simulink model "SimulinkAnalysisofCheetahTail"  (R2022a)
settings: Solver=ode4  StartTime=0.0  StopTime=1.5  FixedStep=0.001  RelTol=1e-3
undefined symbols (not defined in the file): B_cg_H, B_con_H, B_con_L, bar_len, cd_table, Cf, cl_table, g, gear_ratio, int_point_bar, int_point_tail, ITail, M_add, M_cg_H, M_cg_L, M_cg_W, Mb, Mm, Mt, psi3, rho, T_cg_H, T_fur_gap, T_length, T_width_major, T_width_minor, th2_initial, torque_constant, uncertainty_Forces, uncertainty_Position, Vf, windspeed
(part 2 of 21)

== matlab function SimulinkAnalysisofCheetahTail/Model/CoriolusMatrix ==
  data: B_cg_H parameter; B_con_H parameter; B_con_L parameter; ITail parameter; M_cg_H parameter; M_cg_L parameter; M_cg_W parameter; Mb parameter; Mm parameter; Mt parameter; T_cg_H parameter; C output; q input; dq input
function C = CoriolusMatrix(B_cg_H,B_con_H,B_con_L,ITail,M_cg_H,M_cg_L,M_cg_W,Mb,Mm,Mt,T_cg_H,q,dq)
%#codegen
[x,y,z,phi1,th1,psi1,phi2,th2] = deal(q(1),q(2),q(3),q(4),q(5),q(6),q(7),q(8));
[dx,dy,dz,dphi1,dth1,dpsi1,dphi2,dth2] = deal(dq(1),dq(2),dq(3),dq(4),dq(5),dq(6),dq(7),dq(8));
%    This function was generated by the Symbolic Math Toolbox version 9.0.
%    26-Jan-2022 10:41:54

t2 = cos(phi1);
t3 = cos(phi2);
t4 = cos(psi1);
t5 = cos(th1);
t6 = cos(th2);
t7 = sin(phi1);
t8 = sin(phi2);
t9 = sin(psi1);
t10 = sin(th1);
t11 = sin(th2);
t12 = M_cg_L+x;
t13 = M_cg_W+y;
t14 = M_cg_H+z;
t15 = B_cg_H.^2;
t1314 = dphi1.*1.8563e-7;
t1336 = dphi1.*2.3495e-8;
t16 = t2.^2;
t17 = t4.^2;
t18 = t5.^2;
t19 = t7.^2;
t20 = t9.^2;
t21 = t10.^2;
t22 = B_con_L.*t5;
t23 = B_con_L.*t10;
t24 = dth1.*t2;
t25 = dx.*t5;
t26 = dth1.*t7;
t27 = dpsi1.*t10;
t28 = dx.*t10;
t29 = t2.*t3;
t30 = t2.*t4;
t31 = t5.*t6;
t32 = t2.*t8;
t33 = t2.*t9;
t34 = t4.*t7;
t35 = t5.*t11;
t36 = t6.*t10;
t37 = t7.*t8;
t38 = t7.*t9;
t39 = t10.*t11;
t40 = B_con_H.*t2.*t5;
t42 = t5.*t12;
t43 = B_con_H.*t2.*t10;
t44 = B_con_H.*t5.*t7;
t47 = t10.*t12;
t48 = Mb.*t5.*t10;
t49 = Mm.*t5.*t10;
t50 = Mt.*t5.*t10;
t51 = B_con_H.*t7.*t10;
t53 = dphi1.*t2.*t5;
t54 = dpsi1.*t2.*t5;
t56 = dy.*t2.*t5;
t57 = dz.*t2.*t5;
t58 = dpsi1.*t4.*t5;
t60 = dphi1.*t5.*t7;
t61 = dpsi1.*t5.*t7;
t63 = dy.*t5.*t7;
t64 = dz.*t2.*t10;
t65 = dz.*t5.*t7;
t66 = dpsi1.*t5.*t9;
t67 = dth1.*t4.*t10;
t71 = dy.*t7.*t10;
t72 = dth1.*t9.*t10;
t93 = t3.*t5.*t7;
t94 = t3.*t6.*t7;
t107 = t3.*t7.*t10;
t117 = t2.*t5.*t13;
t121 = t2.*t5.*t14;
t127 = t2.*t10.*t13;
t128 = t5.*t7.*t13;
t131 = t2.*t10.*t14;
t132 = t5.*t7.*t14;
t139 = t7.*t10.*t13;
t140 = t7.*t10.*t14;
t1196 = t5.*7.84867146e-3;
t1215 = t2.*1.19846373e-3;
t1223 = t7.*1.19846373e-3;
t1233 = t2.*3.949132625e-3;
t1234 = t7.*3.949132625e-3;
t1252 = t2.*1.0208097e-4;
t1253 = t7.*1.0208097e-4;
t1315 = t5.*t7.*(-1.19846373e-3);
t1343 = t2.*1.8563e-7;
t1344 = t2.*3.7126e-7;
t1345 = t5.*1.8563e-7;
t1346 = t7.*1.8563e-7;
t1347 = t10.*1.8563e-7;
t1348 = t7.*4.699e-8;
t1353 = t5.*t7.*(-1.0208097e-4);
t1370 = t2.*2.3495e-8;
t1371 = t5.*2.3495e-8;
t1374 = t7.*2.3495e-8;
t1375 = t10.*2.3495e-8;
t1391 = t2.*t5.*4.699e-8;
t1393 = t5.*t7.*3.7126e-7;
t1433 = t2.*t10.*(-3.7126e-7);
t41 = t4.*t22;
t45 = t4.*t23;
t46 = t9.*t22;
t52 = t9.*t23;
t55 = dphi1+t27;
t59 = t4.*t25;
t62 = t10.*t24;
t68 = t4.*t28;
t69 = t9.*t25;
t70 = t10.*t26;
t73 = t9.*t28;
t74 = t2.*t39;
t75 = t3.*t39;
t76 = t8.*t35;
t77 = t8.*t36;
t78 = t4.*t39;
t79 = t9.*t35;
t80 = t9.*t36;
t81 = t10.*t37;
t82 = t10.*t38;
t83 = t11.*t38;
t84 = t8.*t39;
t85 = t9.*t39;
t86 = t5.*t29;
t87 = t6.*t29;
t88 = t2.*t31;
t89 = t3.*t31;
t90 = t4.*t31;
t91 = t10.*t29;
t92 = t5.*t32;
t95 = t10.*t30;
t96 = t11.*t30;
t97 = t6.*t34;
t98 = t2.*t35;
t99 = t2.*t36;
t100 = t3.*t35;
t101 = t3.*t36;
t102 = t8.*t31;
t103 = t4.*t35;
t104 = t4.*t36;
t105 = t9.*t31;
t106 = t10.*t32;
t108 = t5.*t37;
t109 = t6.*t37;
t110 = t10.*t33;
t111 = t10.*t34;
t112 = t11.*t33;
t113 = t11.*t34;
t114 = t6.*t38;
t115 = B_con_H.*t5.*t30;
t116 = t4.*t42;
t119 = B_con_H.*t5.*t33;
t120 = B_con_H.*t5.*t34;
t122 = t4.*t47;
t123 = t9.*t42;
t124 = t2.*t48;
t125 = t2.*t49;
t126 = t2.*t50;
t130 = B_con_H.*t5.*t38;
t133 = t4.*t5.*t24;
t134 = dz.*t5.*t30;
t135 = t9.*t47;
t136 = t7.*t48;
t137 = t7.*t49;
t138 = t7.*t50;
t141 = t5.*t9.*t24;
t142 = t4.*t5.*t26;
t143 = dy.*t5.*t34;
t144 = dz.*t5.*t33;
t146 = dphi1.*t7.*t31;
t147 = dth2.*t7.*t31;
t148 = -t43;
t149 = -t44;
t150 = t5.*t9.*t26;
t151 = dy.*t5.*t38;
t152 = dphi1.*t7.*t35;
t153 = -t48;
t154 = -t49;
t155 = -t50;
t156 = -t51;
t157 = dphi1.*t7.*t39;
t158 = t26.*t39;
t159 = -t61;
t160 = -t63;
t161 = -t64;
t164 = -t72;
t165 = Mb.*t2.*t18;
t166 = Mm.*t2.*t18;
t167 = Mt.*t2.*t18;
t168 = Mb.*t2.*t21;
t169 = Mb.*t7.*t18;
t170 = Mm.*t2.*t21;
t171 = Mm.*t7.*t18;
t172 = Mt.*t2.*t21;
t173 = Mt.*t7.*t18;
t174 = Mb.*t7.*t21;
t175 = Mm.*t7.*t21;
t176 = Mt.*t7.*t21;
t182 = t29.*t31;
t183 = t30.*t31;
t186 = t5.*t8.*t30;
t187 = t3.*t5.*t34;
t188 = t29.*t35;
t189 = t29.*t36;
t190 = t31.*t32;
t192 = t30.*t35;
t193 = t30.*t36;
t194 = t31.*t33;
t200 = t3.*t5.*t38;
t201 = t5.*t8.*t34;
t202 = t29.*t39;
t203 = t32.*t35;
t204 = t32.*t36;
t206 = t31.*t37;
t207 = t30.*t39;
t208 = t33.*t35;
t209 = t33.*t36;
t219 = t32.*t39;
t220 = t36.*t37;
t221 = t33.*t39;
t222 = t34.*t39;
t230 = t38.*t39;
t234 = t5.*t13.*t30;
t235 = t5.*t14.*t30;
t236 = t5.*t13.*t33;
t237 = t5.*t13.*t34;
t239 = t5.*t14.*t33;
t240 = t5.*t14.*t34;
t241 = Mb.*t16.*t18;
t242 = Mm.*t16.*t18;
t243 = Mt.*t16.*t18;
t248 = t5.*t13.*t38;
t250 = t5.*t14.*t38;
t251 = Mb.*t18.*t19;
t252 = Mm.*t18.*t19;
t253 = Mt.*t18.*t19;
t255 = -t117;
t261 = dphi1.*t34.*t35;
t264 = -t127;
t265 = -t128;
t268 = -t131;
t269 = -t132;
t271 = dphi1.*t35.*t37;
t272 = dth2.*t35.*t37;
t273 = dphi1.*t35.*t38;
t275 = -t140;
t283 = t16.*t48;
t284 = t17.*t48;
t285 = t16.*t49;
t286 = t16.*t50;
t287 = t17.*t49;
t288 = t17.*t50;
t289 = t19.*t48;
t290 = t20.*t48;
t291 = t19.*t49;
t292 = t19.*t50;
t293 = t20.*t49;
t294 = t20.*t50;
t304 = t26+t54;
t377 = t66+t67;
t378 = t32+t94;
t391 = t93.*(2.7e+1./1.0e+2);
t395 = t107.*(2.7e+1./1.0e+2);
t524 = t117+t132;
t527 = t127+t140;
t1254 = -t1223;
t1258 = t26.*1.19846373e-3;
t1259 = t24.*3.949132625e-3;
t1268 = -t1253;
t1269 = t5.*t1215;
t1273 = t10.*t1215;
t1274 = t5.*t1223;
t1283 = t5.*t1233;
t1290 = t5.*t1234;
t1300 = t10.*t1234;
t1301 = t24.*1.0208097e-4;
t1305 = t26.*1.0208097e-4;
t1310 = t10.*t1253;
t1318 = t54.*1.19846373e-3;
t1321 = t61.*3.949132625e-3;
t1322 = t5.*t1252;
t1326 = t10.*t1252;
t1327 = t5.*t1253;
t1337 = t54.*1.0208097e-4;
t1338 = t61.*1.0208097e-4;
t1359 = t27.*1.8563e-7;
t1369 = -t1345;
t1373 = -t1348;
t1387 = t27.*2.3495e-8;
t1392 = t10.*t1344;
t1397 = t10.*t1348;
t1398 = -t1374;
t1401 = -t1375;
t2597 = t1215+t1253;
t2617 = t1234+t1252;
t2839 = -t2.*t10.*(t1223-t1252);
t2840 = -t5.*t7.*(t1223-t1252);
t2910 = t1346+t1370;
t2913 = t5.*t7.*(t1223-t1252);
t118 = B_con_H.*t95;
t129 = B_con_H.*t110;
t145 = dphi1.*t98;
t162 = -t69;
t163 = -t70;
t177 = -t74;
t178 = -t81;
t179 = -t82;
t180 = -t84;
t181 = t4.*t86;
t184 = t4.*t89;
t185 = t9.*t86;
t191 = t7.*t89;
t195 = t4.*t100;
t196 = t4.*t101;
t197 = t9.*t89;
t198 = t8.*t90;
t199 = t9.*t92;
t205 = t7.*t101;
t210 = t4.*t75;
t211 = t3.*t79;
t212 = t3.*t80;
t213 = t4.*t76;
t214 = t9.*t102;
t215 = -t87;
t216 = t8.*t111;
t217 = t9.*t108;
t218 = -t88;
t223 = t9.*t75;
t224 = t8.*t78;
t225 = t9.*t76;
t226 = -t95;
t227 = t9.*t81;
t228 = -t103;
t229 = -t105;
t231 = t9.*t84;
t232 = -t109;
t233 = -t114;
t238 = t14.*t95;
t244 = t7.*t124;
t245 = t7.*t125;
t246 = t7.*t126;
t247 = t13.*t111;
t249 = t14.*t110;
t254 = T_cg_H.*t7.*t100;
t257 = -t120;
t258 = t13.*t82;
t259 = dphi1.*t7.*t100;
t260 = dth2.*t7.*t100;
t262 = t26.*t103;
t263 = -t123;
t267 = -t130;
t270 = -t133;
t274 = t26.*t79;
t276 = -t143;
t277 = -t151;
t278 = -t157;
t279 = -t158;
t280 = t7.*t165;
t281 = t7.*t166;
t282 = t7.*t167;
t295 = -t165;
t296 = -t166;
t297 = -t167;
t298 = -t169;
t299 = -t171;
t300 = -t173;
t305 = t29.*t90;
t306 = t29.*t103;
t307 = t29.*t104;
t308 = t29.*t105;
t309 = t30.*t102;
t310 = t34.*t89;
t314 = t29.*t79;
t315 = t29.*t80;
t316 = t32.*t105;
t317 = t38.*t89;
t318 = t34.*t102;
t319 = -t182;
t320 = -t183;
t321 = t37.*t105;
t322 = -t190;
t323 = -t194;
t326 = -t202;
t327 = -t206;
t328 = -t207;
t331 = -t219;
t332 = -t220;
t333 = -t221;
t336 = -t230;
t338 = -t234;
t339 = t20.*t169;
t340 = t20.*t171;
t341 = t20.*t173;
t342 = -t236;
t343 = -t237;
t345 = -t240;
t346 = -t241;
t347 = -t242;
t348 = -t243;
t349 = -t248;
t351 = -t250;
t352 = -t271;
t353 = -t272;
t354 = -t273;
t361 = t17.*t165;
t362 = t17.*t166;
t363 = t17.*t167;
t364 = t20.*t165;
t365 = t17.*t169;
t366 = t20.*t166;
t367 = t17.*t171;
t368 = t20.*t167;
t369 = t17.*t173;
t370 = t75.*(2.7e+1./1.0e+2);
t371 = t76.*(2.7e+1./1.0e+2);
t372 = t77.*(2.7e+1./1.0e+2);
t373 = t81.*(2.7e+1./1.0e+2);
t374 = t84.*(2.7e+1./1.0e+2);
t375 = B_cg_H.*Mb.*t7.*t10.*t100;
t376 = t60+t62;
t379 = t35+t99;
t380 = t36+t98;
t381 = t33+t111;
t382 = t34+t110;
t383 = t24+t159;
t388 = t86.*(2.7e+1./1.0e+2);
t389 = t89.*(2.7e+1./1.0e+2);
t390 = t92.*(2.7e+1./1.0e+2);
t392 = t100.*(2.7e+1./1.0e+2);
t393 = t101.*(2.7e+1./1.0e+2);
t394 = t106.*(2.7e+1./1.0e+2);
t396 = t108.*(2.7e+1./1.0e+2);
t401 = B_cg_H.*t3.*t11.*t251;
t415 = t58+t164;
t422 = B_cg_H.*t11.*t29.*t169;
t423 = t182.*(2.7e+1./1.0e+2);
t425 = t186.*(2.7e+1./1.0e+2);
t426 = t187.*(2.7e+1./1.0e+2);
t427 = t188.*(2.7e+1./1.0e+2);
t428 = t189.*(2.7e+1./1.0e+2);
t429 = t190.*(2.7e+1./1.0e+2);
t437 = t200.*(2.7e+1./1.0e+2);
t438 = t201.*(2.7e+1./1.0e+2);
t441 = t202.*(2.7e+1./1.0e+2);
t442 = t203.*(2.7e+1./1.0e+2);
t443 = t204.*(2.7e+1./1.0e+2);
t446 = t206.*(2.7e+1./1.0e+2);
t475 = dphi1.*t5.*t378;
t477 = dphi1.*t10.*t378;
t481 = t93+t190;
t485 = t101+t188;
t487 = t104+t192;
t495 = t77+t203;
t496 = t80+t208;
t506 = t112+t222;
t585 = dphi1.*t524;
t595 = t121+t265;
t650 = Mm.*t5.*t524;
t651 = t234+t240;
t655 = Mm.*t10.*t527;
t657 = t236+t250;
t753 = t7.*t11.*t18.*t378;
t756 = Mm.*t2.*t10.*t524;
t759 = Mm.*t2.*t5.*t527;
t760 = Mm.*t7.*t10.*t524;
t762 = Mm.*t5.*t7.*t527;
t818 = t79+t97+t209;
t819 = t76+t107+t204;
t855 = t42+t139+t268;
t1149 = Mm.*t524.*t527;
t1316 = -t1301;
t1317 = -t1305;
t1350 = -t1321;
t1364 = -t1337;
t2653 = t1252+t1254;
t2660 = t1233+t1268;
t2789 = t5.*t7.*t2617;
t2801 = t1315+t1322;
t2809 = t153+t154+t155+t284+t287+t288+t290+t293+t294;
t2810 = t1283+t1353;
t2815 = t2.*t5.*t2597;
t2911 = t7.*(t1322-t5.*t7.*1.19846373e-3);
t2912 = t2.*(t1283+t5.*t1268);
t2948 = t1343+t1398;
t3030 = t5.*t2910;
t3932 = t1269+t1327+t1347;
t3944 = t1273+t1310+t1369;
t3955 = t1300+t1326+t1371;
t3965 = t1290+t1322+t1401;
t256 = -t118;
t266 = -t129;
t301 = t244.*2.0;
t302 = t245.*2.0;
t303 = t246.*2.0;
t311 = t280.*2.0;
t312 = t281.*2.0;
t313 = t282.*2.0;
t324 = -t195;
t325 = -t197;
t329 = -t214;
t330 = -t216;
t334 = -t224;
t335 = t9.*t178;
t337 = t9.*t180;
C = ft_1({B_cg_H,B_con_H,ITail,Mb,Mm,Mt,T_cg_H,dphi1,dphi2,dpsi1,dth1,dth2,dx,dy,dz,t10,t100,t102,t103,t105,t106,t108,t11,t113,t1149,t115,t116,t119,t1196,t120,t1215,t122,t1223,t123,t1234,t124,t125,t1252,t1253,t1258,t1259,t126,t1268,t1283,t13,t130,t1301,t1305,t1314,t1316,t1317,t1318,t1322,t1336,t1337,t1338,t134,t1343,t1344,t1345,t1348,t135,t1350,t1359,t136,t1364,t137,t1370,t1371,t1373,t1374,t138,t1387,t1391,t1393,t1397,t14,t141,t142,t1433,t144,t145,t146,t147,t148,t149,t15,t150,t152,t156,t160,t161,t162,t163,t165,t166,t167,t168,t169,t170,t171,t172,t173,t174,t175,t176,t177,t178,t179,t180,t181,t184,t185,t186,t187,t189,t191,t193,t195,t196,t197,t198,t199,t2,t200,t201,t205,t210,t211,t212,t213,t214,t215,t216,t217,t218,t22,t221,t223,t224,t225,t226,t227,t228,t229,t23,t231,t232,t233,t235,t239,t24,t241,t242,t243,t244,t245,t246,t247,t249,t25,t251,t252,t253,t254,t255,t256,t257,t258,t259,t2597,t26,t260,t261,t2617,t262,t263,t264,t266,t2660,t267,t269,t27,t270,t271,t273,t274,t275,t276,t277,t278,t2789,t279,t28,t280,t2809,t281,t2815,t282,t283,t2839,t284,t285,t286,t287,t288,t289,t29,t290,t291,t2911,t2912,t2913,t292,t293,t294,t2948,t295,t296,t297,t298,t299,t3,t30,t300,t301,t302,t303,t3030,t304,t305,t306,t307,t308,t309,t31,t310,t311,t312,t313,t314,t315,t316,t317,t318,t319,t320,t322,t323,t324,t325,t326,t327,t328,t329,t33,t330,t331,t332,t333,t334,t335,t336,t337,t338,t339,t34,t340,t341,t342,t343,t345,t346,t347,t348,t349,t35,t351,t352,t353,t354,t361,t362,t363,t364,t365,t366,t367,t368,t369,t37,t370,t371,t372,t373,t374,t375,t376,t377,t378,t379,t38,t380,t381,t382,t383,t388,t389,t39,t390,t391,t392,t393,t3932,t394,t3944,t395,t3955,t396,t3965,t4,t40,t401,t41,t415,t423,t425,t426,t427,t428,t429,t437,t438,t44,t441,t442,t443,t446,t45,t46,t47,t475,t477,t48,t481,t485,t487,t49,t495,t496,t5,t50,t506,t51,t52,t524,t527,t53,t54,t55,t56,t57,t585,t59,t595,t6,t61,t65,t650,t651,t655,t657,t68,t69,t7,t71,t73,t75,t753,t756,t759,t760,t762,t78,t79,t8,t818,t819,t83,t84,t85,t855,t86,t89,t9,t90,t91,t92,t96,t98});
end
function C = ft_1(ct)
B_cg_H = ct{1};
B_con_H = ct{2};
ITail = ct{3};
Mb = ct{4};
Mm = ct{5};
Mt = ct{6};
T_cg_H = ct{7};
dphi1 = ct{8};
dphi2 = ct{9};
dpsi1 = ct{10};
dth1 = ct{11};
dth2 = ct{12};
dx = ct{13};
dy = ct{14};
dz = ct{15};
t10 = ct{16};
t100 = ct{17};
t102 = ct{18};
t103 = ct{19};
t105 = ct{20};
t106 = ct{21};
t108 = ct{22};
t11 = ct{23};
t113 = ct{24};
t1149 = ct{25};
t115 = ct{26};
t116 = ct{27};
t119 = ct{28};
t1196 = ct{29};
t120 = ct{30};
t1215 = ct{31};
t122 = ct{32};
t1223 = ct{33};
t123 = ct{34};
t1234 = ct{35};
t124 = ct{36};
t125 = ct{37};
t1252 = ct{38};
t1253 = ct{39};
t1258 = ct{40};
t1259 = ct{41};
t126 = ct{42};
t1268 = ct{43};
t1283 = ct{44};
t13 = ct{45};
t130 = ct{46};
t1301 = ct{47};
t1305 = ct{48};
t1314 = ct{49};
t1316 = ct{50};
t1317 = ct{51};
t1318 = ct{52};
t1322 = ct{53};
t1336 = ct{54};
t1337 = ct{55};
t1338 = ct{56};
t134 = ct{57};
t1343 = ct{58};
t1344 = ct{59};
t1345 = ct{60};
t1348 = ct{61};
t135 = ct{62};
t1350 = ct{63};
t1359 = ct{64};
t136 = ct{65};
t1364 = ct{66};
t137 = ct{67};
t1370 = ct{68};
t1371 = ct{69};
t1373 = ct{70};
t1374 = ct{71};
t138 = ct{72};
t1387 = ct{73};
t1391 = ct{74};
t1393 = ct{75};
t1397 = ct{76};
t14 = ct{77};
t141 = ct{78};
t142 = ct{79};
t1433 = ct{80};
t144 = ct{81};
t145 = ct{82};
t146 = ct{83};
t147 = ct{84};
t148 = ct{85};
t149 = ct{86};
t15 = ct{87};
t150 = ct{88};
t152 = ct{89};
t156 = ct{90};
t160 = ct{91};
t161 = ct{92};
t162 = ct{93};
t163 = ct{94};
t165 = ct{95};
t166 = ct{96};
t167 = ct{97};
t168 = ct{98};
t169 = ct{99};
t170 = ct{100};
t171 = ct{101};
t172 = ct{102};
t173 = ct{103};
t174 = ct{104};
t175 = ct{105};
t176 = ct{106};
t177 = ct{107};
t178 = ct{108};
t179 = ct{109};
t180 = ct{110};
t181 = ct{111};
t184 = ct{112};
t185 = ct{113};
t186 = ct{114};
t187 = ct{115};
t189 = ct{116};
t191 = ct{117};
t193 = ct{118};
t195 = ct{119};
t196 = ct{120};
t197 = ct{121};
t198 = ct{122};
t199 = ct{123};
t2 = ct{124};
t200 = ct{125};
t201 = ct{126};
t205 = ct{127};
t210 = ct{128};
t211 = ct{129};
t212 = ct{130};
t213 = ct{131};
t214 = ct{132};
t215 = ct{133};
t216 = ct{134};
t217 = ct{135};
t218 = ct{136};
t22 = ct{137};
t221 = ct{138};
t223 = ct{139};
t224 = ct{140};
t225 = ct{141};
t226 = ct{142};
t227 = ct{143};
t228 = ct{144};
t229 = ct{145};
t23 = ct{146};
t231 = ct{147};
t232 = ct{148};
t233 = ct{149};
t235 = ct{150};
t239 = ct{151};
t24 = ct{152};
t241 = ct{153};
t242 = ct{154};
t243 = ct{155};
t244 = ct{156};
t245 = ct{157};
t246 = ct{158};
t247 = ct{159};
t249 = ct{160};
t25 = ct{161};
t251 = ct{162};
t252 = ct{163};
t253 = ct{164};
t254 = ct{165};
t255 = ct{166};
t256 = ct{167};
t257 = ct{168};
t258 = ct{169};
t259 = ct{170};
t2597 = ct{171};
t26 = ct{172};
t260 = ct{173};
t261 = ct{174};
t2617 = ct{175};
t262 = ct{176};
t263 = ct{177};
t264 = ct{178};
t266 = ct{179};
t2660 = ct{180};
t267 = ct{181};
t269 = ct{182};
t27 = ct{183};
t270 = ct{184};
t271 = ct{185};
t273 = ct{186};
t274 = ct{187};
t275 = ct{188};
t276 = ct{189};
t277 = ct{190};
t278 = ct{191};
t2789 = ct{192};
t279 = ct{193};
t28 = ct{194};
t280 = ct{195};
t2809 = ct{196};
t281 = ct{197};
t2815 = ct{198};
t282 = ct{199};
t283 = ct{200};
t2839 = ct{201};
t284 = ct{202};
t285 = ct{203};
t286 = ct{204};
t287 = ct{205};
t288 = ct{206};
t289 = ct{207};
t29 = ct{208};
t290 = ct{209};
t291 = ct{210};
t2911 = ct{211};
t2912 = ct{212};
t2913 = ct{213};
t292 = ct{214};
t293 = ct{215};
t294 = ct{216};
t2948 = ct{217};
t295 = ct{218};
t296 = ct{219};
t297 = ct{220};
t298 = ct{221};
t299 = ct{222};
t3 = ct{223};
t30 = ct{224};
t300 = ct{225};
t301 = ct{226};
t302 = ct{227};
t303 = ct{228};
t3030 = ct{229};
t304 = ct{230};
t305 = ct{231};
t306 = ct{232};
t307 = ct{233};
t308 = ct{234};
t309 = ct{235};
t31 = ct{236};
t310 = ct{237};
t311 = ct{238};
t312 = ct{239};
t313 = ct{240};
t314 = ct{241};
t315 = ct{242};
t316 = ct{243};
t317 = ct{244};
t318 = ct{245};
t319 = ct{246};
t320 = ct{247};
t322 = ct{248};
t323 = ct{249};
t324 = ct{250};
t325 = ct{251};
t326 = ct{252};
t327 = ct{253};
t328 = ct{254};
t329 = ct{255};
t33 = ct{256};
t330 = ct{257};
t331 = ct{258};
t332 = ct{259};
t333 = ct{260};
t334 = ct{261};
t335 = ct{262};
t336 = ct{263};
t337 = ct{264};
t338 = ct{265};
t339 = ct{266};
t34 = ct{267};
t340 = ct{268};
t341 = ct{269};
t342 = ct{270};
t343 = ct{271};
t345 = ct{272};
t346 = ct{273};
t347 = ct{274};
t348 = ct{275};
t349 = ct{276};
t35 = ct{277};
t351 = ct{278};
t352 = ct{279};
t353 = ct{280};
t354 = ct{281};
t361 = ct{282};
t362 = ct{283};
t363 = ct{284};
t364 = ct{285};
t365 = ct{286};
t366 = ct{287};
t367 = ct{288};
t368 = ct{289};
t369 = ct{290};
t37 = ct{291};
t370 = ct{292};
t371 = ct{293};
t372 = ct{294};
t373 = ct{295};
t374 = ct{296};
t375 = ct{297};
t376 = ct{298};
t377 = ct{299};
t378 = ct{300};
t379 = ct{301};
t38 = ct{302};
t380 = ct{303};
t381 = ct{304};
t382 = ct{305};
t383 = ct{306};
t388 = ct{307};
t389 = ct{308};
t39 = ct{309};
t390 = ct{310};
t391 = ct{311};
t392 = ct{312};
t393 = ct{313};
t3932 = ct{314};
t394 = ct{315};
t3944 = ct{316};
t395 = ct{317};
t3955 = ct{318};
t396 = ct{319};
t3965 = ct{320};
t4 = ct{321};
t40 = ct{322};
t401 = ct{323};
t41 = ct{324};
t415 = ct{325};
t423 = ct{326};
t425 = ct{327};
t426 = ct{328};
t427 = ct{329};
t428 = ct{330};
t429 = ct{331};
t437 = ct{332};
t438 = ct{333};
t44 = ct{334};
t441 = ct{335};
t442 = ct{336};
t443 = ct{337};
t446 = ct{338};
t45 = ct{339};
t46 = ct{340};
t47 = ct{341};
t475 = ct{342};
t477 = ct{343};
t48 = ct{344};
t481 = ct{345};
t485 = ct{346};
t487 = ct{347};
t49 = ct{348};
t495 = ct{349};
t496 = ct{350};
t5 = ct{351};
t50 = ct{352};
t506 = ct{353};
t51 = ct{354};
t52 = ct{355};
t524 = ct{356};
t527 = ct{357};
t53 = ct{358};
t54 = ct{359};
t55 = ct{360};
t56 = ct{361};
t57 = ct{362};
t585 = ct{363};
t59 = ct{364};
t595 = ct{365};
t6 = ct{366};
t61 = ct{367};
t65 = ct{368};
t650 = ct{369};
t651 = ct{370};
t655 = ct{371};
t657 = ct{372};
t68 = ct{373};
t69 = ct{374};
t7 = ct{375};
t71 = ct{376};
t73 = ct{377};
t75 = ct{378};
t753 = ct{379};
t756 = ct{380};
t759 = ct{381};
t760 = ct{382};
t762 = ct{383};
t78 = ct{384};
t79 = ct{385};
t8 = ct{386};
t818 = ct{387};
t819 = ct{388};
t83 = ct{389};
t84 = ct{390};
t85 = ct{391};
t855 = ct{392};
t86 = ct{393};
t89 = ct{394};
t9 = ct{395};
t90 = ct{396};
t91 = ct{397};
t92 = ct{398};
t96 = ct{399};
t98 = ct{400};
t344 = t14.*t226;
t350 = -t249;
t355 = -t280;
t357 = -t281;
t359 = -t282;
t384 = -t305;
t385 = t29.*t229;
t386 = -t318;
t387 = t37.*t229;
t397 = -t373;
t398 = -t374;
t399 = B_con_H.*t381;
t400 = B_con_H.*t382;
t402 = dth1.*t379;
t403 = dth1.*t380;
t404 = dth2.*t379;
t405 = dth2.*t380;
t406 = dphi1.*t381;
t407 = dphi1.*t382;
t408 = dpsi1.*t381;
t409 = dpsi1.*t382;
t410 = dy.*t381;
t411 = dy.*t382;
t412 = dz.*t381;
t413 = dz.*t382;
t414 = t53+t163;
t416 = t29+t232;
t417 = t37+t215;
t418 = t31+t177;
t419 = t39+t218;
t420 = t30+t179;
t421 = t38+t226;
t424 = t184.*(2.7e+1./1.0e+2);
t430 = t191.*(2.7e+1./1.0e+2);
t431 = t195.*(2.7e+1./1.0e+2);
t432 = t196.*(2.7e+1./1.0e+2);
t433 = t197.*(2.7e+1./1.0e+2);
t434 = t198.*(2.7e+1./1.0e+2);
t435 = t380.^2;
t436 = t199.*(2.7e+1./1.0e+2);
t439 = t381.^2;
t440 = t382.^2;
t444 = t7.*t392;
t445 = t205.*(2.7e+1./1.0e+2);
t447 = t210.*(2.7e+1./1.0e+2);
t448 = t211.*(2.7e+1./1.0e+2);
t449 = t212.*(2.7e+1./1.0e+2);
t450 = t213.*(2.7e+1./1.0e+2);
t451 = t214.*(2.7e+1./1.0e+2);
t452 = t216.*(2.7e+1./1.0e+2);
t453 = t217.*(2.7e+1./1.0e+2);
t454 = t223.*(2.7e+1./1.0e+2);
t455 = t224.*(2.7e+1./1.0e+2);
t456 = t225.*(2.7e+1./1.0e+2);
t457 = t227.*(2.7e+1./1.0e+2);
t458 = t231.*(2.7e+1./1.0e+2);
t459 = t3.*t381;
t460 = t3.*t382;
t461 = t6.*t382;
t462 = -t423;
t463 = t8.*t381;
t464 = t8.*t382;
t465 = t11.*t382;
t468 = -t441;
t469 = -t446;
t479 = dth2.*t6.*t381;
t480 = t92+t191;
t491 = -t401;
t492 = t106+t205;
t513 = t305.*(2.7e+1./1.0e+2);
t514 = B_cg_H.*t11.*t29.*t298;
t515 = t306.*(2.7e+1./1.0e+2);
t516 = t307.*(2.7e+1./1.0e+2);
t517 = t308.*(2.7e+1./1.0e+2);
t518 = t309.*(2.7e+1./1.0e+2);
t519 = t310.*(2.7e+1./1.0e+2);
t520 = t314.*(2.7e+1./1.0e+2);
t521 = t315.*(2.7e+1./1.0e+2);
t522 = t316.*(2.7e+1./1.0e+2);
t523 = t317.*(2.7e+1./1.0e+2);
t528 = t13.*t381;
t529 = t13.*t382;
t530 = t14.*t381;
t531 = t14.*t382;
t555 = t86+t327;
t556 = t108+t319;
t557 = t75+t319;
t558 = t89+t326;
t559 = t78+t320;
t560 = t90+t328;
t564 = t91+t332;
t566 = t84+t322;
t567 = t102+t331;
t568 = t85+t323;
t569 = t105+t333;
t575 = t96+t336;
t588 = T_cg_H.*t485;
t589 = Mb.*t4.*t5.*t381;
t590 = Mb.*t4.*t5.*t382;
t591 = Mm.*t4.*t5.*t381;
t592 = Mm.*t4.*t5.*t382;
t593 = Mt.*t4.*t5.*t381;
t594 = Mt.*t4.*t5.*t382;
t598 = dphi1.*t481;
t600 = dphi2.*t485;
t601 = dth2.*t485;
t602 = dpsi1.*t487;
t603 = dth1.*t487;
t604 = Mb.*t4.*t10.*t381;
t605 = Mb.*t5.*t9.*t381;
t606 = Mb.*t5.*t9.*t382;
t607 = Mm.*t4.*t10.*t381;
t608 = Mm.*t5.*t9.*t381;
t609 = Mm.*t5.*t9.*t382;
t610 = Mt.*t4.*t10.*t381;
t611 = Mt.*t5.*t9.*t381;
t612 = Mt.*t5.*t9.*t382;
t615 = T_cg_H.*t495;
t616 = Mb.*t9.*t10.*t382;
t617 = Mm.*t9.*t10.*t382;
t618 = Mt.*t9.*t10.*t382;
t628 = dphi2.*t495;
t629 = dth2.*t495;
t630 = dpsi1.*t496;
t631 = dth1.*t496;
t656 = -t585;
t658 = Mb.*t5.*t30.*t381;
t659 = Mm.*t5.*t30.*t381;
t660 = Mt.*t5.*t30.*t381;
t662 = dth1.*t4.*t485;
t663 = dth2.*t3.*t487;
t664 = Mb.*t5.*t33.*t382;
t665 = Mb.*t5.*t34.*t381;
t666 = Mm.*t5.*t33.*t382;
t667 = Mm.*t5.*t34.*t381;
t668 = Mt.*t5.*t33.*t382;
t669 = Mt.*t5.*t34.*t381;
t673 = t186+t310;
t674 = dth1.*t9.*t485;
t675 = t196+t306;
t676 = dth2.*t8.*t487;
t677 = Mb.*t5.*t38.*t382;
t678 = Mm.*t5.*t38.*t382;
t679 = Mt.*t5.*t38.*t382;
t693 = dth1.*t4.*t495;
t694 = dth2.*t3.*t496;
t698 = t199+t317;
t699 = dth2.*t3.*t506;
t720 = dth1.*t9.*t495;
t721 = t212+t314;
t722 = dth2.*t8.*t496;
t724 = dth2.*t8.*t506;
t744 = B_cg_H.*Mb.*t10.*t495;
t745 = t7.*t100.*t380;
t754 = B_cg_H.*Mb.*t5.*t485;
t755 = t2.*t650;
t757 = t7.*t650;
t761 = -t650;
t764 = Mm.*t10.*t595;
t820 = t7.*t35.*t495;
t837 = B_cg_H.*Mb.*t2.*t10.*t485;
t839 = -t753;
t840 = B_cg_H.*Mb.*t195.*t381;
t841 = B_cg_H.*Mb.*t2.*t5.*t495;
t842 = B_cg_H.*Mb.*t7.*t10.*t485;
t843 = B_cg_H.*Mb.*t5.*t7.*t495;
t847 = Mm.*t2.*t5.*t595;
t849 = Mm.*t5.*t7.*t595;
t850 = -t756;
t852 = t47+t595;
t854 = -t759;
t865 = t753./2.0;
t869 = t103+t193+t233;
t870 = t100+t178+t189;
t871 = t180+t481;
t873 = t113+t221+t229;
t899 = T_cg_H.*t819;
t901 = dphi2.*t819;
t902 = dth1.*t819;
t904 = Mm.*t5.*t9.*t657;
t905 = dth1.*t855;
t911 = t145+t147+t279;
t914 = Mm.*t4.*t5.*t651;
t920 = Mb.*t381.*t382;
t921 = Mm.*t381.*t382;
t922 = Mt.*t381.*t382;
t927 = dth2.*t3.*t818;
t934 = dth2.*t8.*t818;
t947 = t5.*t378.*t380;
t948 = B_cg_H.*Mb.*t10.*t819;
t950 = t10.*t378.*t380;
t952 = Mm.*t5.*t855;
t983 = Mb.*t7.*t15.*t100.*t485;
t987 = t380.*t495;
t995 = t7.*t35.*t819;
t1005 = Mm.*t2.*t10.*t855;
t1007 = t122+t235+t343;
t1008 = Mm.*t7.*t10.*t855;
t1010 = B_cg_H.*Mb.*t2.*t5.*t819;
t1012 = B_cg_H.*Mb.*t5.*t7.*t819;
t1013 = t135+t239+t349;
t1131 = t485.*t495;
t1151 = Mm.*t381.*t651;
t1152 = Mm.*t382.*t657;
t1185 = t380.*t819;
t1186 = -t1149;
t1320 = t485.*t819;
t1384 = Mm.*t527.*t855;
t1455 = Mm.*t595.*t855;
t1692 = t753.*3.36554e-3;
t1784 = t753.*9.53094055e-4;
t1810 = t753.*3.372786875e-3;
t2819 = t7.*t10.*t2660;
t2842 = t2.*t5.*t2660;
t2844 = -t2789;
t2857 = dx.*t2809;
t2879 = -t2815;
t2977 = -t2911;
t3052 = t10.*t2948;
t3202 = t168+t170+t172+t361+t362+t363+t364+t366+t368;
t3209 = t174+t175+t176+t339+t340+t341+t365+t367+t369;
t3982 = t2.*t3932;
t3998 = t7.*t3944;
t4003 = t2.*t3955;
t4014 = t7.*t3965;
t4597 = t1258+t1314+t1316+t1318+t1338+t1359;
t4603 = t1259+t1317+t1336+t1350+t1364+t1387;
t356 = -t311;
t358 = -t312;
t360 = -t313;
t466 = -t431;
t467 = -t433;
t470 = -t451;
t471 = -t452;
t472 = -t455;
t473 = -t457;
t474 = -t458;
t476 = t3.*t405;
t478 = t6.*t406;
t482 = B_con_H.*t420;
t483 = B_con_H.*t421;
t484 = -t400;
t486 = t8.*t405;
t488 = t11.*t406;
t489 = t11.*t407;
t490 = t11.*t408;
t493 = dth1.*t418;
t494 = dth2.*t419;
t497 = dphi1.*t420;
t498 = dphi1.*t421;
t499 = dpsi1.*t420;
t500 = dpsi1.*t421;
t501 = dy.*t420;
t502 = dy.*t421;
t503 = dz.*t420;
t504 = dz.*t421;
t505 = -t413;
t507 = Mb.*t439;
t508 = Mb.*t440;
t509 = Mm.*t439;
t510 = Mm.*t440;
t511 = Mt.*t439;
t512 = Mt.*t440;
t525 = t420.^2;
t526 = t421.^2;
t532 = t3.*t435;
t533 = t8.*t435;
t534 = t6.*t459;
t535 = t6.*t460;
t536 = -t513;
t537 = t11.*t460;
t538 = t6.*t463;
t539 = t8.*t461;
t540 = -t517;
t541 = t11.*t464;
t542 = t3.*t420;
t543 = t3.*t421;
t544 = t6.*t421;
t545 = t8.*t420;
t546 = t8.*t421;
t547 = t11.*t421;
t548 = dphi1.*t5.*t416;
t549 = dphi1.*t5.*t417;
t551 = dth2.*t3.*t418;
t554 = dth2.*t6.*t420;
t586 = B_cg_H.*t480;
t587 = T_cg_H.*t480;
t596 = B_cg_H.*t492;
t597 = dphi1.*t480;
t599 = dphi2.*t480;
t613 = T_cg_H.*t11.*t459;
t614 = T_cg_H.*t492;
t620 = dth1.*t492;
t621 = t13.*t420;
t622 = t13.*t421;
t623 = -t529;
t624 = t14.*t420;
t625 = t14.*t421;
t626 = -t530;
t627 = -t531;
t632 = B_cg_H.*t601;
t661 = dth1.*t4.*t480;
t670 = B_cg_H.*t556;
t672 = dth1.*t9.*t480;
t680 = T_cg_H.*t555;
t681 = T_cg_H.*t556;
t682 = T_cg_H.*t557;
t683 = T_cg_H.*t558;
t684 = Mb.*t4.*t5.*t420;
t685 = Mb.*t4.*t5.*t421;
t686 = -t589;
t687 = Mm.*t4.*t5.*t420;
t688 = Mm.*t4.*t5.*t421;
t689 = -t591;
t690 = Mt.*t4.*t5.*t420;
t691 = Mt.*t4.*t5.*t421;
t692 = -t593;
t696 = dphi1.*t555;
t697 = dphi2.*t555;
t700 = dth1.*t558;
t701 = dth1.*t559;
t702 = dth1.*t560;
t703 = -t603;
t704 = dth2.*t559;
t705 = Mb.*t4.*t10.*t421;
t706 = Mb.*t5.*t9.*t420;
t707 = Mb.*t5.*t9.*t421;
t708 = -t604;
t709 = -t606;
t710 = Mm.*t4.*t10.*t421;
t711 = Mm.*t5.*t9.*t420;
t712 = Mm.*t5.*t9.*t421;
t713 = -t607;
t714 = -t609;
t715 = Mt.*t4.*t10.*t421;
t716 = Mt.*t5.*t9.*t420;
t717 = Mt.*t5.*t9.*t421;
t718 = -t610;
t719 = -t612;
t725 = Mb.*t9.*t10.*t420;
t726 = -t616;
t727 = Mm.*t9.*t10.*t420;
t728 = -t617;
t729 = Mt.*t9.*t10.*t420;
t730 = -t618;
t733 = dphi1.*t564;
t734 = dth1.*t564;
t738 = dth1.*t567;
t739 = dth2.*t566;
t740 = dth2.*t567;
t741 = dth1.*t568;
t742 = dth1.*t569;
t743 = dth2.*t568;
t749 = t459.*(2.7e+1./1.0e+2);
t750 = t460.*(2.7e+1./1.0e+2);
t751 = t463.*(2.7e+1./1.0e+2);
t752 = t464.*(2.7e+1./1.0e+2);
t758 = t745.*2.0;
t763 = B_cg_H.*t673;
t765 = T_cg_H.*t673;
t766 = T_cg_H.*t675;
t767 = B_cg_H.*t698;
t768 = dphi1.*t673;
t769 = T_cg_H.*t698;
t770 = T_cg_H.*t721;
t771 = dphi1.*t698;
t772 = Mb.*t5.*t30.*t421;
t773 = -t658;
t774 = Mm.*t5.*t30.*t421;
t775 = -t659;
t776 = Mt.*t5.*t30.*t421;
t777 = -t660;
t778 = dth1.*t4.*t555;
t780 = Mb.*t5.*t33.*t420;
t781 = Mb.*t5.*t34.*t421;
t782 = -t664;
t783 = -t665;
t784 = Mm.*t5.*t33.*t420;
t785 = Mm.*t5.*t34.*t421;
t786 = -t666;
t787 = -t667;
t788 = Mt.*t5.*t33.*t420;
t789 = Mt.*t5.*t34.*t421;
t790 = -t668;
t791 = -t669;
t793 = dth1.*t9.*t555;
t794 = t181+t386;
t795 = Mb.*t5.*t38.*t420;
t796 = -t677;
t797 = Mm.*t5.*t38.*t420;
t798 = -t678;
t799 = Mt.*t5.*t38.*t420;
t800 = -t679;
t801 = -t693;
t804 = t185+t387;
t805 = dth2.*t3.*t575;
t811 = dth2.*t8.*t575;
t817 = t79+t461;
t821 = -t745;
t834 = t2.*t754;
t838 = t7.*t754;
t844 = B_cg_H.*Mb.*t10.*t555;
t845 = B_cg_H.*Mb.*t10.*t557;
t846 = B_cg_H.*Mb.*t10.*t558;
t848 = -t755;
t851 = -t757;
t853 = t745./2.0;
t866 = t229+t465;
t867 = t7.*t35.*t555;
t868 = t75+t556;
t872 = t83+t560;
t874 = -t820;
t876 = t254+t444;
t885 = B_cg_H.*Mb.*t2.*t5.*t555;
t886 = B_cg_H.*Mb.*t2.*t5.*t557;
t887 = B_cg_H.*Mb.*t2.*t5.*t558;
t888 = B_cg_H.*Mb.*t5.*t7.*t555;
t889 = B_cg_H.*Mb.*t5.*t7.*t557;
t890 = B_cg_H.*Mb.*t5.*t7.*t558;
t892 = -t865;
t893 = B_cg_H.*Mb.*t324.*t381;
t896 = -t842;
t897 = B_cg_H.*Mb.*t211.*t420;
t898 = -t843;
t906 = -t849;
t907 = t820./2.0;
t917 = B_cg_H.*Mb.*t4.*t5.*t675;
t919 = B_cg_H.*Mb.*t5.*t9.*t721;
t931 = B_cg_H.*t870;
t933 = t4.*t902;
t935 = -dpsi1.*(t105-t465);
t936 = -dth2.*(t105-t465);
t937 = T_cg_H.*t870;
t938 = T_cg_H.*t871;
t941 = t9.*t902;
t942 = dphi2.*t870;
t943 = dphi2.*t871;
t944 = dth1.*t870;
t945 = dth1.*t871;
t953 = Mm.*t10.*t852;
t958 = Mb.*t381.*t421;
t959 = Mb.*t382.*t420;
t960 = Mm.*t381.*t421;
t961 = Mm.*t382.*t420;
t962 = Mt.*t381.*t421;
t963 = Mt.*t382.*t420;
t966 = dth2.*t3.*t869;
t972 = dth2.*t8.*t869;
t980 = dth2.*t3.*t873;
t984 = dth2.*t8.*t873;
t986 = t380.*t492;
t988 = t5.*t378.*t418;
t989 = t5.*t378.*t419;
t990 = t5.*t380.*t416;
t991 = t5.*t380.*t417;
t992 = -t948;
t993 = t3.*t380.*t418;
t994 = t3.*t380.*t419;
t996 = Mm.*t2.*t5.*t852;
t1003 = t2.*t952;
t1004 = Mm.*t5.*t7.*t852;
t1006 = t7.*t952;
t1009 = t116+t247+t344;
t1011 = -t952;
t1014 = B_cg_H.*Mb.*t5.*t871;
t1016 = t123+t258+t350;
t1017 = t947./2.0;
t1020 = t950./2.0;
t1031 = t201+t210+t384;
t1032 = Mb.*t420.*t421;
t1033 = Mm.*t420.*t421;
t1034 = Mt.*t420.*t421;
t1037 = t187+t309+t334;
t1038 = t195+t307+t330;
t1044 = t217+t223+t385;
t1047 = t200+t316+t337;
t1048 = t211+t315+t335;
t1050 = -t983;
t1052 = t418.*t495;
t1053 = t419.*t495;
t1059 = t98.*t871;
t1060 = t7.*t31.*t871;
t1062 = t7.*t35.*t870;
t1063 = t7.*t35.*t871;
t1064 = t7.*t39.*t871;
t1065 = -t995;
t1066 = dth1.*t1007;
t1069 = dth1.*t1013;
t1074 = -t1008;
t1075 = B_cg_H.*Mb.*t2.*t10.*t871;
t1077 = B_cg_H.*Mb.*t7.*t10.*t871;
t1078 = -t1012;
t1079 = t380.*t555;
t1080 = t380.*t558;
t1082 = t987./2.0;
t1088 = t995./2.0;
t1129 = t480.*t495;
t1137 = t418.*t555;
t1138 = t419.*t555;
t1159 = Mm.*t4.*t10.*t1007;
C = ft_2({B_cg_H,ITail,Mb,Mm,Mt,T_cg_H,dphi1,dphi2,dpsi1,dth1,dth2,dx,dy,dz,t10,t100,t1003,t1004,t1005,t1006,t1007,t1008,t1009,t1010,t1011,t1012,t1013,t1014,t1016,t1017,t1020,t103,t1031,t1032,t1033,t1034,t1037,t1038,t1044,t1047,t1048,t105,t1050,t1052,t1053,t1059,t1060,t1062,t1063,t1064,t1065,t1066,t1069,t1074,t1075,t1077,t1078,t1079,t1080,t1082,t1088,t11,t1129,t1131,t1137,t1138,t1149,t115,t1151,t1152,t1159,t116,t1185,t1186,t119,t1196,t120,t1215,t1223,t123,t1234,t124,t125,t1252,t1253,t126,t1268,t1283,t130,t1301,t1305,t1320,t1322,t1337,t1338,t134,t1343,t1344,t1345,t1348,t136,t137,t1370,t1371,t1373,t1374,t138,t1384,t1391,t1393,t1397,t141,t142,t1433,t144,t1455,t146,t148,t149,t15,t150,t152,t156,t160,t161,t162,t165,t166,t167,t169,t1692,t171,t173,t1784,t1810,t184,t195,t197,t198,t2,t211,t213,t214,t22,t225,t228,t23,t24,t241,t242,t243,t244,t245,t246,t25,t251,t252,t253,t255,t256,t257,t259,t2597,t26,t260,t261,t2617,t262,t263,t264,t266,t2660,t267,t269,t27,t270,t271,t273,t274,t275,t276,t277,t278,t28,t2819,t283,t2839,t284,t2842,t2844,t285,t2857,t286,t287,t2879,t288,t289,t290,t291,t2912,t2913,t292,t293,t294,t295,t296,t297,t2977,t298,t299,t3,t30,t300,t301,t302,t303,t3030,t304,t3052,t3202,t3209,t324,t325,t329,t33,t338,t34,t342,t345,t346,t347,t348,t35,t351,t352,t353,t354,t355,t356,t357,t358,t359,t360,t37,t370,t371,t372,t375,t376,t377,t379,t38,t380,t381,t382,t383,t388,t389,t390,t391,t392,t393,t3932,t394,t3944,t395,t3955,t396,t3965,t397,t398,t3982,t399,t3998,t4,t40,t400,t4003,t401,t4014,t402,t403,t404,t405,t406,t407,t408,t409,t41,t410,t411,t412,t413,t414,t415,t418,t419,t420,t421,t424,t425,t426,t427,t428,t429,t430,t431,t432,t433,t434,t436,t437,t438,t44,t442,t443,t445,t447,t448,t449,t45,t450,t451,t453,t454,t456,t459,t4597,t46,t460,t4603,t462,t463,t464,t465,t466,t467,t468,t469,t470,t471,t472,t473,t474,t475,t476,t477,t478,t479,t48,t480,t481,t482,t483,t484,t485,t486,t487,t488,t489,t49,t490,t491,t493,t494,t495,t496,t497,t498,t499,t5,t50,t500,t501,t502,t503,t504,t505,t506,t507,t508,t509,t51,t510,t511,t512,t514,t515,t516,t518,t519,t52,t520,t521,t522,t523,t524,t525,t526,t527,t528,t529,t530,t531,t532,t533,t534,t535,t536,t537,t538,t539,t54,t540,t541,t542,t543,t544,t545,t546,t547,t548,t549,t55,t551,t554,t555,t557,t558,t559,t56,t560,t564,t566,t567,t568,t569,t57,t575,t586,t587,t588,t59,t590,t592,t594,t595,t596,t597,t598,t599,t6,t600,t601,t602,t603,t604,t605,t607,t608,t61,t610,t611,t613,t614,t615,t616,t617,t618,t620,t621,t622,t623,t624,t625,t626,t627,t628,t629,t630,t631,t632,t65,t650,t651,t655,t656,t657,t661,t662,t663,t664,t665,t666,t667,t668,t669,t670,t672,t673,t674,t675,t676,t68,t680,t681,t682,t683,t684,t685,t686,t687,t688,t689,t69,t690,t691,t692,t693,t694,t696,t697,t698,t699,t7,t700,t701,t702,t703,t704,t705,t706,t707,t708,t709,t71,t710,t711,t712,t713,t714,t715,t716,t717,t718,t719,t720,t721,t722,t724,t725,t726,t727,t728,t729,t73,t730,t733,t734,t738,t739,t740,t741,t742,t743,t744,t745,t749,t750,t751,t752,t753,t754,t755,t756,t757,t758,t759,t760,t761,t762,t763,t764,t765,t766,t767,t768,t769,t770,t771,t772,t773,t774,t775,t776,t777,t778,t780,t781,t782,t783,t784,t785,t786,t787,t788,t789,t790,t791,t793,t794,t795,t796,t797,t798,t799,t8,t800,t801,t804,t805,t811,t817,t818,t819,t820,t821,t834,t837,t838,t839,t841,t842,t843,t844,t845,t846,t847,t848,t850,t851,t852,t853,t854,t855,t865,t867,t868,t869,t870,t871,t872,t873,t874,t876,t885,t886,t887,t888,t889,t890,t892,t893,t896,t897,t898,t899,t9,t90,t901,t902,t904,t905,t906,t907,t911,t914,t917,t919,t920,t921,t922,t927,t931,t933,t934,t935,t936,t937,t938,t941,t942,t943,t944,t945,t947,t948,t950,t952,t953,t958,t959,t960,t961,t962,t963,t966,t972,t980,t983,t984,t986,t987,t988,t989,t990,t991,t992,t993,t994,t995,t996});
end
function C = ft_2(ct)
B_cg_H = ct{1};
ITail = ct{2};
Mb = ct{3};
Mm = ct{4};
Mt = ct{5};
T_cg_H = ct{6};
dphi1 = ct{7};
dphi2 = ct{8};
dpsi1 = ct{9};
dth1 = ct{10};
dth2 = ct{11};
dx = ct{12};
dy = ct{13};
dz = ct{14};
t10 = ct{15};
t100 = ct{16};
t1003 = ct{17};
t1004 = ct{18};
t1005 = ct{19};
t1006 = ct{20};
t1007 = ct{21};
t1008 = ct{22};
t1009 = ct{23};
t1010 = ct{24};
t1011 = ct{25};
t1012 = ct{26};
t1013 = ct{27};
t1014 = ct{28};
t1016 = ct{29};
t1017 = ct{30};
t1020 = ct{31};
t103 = ct{32};
t1031 = ct{33};
t1032 = ct{34};
t1033 = ct{35};
t1034 = ct{36};
t1037 = ct{37};
t1038 = ct{38};
t1044 = ct{39};
t1047 = ct{40};
t1048 = ct{41};
t105 = ct{42};
t1050 = ct{43};
t1052 = ct{44};
t1053 = ct{45};
t1059 = ct{46};
t1060 = ct{47};
t1062 = ct{48};
t1063 = ct{49};
t1064 = ct{50};
t1065 = ct{51};
t1066 = ct{52};
t1069 = ct{53};
t1074 = ct{54};
t1075 = ct{55};
t1077 = ct{56};
t1078 = ct{57};
t1079 = ct{58};
t1080 = ct{59};
t1082 = ct{60};
t1088 = ct{61};
t11 = ct{62};
t1129 = ct{63};
t1131 = ct{64};
t1137 = ct{65};
t1138 = ct{66};
t1149 = ct{67};
t115 = ct{68};
t1151 = ct{69};
t1152 = ct{70};
t1159 = ct{71};
t116 = ct{72};
t1185 = ct{73};
t1186 = ct{74};
t119 = ct{75};
t1196 = ct{76};
t120 = ct{77};
t1215 = ct{78};
t1223 = ct{79};
t123 = ct{80};
t1234 = ct{81};
t124 = ct{82};
t125 = ct{83};
t1252 = ct{84};
t1253 = ct{85};
t126 = ct{86};
t1268 = ct{87};
t1283 = ct{88};
t130 = ct{89};
t1301 = ct{90};
t1305 = ct{91};
t1320 = ct{92};
t1322 = ct{93};
t1337 = ct{94};
t1338 = ct{95};
t134 = ct{96};
t1343 = ct{97};
t1344 = ct{98};
t1345 = ct{99};
t1348 = ct{100};
t136 = ct{101};
t137 = ct{102};
t1370 = ct{103};
t1371 = ct{104};
t1373 = ct{105};
t1374 = ct{106};
t138 = ct{107};
t1384 = ct{108};
t1391 = ct{109};
t1393 = ct{110};
t1397 = ct{111};
t141 = ct{112};
t142 = ct{113};
t1433 = ct{114};
t144 = ct{115};
t1455 = ct{116};
t146 = ct{117};
t148 = ct{118};
t149 = ct{119};
t15 = ct{120};
t150 = ct{121};
t152 = ct{122};
t156 = ct{123};
t160 = ct{124};
t161 = ct{125};
t162 = ct{126};
t165 = ct{127};
t166 = ct{128};
t167 = ct{129};
t169 = ct{130};
t1692 = ct{131};
t171 = ct{132};
t173 = ct{133};
t1784 = ct{134};
t1810 = ct{135};
t184 = ct{136};
t195 = ct{137};
t197 = ct{138};
t198 = ct{139};
t2 = ct{140};
t211 = ct{141};
t213 = ct{142};
t214 = ct{143};
t22 = ct{144};
t225 = ct{145};
t228 = ct{146};
t23 = ct{147};
t24 = ct{148};
t241 = ct{149};
t242 = ct{150};
t243 = ct{151};
t244 = ct{152};
t245 = ct{153};
t246 = ct{154};
t25 = ct{155};
t251 = ct{156};
t252 = ct{157};
t253 = ct{158};
t255 = ct{159};
t256 = ct{160};
t257 = ct{161};
t259 = ct{162};
t2597 = ct{163};
t26 = ct{164};
t260 = ct{165};
t261 = ct{166};
t2617 = ct{167};
t262 = ct{168};
t263 = ct{169};
t264 = ct{170};
t266 = ct{171};
t2660 = ct{172};
t267 = ct{173};
t269 = ct{174};
t27 = ct{175};
t270 = ct{176};
t271 = ct{177};
t273 = ct{178};
t274 = ct{179};
t275 = ct{180};
t276 = ct{181};
t277 = ct{182};
t278 = ct{183};
t28 = ct{184};
t2819 = ct{185};
t283 = ct{186};
t2839 = ct{187};
t284 = ct{188};
t2842 = ct{189};
t2844 = ct{190};
t285 = ct{191};
t2857 = ct{192};
t286 = ct{193};
t287 = ct{194};
t2879 = ct{195};
t288 = ct{196};
t289 = ct{197};
t290 = ct{198};
t291 = ct{199};
t2912 = ct{200};
t2913 = ct{201};
t292 = ct{202};
t293 = ct{203};
t294 = ct{204};
t295 = ct{205};
t296 = ct{206};
t297 = ct{207};
t2977 = ct{208};
t298 = ct{209};
t299 = ct{210};
t3 = ct{211};
t30 = ct{212};
t300 = ct{213};
t301 = ct{214};
t302 = ct{215};
t303 = ct{216};
t3030 = ct{217};
t304 = ct{218};
t3052 = ct{219};
t3202 = ct{220};
t3209 = ct{221};
t324 = ct{222};
t325 = ct{223};
t329 = ct{224};
t33 = ct{225};
t338 = ct{226};
t34 = ct{227};
t342 = ct{228};
t345 = ct{229};
t346 = ct{230};
t347 = ct{231};
t348 = ct{232};
t35 = ct{233};
t351 = ct{234};
t352 = ct{235};
t353 = ct{236};
t354 = ct{237};
t355 = ct{238};
t356 = ct{239};
t357 = ct{240};
t358 = ct{241};
t359 = ct{242};
t360 = ct{243};
t37 = ct{244};
t370 = ct{245};
t371 = ct{246};
t372 = ct{247};
t375 = ct{248};
t376 = ct{249};
t377 = ct{250};
t379 = ct{251};
t38 = ct{252};
t380 = ct{253};
t381 = ct{254};
t382 = ct{255};
t383 = ct{256};
t388 = ct{257};
t389 = ct{258};
t390 = ct{259};
t391 = ct{260};
t392 = ct{261};
t393 = ct{262};
t3932 = ct{263};
t394 = ct{264};
t3944 = ct{265};
t395 = ct{266};
t3955 = ct{267};
t396 = ct{268};
t3965 = ct{269};
t397 = ct{270};
t398 = ct{271};
t3982 = ct{272};
t399 = ct{273};
t3998 = ct{274};
t4 = ct{275};
t40 = ct{276};
t400 = ct{277};
t4003 = ct{278};
t401 = ct{279};
t4014 = ct{280};
t402 = ct{281};
t403 = ct{282};
t404 = ct{283};
t405 = ct{284};
t406 = ct{285};
t407 = ct{286};
t408 = ct{287};
t409 = ct{288};
t41 = ct{289};
t410 = ct{290};
t411 = ct{291};
t412 = ct{292};
t413 = ct{293};
t414 = ct{294};
t415 = ct{295};
t418 = ct{296};
t419 = ct{297};
t420 = ct{298};
t421 = ct{299};
t424 = ct{300};
t425 = ct{301};
t426 = ct{302};
t427 = ct{303};
t428 = ct{304};
t429 = ct{305};
t430 = ct{306};
t431 = ct{307};
t432 = ct{308};
t433 = ct{309};
t434 = ct{310};
t436 = ct{311};
t437 = ct{312};
t438 = ct{313};
t44 = ct{314};
t442 = ct{315};
t443 = ct{316};
t445 = ct{317};
t447 = ct{318};
t448 = ct{319};
t449 = ct{320};
t45 = ct{321};
t450 = ct{322};
t451 = ct{323};
t453 = ct{324};
t454 = ct{325};
t456 = ct{326};
t459 = ct{327};
t4597 = ct{328};
t46 = ct{329};
t460 = ct{330};
t4603 = ct{331};
t462 = ct{332};
t463 = ct{333};
t464 = ct{334};
t465 = ct{335};
t466 = ct{336};
t467 = ct{337};
t468 = ct{338};
t469 = ct{339};
t470 = ct{340};
t471 = ct{341};
t472 = ct{342};
t473 = ct{343};
t474 = ct{344};
t475 = ct{345};
t476 = ct{346};
t477 = ct{347};
t478 = ct{348};
t479 = ct{349};
t48 = ct{350};
t480 = ct{351};
t481 = ct{352};
t482 = ct{353};
t483 = ct{354};
t484 = ct{355};
t485 = ct{356};
t486 = ct{357};
t487 = ct{358};
t488 = ct{359};
t489 = ct{360};
t49 = ct{361};
t490 = ct{362};
t491 = ct{363};
t493 = ct{364};
t494 = ct{365};
t495 = ct{366};
t496 = ct{367};
t497 = ct{368};
t498 = ct{369};
t499 = ct{370};
t5 = ct{371};
t50 = ct{372};
t500 = ct{373};
t501 = ct{374};
t502 = ct{375};
t503 = ct{376};
t504 = ct{377};
t505 = ct{378};
t506 = ct{379};
t507 = ct{380};
t508 = ct{381};
t509 = ct{382};
t51 = ct{383};
t510 = ct{384};
t511 = ct{385};
t512 = ct{386};
t514 = ct{387};
t515 = ct{388};
t516 = ct{389};
t518 = ct{390};
t519 = ct{391};
t52 = ct{392};
t520 = ct{393};
t521 = ct{394};
t522 = ct{395};
t523 = ct{396};
t524 = ct{397};
t525 = ct{398};
t526 = ct{399};
t527 = ct{400};
t528 = ct{401};
t529 = ct{402};
t530 = ct{403};
t531 = ct{404};
t532 = ct{405};
t533 = ct{406};
t534 = ct{407};
t535 = ct{408};
t536 = ct{409};
t537 = ct{410};
t538 = ct{411};
t539 = ct{412};
t54 = ct{413};
t540 = ct{414};
t541 = ct{415};
t542 = ct{416};
t543 = ct{417};
t544 = ct{418};
t545 = ct{419};
t546 = ct{420};
t547 = ct{421};
t548 = ct{422};
t549 = ct{423};
t55 = ct{424};
t551 = ct{425};
t554 = ct{426};
t555 = ct{427};
t557 = ct{428};
t558 = ct{429};
t559 = ct{430};
t56 = ct{431};
t560 = ct{432};
t564 = ct{433};
t566 = ct{434};
t567 = ct{435};
t568 = ct{436};
t569 = ct{437};
t57 = ct{438};
t575 = ct{439};
t586 = ct{440};
t587 = ct{441};
t588 = ct{442};
t59 = ct{443};
t590 = ct{444};
t592 = ct{445};
t594 = ct{446};
t595 = ct{447};
t596 = ct{448};
t597 = ct{449};
t598 = ct{450};
t599 = ct{451};
t6 = ct{452};
t600 = ct{453};
t601 = ct{454};
t602 = ct{455};
t603 = ct{456};
t604 = ct{457};
t605 = ct{458};
t607 = ct{459};
t608 = ct{460};
t61 = ct{461};
t610 = ct{462};
t611 = ct{463};
t613 = ct{464};
t614 = ct{465};
t615 = ct{466};
t616 = ct{467};
t617 = ct{468};
t618 = ct{469};
t620 = ct{470};
t621 = ct{471};
t622 = ct{472};
t623 = ct{473};
t624 = ct{474};
t625 = ct{475};
t626 = ct{476};
t627 = ct{477};
t628 = ct{478};
t629 = ct{479};
t630 = ct{480};
t631 = ct{481};
t632 = ct{482};
t65 = ct{483};
t650 = ct{484};
t651 = ct{485};
t655 = ct{486};
t656 = ct{487};
t657 = ct{488};
t661 = ct{489};
t662 = ct{490};
t663 = ct{491};
t664 = ct{492};
t665 = ct{493};
t666 = ct{494};
t667 = ct{495};
t668 = ct{496};
t669 = ct{497};
t670 = ct{498};
t672 = ct{499};
t673 = ct{500};
t674 = ct{501};
t675 = ct{502};
t676 = ct{503};
t68 = ct{504};
t680 = ct{505};
t681 = ct{506};
t682 = ct{507};
t683 = ct{508};
t684 = ct{509};
t685 = ct{510};
t686 = ct{511};
t687 = ct{512};
t688 = ct{513};
t689 = ct{514};
t69 = ct{515};
t690 = ct{516};
t691 = ct{517};
t692 = ct{518};
t693 = ct{519};
t694 = ct{520};
t696 = ct{521};
t697 = ct{522};
t698 = ct{523};
t699 = ct{524};
t7 = ct{525};
t700 = ct{526};
t701 = ct{527};
t702 = ct{528};
t703 = ct{529};
t704 = ct{530};
t705 = ct{531};
t706 = ct{532};
t707 = ct{533};
t708 = ct{534};
t709 = ct{535};
t71 = ct{536};
t710 = ct{537};
t711 = ct{538};
t712 = ct{539};
t713 = ct{540};
t714 = ct{541};
t715 = ct{542};
t716 = ct{543};
t717 = ct{544};
t718 = ct{545};
t719 = ct{546};
t720 = ct{547};
t721 = ct{548};
t722 = ct{549};
t724 = ct{550};
t725 = ct{551};
t726 = ct{552};
t727 = ct{553};
t728 = ct{554};
t729 = ct{555};
t73 = ct{556};
t730 = ct{557};
t733 = ct{558};
t734 = ct{559};
t738 = ct{560};
t739 = ct{561};
t740 = ct{562};
t741 = ct{563};
t742 = ct{564};
t743 = ct{565};
t744 = ct{566};
t745 = ct{567};
t749 = ct{568};
t750 = ct{569};
t751 = ct{570};
t752 = ct{571};
t753 = ct{572};
t754 = ct{573};
t755 = ct{574};
t756 = ct{575};
t757 = ct{576};
t758 = ct{577};
t759 = ct{578};
t760 = ct{579};
t761 = ct{580};
t762 = ct{581};
t763 = ct{582};
t764 = ct{583};
t765 = ct{584};
t766 = ct{585};
t767 = ct{586};
t768 = ct{587};
t769 = ct{588};
t770 = ct{589};
t771 = ct{590};
t772 = ct{591};
t773 = ct{592};
t774 = ct{593};
t775 = ct{594};
t776 = ct{595};
t777 = ct{596};
t778 = ct{597};
t780 = ct{598};
t781 = ct{599};
t782 = ct{600};
t783 = ct{601};
t784 = ct{602};
t785 = ct{603};
t786 = ct{604};
t787 = ct{605};
t788 = ct{606};
t789 = ct{607};
t790 = ct{608};
t791 = ct{609};
t793 = ct{610};
t794 = ct{611};
t795 = ct{612};
t796 = ct{613};
t797 = ct{614};
t798 = ct{615};
t799 = ct{616};
t8 = ct{617};
t800 = ct{618};
t801 = ct{619};
t804 = ct{620};
t805 = ct{621};
t811 = ct{622};
t817 = ct{623};
t818 = ct{624};
t819 = ct{625};
t820 = ct{626};
t821 = ct{627};
t834 = ct{628};
t837 = ct{629};
t838 = ct{630};
t839 = ct{631};
t841 = ct{632};
t842 = ct{633};
t843 = ct{634};
t844 = ct{635};
t845 = ct{636};
t846 = ct{637};
t847 = ct{638};
t848 = ct{639};
t850 = ct{640};
t851 = ct{641};
t852 = ct{642};
t853 = ct{643};
t854 = ct{644};
t855 = ct{645};
t865 = ct{646};
t867 = ct{647};
t868 = ct{648};
t869 = ct{649};
t870 = ct{650};
t871 = ct{651};
t872 = ct{652};
t873 = ct{653};
t874 = ct{654};
t876 = ct{655};
t885 = ct{656};
t886 = ct{657};
t887 = ct{658};
t888 = ct{659};
t889 = ct{660};
t890 = ct{661};
t892 = ct{662};
t893 = ct{663};
t896 = ct{664};
t897 = ct{665};
t898 = ct{666};
t899 = ct{667};
t9 = ct{668};
t90 = ct{669};
t901 = ct{670};
t902 = ct{671};
t904 = ct{672};
t905 = ct{673};
t906 = ct{674};
t907 = ct{675};
t911 = ct{676};
t914 = ct{677};
t917 = ct{678};
t919 = ct{679};
t920 = ct{680};
t921 = ct{681};
t922 = ct{682};
t927 = ct{683};
t931 = ct{684};
t933 = ct{685};
t934 = ct{686};
t935 = ct{687};
t936 = ct{688};
t937 = ct{689};
t938 = ct{690};
t941 = ct{691};
t942 = ct{692};
t943 = ct{693};
t944 = ct{694};
t945 = ct{695};
t947 = ct{696};
t948 = ct{697};
t950 = ct{698};
t952 = ct{699};
t953 = ct{700};
t958 = ct{701};
t959 = ct{702};
t960 = ct{703};
t961 = ct{704};
t962 = ct{705};
t963 = ct{706};
t966 = ct{707};
t972 = ct{708};
t980 = ct{709};
t983 = ct{710};
t984 = ct{711};
t986 = ct{712};
t987 = ct{713};
t988 = ct{714};
t989 = ct{715};
t990 = ct{716};
t991 = ct{717};
t992 = ct{718};
t993 = ct{719};
t994 = ct{720};
t995 = ct{721};
t996 = ct{722};
t1160 = Mm.*t5.*t9.*t1007;
t1161 = B_cg_H.*Mb.*t381.*t675;
t1164 = Mm.*t4.*t5.*t1013;
t1165 = B_cg_H.*Mb.*t382.*t721;
t1173 = Mm.*t9.*t10.*t1013;
t1176 = t480.*t555;
t1177 = t485.*t555;
t1187 = Mm.*t421.*t651;
t1188 = -t1151;
t1190 = t1131./2.0;
t1191 = Mm.*t420.*t657;
t1192 = -t1152;
t1198 = t146+t402+t405;
t1201 = B_cg_H.*Mb.*t421.*t675;
t1203 = Mm.*t5.*t33.*t1013;
t1205 = t150+t407+t408;
t1206 = Mm.*t5.*t38.*t1013;
t1212 = B_cg_H.*Mb.*t420.*t721;
t1242 = Mb.*t15.*t1131;
t1245 = Mm.*t5.*t30.*t1007;
t1246 = Mb.*t7.*t15.*t100.*t871;
t1247 = Mm.*t5.*t34.*t1007;
t1249 = t418.*t819;
t1250 = t419.*t819;
t1251 = -t1185;
t1261 = t379.*t871;
t1262 = t380.*t870;
t1263 = t380.*t871;
t1264 = t1185./2.0;
t1265 = t270+t406+t409;
t1281 = t278+t403+t404;
t1304 = Mb.*t15.*t485.*t558;
t1319 = t480.*t819;
t1328 = t418.*t870;
t1329 = t418.*t871;
t1330 = t419.*t870;
t1331 = t419.*t871;
t1378 = Mm.*t524.*t852;
t1379 = t495.*t870;
t1380 = t495.*t871;
t1402 = t1320./2.0;
t1415 = Mm.*t381.*t1013;
t1416 = Mm.*t382.*t1013;
t1428 = -t9.*t480.*(t105-t465);
t1429 = -t9.*t485.*(t105-t465);
t1434 = -t3.*t496.*(t105-t465);
t1442 = t555.*t870;
t1443 = t555.*t871;
t1444 = Mb.*t15.*t1320;
t1446 = t3.*t496.*t873;
t1457 = Mm.*t381.*t1007;
t1458 = Mm.*t382.*t1007;
t1460 = -t1384;
t1485 = Mm.*t420.*t1013;
t1486 = Mm.*t421.*t1013;
t1495 = t372+t442+t615;
t1502 = -t698.*(t105-t465);
t1507 = t9.*t480.*(t105-t465);
t1514 = -t3.*t575.*(t105-t465);
t1526 = -t1455;
t1529 = Mm.*t420.*t1007;
t1530 = Mm.*t421.*t1007;
t1531 = t393+t427+t588;
t1539 = t9.*t485.*(t105-t465).*(-1.0./2.0);
t1542 = t3.*t496.*(t105-t465).*(-1.0./2.0);
t1582 = t698.*(t105-t465);
t1596 = Mb.*t15.*t557.*t871;
t1597 = Mb.*t15.*t558.*t871;
t1613 = t3.*t575.*(t105-t465).*(-1.0./2.0);
t1616 = t819.*t870;
t1617 = t819.*t871;
t1645 = t745.*6.73108e-3;
t1648 = -t3.*t818.*(t105-t465);
t1661 = t871.*t911;
t1664 = Mm.*t657.*t1013;
t1675 = t745.*3.36554e-3;
t1693 = Mm.*t651.*t1007;
t1712 = -t9.*t870.*(t105-t465);
t1713 = -t9.*t871.*(t105-t465);
t1714 = -t3.*t873.*(t105-t465);
t1717 = -t8.*t873.*(t105-t465);
t1723 = -t1692;
t1728 = t820.*3.36554e-3;
t1733 = t3.*t818.*(t105-t465).*(-1.0./2.0);
t1775 = t9.*t871.*(t105-t465);
t1798 = t745.*3.372786875e-3;
t1799 = t745.*6.74557375e-3;
t1803 = t9.*t870.*(t105-t465).*(-1.0./2.0);
t1805 = t3.*t873.*(t105-t465).*(-1.0./2.0);
t1806 = t745.*9.53094055e-4;
t1807 = t745.*1.90618811e-3;
t1808 = t8.*t873.*(t105-t465).*(-1.0./2.0);
t1814 = -t1784;
t1841 = -t1810;
t1861 = t820.*3.367829185e-3;
t1865 = t947.*3.36554e-3;
t1867 = t950.*3.36554e-3;
t1892 = t820.*8.56645e-6;
t1906 = t987.*3.36554e-3;
t1915 = t995.*3.36554e-3;
t1971 = t947.*3.372786875e-3;
t1973 = t950.*3.372786875e-3;
t1974 = t947.*9.53094055e-4;
t1975 = t950.*9.53094055e-4;
t2043 = t987.*3.372786875e-3;
t2053 = t987.*9.53094055e-4;
t2062 = t28+t57+t160+t656+t905;
t2066 = t1131.*3.36554e-3;
t2067 = t995.*3.367829185e-3;
t2087 = t371+t395+t443+t899;
t2141 = t995.*8.56645e-6;
t2172 = t1185.*3.36554e-3;
t2238 = t1131.*9.52624335e-4;
t2245 = t1131.*3.372816795e-3;
t2324 = t1185.*3.372786875e-3;
t2326 = t1185.*9.53094055e-4;
t2339 = t1320.*3.36554e-3;
t2479 = t9.*t485.*(t105-t465).*(-3.36554e-3);
t2485 = t3.*t496.*(t105-t465).*(-3.36554e-3);
t2505 = t1320.*9.52624335e-4;
t2512 = t1320.*3.372816795e-3;
t2531 = t9.*t485.*(t105-t465).*3.36554e-3;
t2581 = t3.*t575.*(t105-t465).*(-3.36554e-3);
t2692 = t9.*t485.*(t105-t465).*(-3.372786875e-3);
t2698 = t3.*t496.*(t105-t465).*(-3.372786875e-3);
t2699 = t9.*t485.*(t105-t465).*(-9.53094055e-4);
t2704 = t3.*t496.*(t105-t465).*(-9.53094055e-4);
t2742 = t9.*t485.*(t105-t465).*3.372786875e-3;
t2783 = t3.*t575.*(t105-t465).*(-3.372786875e-3);
t2784 = t3.*t575.*(t105-t465).*(-9.53094055e-4);
t2804 = t3.*t818.*(t105-t465).*(-3.36554e-3);
t2872 = t9.*t870.*(t105-t465).*(-3.36554e-3);
t2874 = t3.*t873.*(t105-t465).*(-3.36554e-3);
t2875 = t8.*t873.*(t105-t465).*(-3.36554e-3);
t2946 = t3.*t818.*(t105-t465).*(-3.372786875e-3);
t2951 = t3.*t818.*(t105-t465).*(-9.53094055e-4);
t3017 = t9.*t870.*(t105-t465).*(-3.372786875e-3);
t3019 = t3.*t873.*(t105-t465).*(-3.372786875e-3);
t3022 = t8.*t873.*(t105-t465).*(-3.372786875e-3);
t3023 = t9.*t870.*(t105-t465).*(-9.53094055e-4);
t3025 = t3.*t873.*(t105-t465).*(-9.53094055e-4);
t3028 = t8.*t873.*(t105-t465).*(-9.53094055e-4);
t3109 = -t3052;
t3260 = dz.*t3202;
t3264 = dy.*t3209;
t4008 = -t3982;
t4033 = -t3998;
t4038 = -t4014;
t550 = t8.*t488;
t552 = t3.*t494;
t553 = t6.*t497;
t561 = t11.*t497;
t562 = t11.*t498;
t563 = t11.*t499;
t565 = -t493;
t570 = -t498;
t571 = -t500;
t572 = -t501;
t573 = -t502;
t574 = -t503;
t576 = Mb.*t525;
t577 = Mb.*t526;
t578 = -t508;
t579 = Mm.*t525;
t580 = Mm.*t526;
t581 = -t510;
t582 = Mt.*t525;
t583 = Mt.*t526;
t584 = -t512;
t619 = t3.*t488;
t633 = t6.*t542;
t634 = t6.*t543;
t635 = -t534;
t636 = t11.*t543;
t637 = t6.*t545;
t638 = t8.*t544;
t639 = -t539;
t640 = t11.*t546;
t641 = -t542;
t642 = -t548;
t643 = t532./2.0;
t645 = -t551;
t647 = -t554;
t648 = t533./2.0;
t671 = -t586;
t695 = -t596;
t723 = T_cg_H.*t11.*t542;
t735 = -t621;
t736 = -t622;
t737 = -t624;
t746 = B_cg_H.*t3.*t11.*t507;
t779 = -t661;
t792 = -t751;
t802 = -t696;
t803 = -t697;
t806 = -t700;
t807 = -t702;
t808 = -t705;
t809 = -t710;
t810 = -t715;
t812 = -t725;
t813 = -t727;
t814 = -t729;
t815 = -t739;
t816 = -t743;
t822 = -t758;
t825 = t534.*(2.7e+1./1.0e+2);
t826 = t535.*(2.7e+1./1.0e+2);
t827 = t11.*t749;
t828 = t537.*(2.7e+1./1.0e+2);
t829 = t538.*(2.7e+1./1.0e+2);
t830 = t539.*(2.7e+1./1.0e+2);
t831 = t541.*(2.7e+1./1.0e+2);
t832 = t542.*(2.7e+1./1.0e+2);
t833 = t543.*(2.7e+1./1.0e+2);
t835 = t545.*(2.7e+1./1.0e+2);
t836 = t546.*(2.7e+1./1.0e+2);
t856 = -t763;
t857 = -t767;
t860 = dphi1.*t794;
t861 = dphi1.*t804;
t864 = -t793;
t875 = -t853;
t891 = -t838;
t894 = dpsi1.*t817;
t895 = dth2.*t817;
t900 = -t846;
t903 = t90+t547;
t915 = -t867;
t916 = -t907;
t918 = t868.^2;
t923 = -t886;
t924 = -t887;
t925 = t211+t535;
t926 = B_cg_H.*t868;
t928 = -t888;
t932 = T_cg_H.*t868;
t939 = dphi2.*t868;
t940 = dth1.*t868;
t946 = t228+t544;
t949 = t867./2.0;
t951 = B_cg_H.*t943;
t955 = -t917;
t957 = -t919;
t967 = t325+t537;
t968 = t4.*t944;
t969 = t4.*t945;
t971 = dth2.*t3.*t872;
t973 = -dpsi1.*(t103-t544);
t975 = -dth2.*(t103-t544);
t978 = t9.*t944;
t979 = t9.*t945;
t981 = dth2.*t8.*t872;
t982 = t329+t541;
t985 = Mt.*t10.*t876;
t997 = t958.*2.0;
t998 = t959.*2.0;
t999 = t960.*2.0;
t1000 = t961.*2.0;
t1001 = t962.*2.0;
t1002 = t963.*2.0;
t1018 = t993.*2.0;
t1019 = t994.*2.0;
t1022 = -T_cg_H.*(t197-t537);
t1026 = -dphi2.*(t197-t537);
t1027 = -dpsi1.*(t197-t537);
t1028 = -T_cg_H.*(t214-t541);
t1035 = -dphi2.*(t214-t541);
t1036 = -dpsi1.*(t214-t541);
t1040 = Mt.*t2.*t5.*t876;
t1043 = -t972;
t1045 = Mt.*t5.*t7.*t876;
t1051 = -t984;
t1054 = -t988;
t1055 = -t989;
t1056 = -t991;
t1057 = -t994;
t1061 = t7.*t35.*t868;
t1067 = -t1004;
t1071 = -B_cg_H.*dth2.*(t197-t537);
t1072 = t2.*t1014;
t1076 = t7.*t1014;
t1081 = t986./2.0;
t1083 = t988./2.0;
t1084 = t989./2.0;
t1085 = t990./2.0;
t1086 = t991./2.0;
t1087 = B_cg_H.*t1031;
t1089 = B_cg_H.*t1038;
t1090 = T_cg_H.*t1031;
t1091 = T_cg_H.*t1037;
t1092 = T_cg_H.*t1038;
t1093 = dphi2.*t1031;
t1094 = dpsi1.*t1031;
t1096 = B_cg_H.*t1044;
t1097 = dphi2.*t1037;
t1098 = dpsi1.*t1037;
t1100 = B_cg_H.*t1048;
t1101 = T_cg_H.*t1044;
t1102 = dpsi1.*(t197-t537);
t1103 = T_cg_H.*t1047;
t1104 = T_cg_H.*t1048;
t1105 = dphi2.*t1044;
t1106 = dpsi1.*t1044;
t1108 = dphi2.*t1047;
t1109 = dpsi1.*t1047;
t1110 = -t1032;
t1111 = -t1033;
t1112 = -t1034;
t1113 = dphi2.*(t214-t541);
t1116 = -t1053;
t1120 = -t1059;
t1121 = -t1060;
t1122 = -t1063;
t1123 = -t1064;
t1124 = -t1088;
t1126 = -t1066;
t1127 = B_cg_H.*Mb.*t459.*t547;
t1128 = B_cg_H.*Mb.*t420.*t537;
t1130 = -t1069;
t1134 = -t1075;
t1136 = -t1077;
t1139 = t35.*t37.*t868;
t1140 = t1052./2.0;
t1141 = t1053./2.0;
t1142 = t1059./2.0;
t1143 = t1060./2.0;
t1145 = t1062./2.0;
t1146 = t1063./2.0;
t1147 = t1064./2.0;
t1153 = t1079./2.0;
t1154 = t1080./2.0;
t1158 = Mm.*t4.*t5.*t1009;
t1166 = -B_cg_H.*Mb.*t4.*t5.*(t197-t537);
t1169 = t528+t625;
t1170 = t531+t621;
t1172 = Mm.*t5.*t9.*t1016;
t1174 = -B_cg_H.*Mb.*t9.*t10.*(t197-t537);
t1175 = -B_cg_H.*Mb.*t5.*t9.*(t214-t541);
t1179 = t538+t543;
t1181 = t535+t545;
t1182 = -t1137;
t1183 = -t1138;
t1189 = t1129./2.0;
t1193 = t1137./2.0;
t1194 = t1138./2.0;
t1199 = -t1159;
t1200 = -t1160;
t1204 = -B_cg_H.*Mb.*t5.*t33.*(t197-t537);
t1209 = B_cg_H.*Mb.*t4.*t5.*t1037;
t1211 = -t1164;
t1213 = -t1165;
t1214 = -B_cg_H.*Mb.*t5.*t38.*(t197-t537);
t1222 = t622+t626;
t1232 = -t1173;
t1235 = B_cg_H.*Mb.*t5.*t9.*t1047;
t1236 = B_cg_H.*Mb.*t5.*t9.*(t214-t541);
t1237 = -t1176;
t1255 = t1176./2.0;
t1256 = t1177./2.0;
t1257 = -t1187;
t1260 = t380.*t868;
t1270 = -t1201;
t1272 = -t1203;
t1275 = B_cg_H.*Mb.*t5.*t33.*(t197-t537);
t1277 = -B_cg_H.*(t534-t546);
t1284 = -t1212;
t1285 = B_cg_H.*Mb.*t5.*t38.*(t197-t537);
t1287 = -T_cg_H.*(t534-t546);
t1294 = -dphi1.*(t534-t546);
t1296 = -dphi2.*(t534-t546);
t1298 = -dpsi1.*(t534-t546);
t1302 = Mb.*t15.*t1177;
t1307 = -t1242;
t1308 = -t1245;
t1309 = -t1246;
t1311 = -t1249;
t1312 = -t1250;
t1313 = -t1264;
t1323 = t418.*t868;
t1324 = t419.*t868;
t1332 = -t1263;
t1333 = t1249./2.0;
t1334 = t1250./2.0;
t1341 = dphi1.*(t534-t546);
t1342 = dpsi1.*(t534-t546);
t1354 = t1261./2.0;
t1355 = t1262./2.0;
t1356 = t1263./2.0;
t1365 = t480.*t868;
t1366 = t481.*t868;
t1368 = t485.*t868;
t1372 = t4.*t11.*t381.*t868;
t1376 = t495.*t868;
t1377 = t11.*t459.*t872;
t1385 = -t1330;
t1399 = t1319./2.0;
t1409 = t1328./2.0;
t1410 = t1329./2.0;
t1411 = t1330./2.0;
t1412 = t1331./2.0;
t1417 = -B_cg_H.*Mb.*t381.*(t197-t537);
t1418 = -B_cg_H.*Mb.*t382.*(t197-t537);
t1420 = Mm.*t382.*t1016;
t1422 = -B_cg_H.*Mb.*t382.*(t214-t541);
t1427 = t4.*t487.*t868;
t1431 = t3.*t487.*t872;
t1436 = t555.*t868;
t1441 = t9.*t496.*t868;
t1448 = t564.*t868;
t1449 = t566.*t868;
t1450 = t567.*t868;
t1452 = t9.*t11.*t420.*t868;
t1453 = -t1378;
t1454 = t11.*t542.*t873;
t1456 = t40+t595+t670;
t1459 = Mm.*t381.*t1009;
t1478 = t1379./2.0;
t1479 = t1380./2.0;
t1481 = B_cg_H.*Mb.*t381.*t1037;
t1489 = -B_cg_H.*Mb.*t420.*(t197-t537);
t1490 = -B_cg_H.*Mb.*t421.*(t197-t537);
t1491 = B_cg_H.*Mb.*t381.*(t197-t537);
t1492 = Mm.*t420.*t1016;
t1499 = B_cg_H.*Mb.*t382.*t1047;
t1500 = -B_cg_H.*Mb.*t420.*(t214-t541);
t1506 = t11.*t381.*t1037;
t1509 = -t496.*(t214-t541);
t1517 = -t11.*t420.*(t214-t541);
t1518 = -t1444;
t1521 = Mb.*t15.*t1380;
t1532 = Mm.*t421.*t1009;
t1538 = t1507.*(-1.0./2.0);
t1548 = t1442./2.0;
t1549 = t1443./2.0;
t1550 = t11.*t542.*(t105-t465).*(-1.0./2.0);
t1552 = t1446./2.0;
t1559 = B_cg_H.*Mb.*t421.*t1037;
t1562 = -t1485;
t1563 = t532.*3.36554e-3;
t1565 = B_cg_H.*Mb.*t421.*(t197-t537);
t1567 = t487.*t1037;
t1568 = t533.*3.36554e-3;
t1576 = B_cg_H.*Mb.*t420.*t1047;
t1588 = t1507./2.0;
t1591 = t496.*t1047;
t1593 = Mb.*t15.*t1443;
t1598 = t11.*t420.*t1047;
t1600 = dth2.*t1531;
t1605 = -t1530;
t1608 = t1582.*(-1.0./2.0);
t1610 = t496.*(t214-t541).*(-1.0./2.0);
t1614 = t11.*t420.*(t214-t541).*(-1.0./2.0);
t1615 = t819.*t868;
t1618 = t388+t469+t680;
t1619 = t370+t462+t682;
t1620 = t389+t468+t683;
t1632 = t1582./2.0;
t1635 = Mt.*t5.*t1531;
t1639 = -t1596;
t1640 = -t1597;
t1642 = Mt.*t10.*t1495;
t1647 = t9.*t817.*t868;
t1651 = t3.*t817.*t873;
t1653 = t868.*t870;
t1654 = t868.*t871;
t1663 = t532.*3.372786875e-3;
t1667 = t533.*3.372786875e-3;
t1670 = t532.*9.53094055e-4;
t1671 = Mt.*t2.*t10.*t1531;
t1673 = t533.*9.53094055e-4;
t1674 = -t1645;
t1677 = Mt.*t7.*t10.*t1531;
t1684 = Mt.*t2.*t5.*t1495;
t1685 = Mt.*t5.*t7.*t1495;
t1690 = t1616./2.0;
t1691 = t1617./2.0;
t1700 = -t817.*(t214-t541);
t1704 = -t11.*t381.*(t534-t546);
t1709 = -t9.*t868.*(t105-t465);
t1718 = Mb.*t15.*t1617;
t1727 = t432+t515+t766;
t1734 = t449+t520+t770;
t1747 = -Mb.*t15.*t721.*(t197-t537);
t1749 = -t487.*(t534-t546);
t1761 = t817.*t1047;
t1762 = (t105-t465).*(t214-t541);
t1765 = -t1728;
t1766 = -t4.*t868.*(t103-t544);
t1773 = -t3.*t872.*(t103-t544);
t1786 = t867.*3.36554e-3;
t1788 = t817.*(t214-t541).*(-1.0./2.0);
t1791 = t11.*t381.*(t534-t546).*(-1.0./2.0);
t1796 = t9.*t868.*(t105-t465).*(-1.0./2.0);
t1804 = t1775.*(-1.0./2.0);
t1812 = -t1031.*(t105-t465);
t1815 = -t1037.*(t105-t465);
t1818 = -t9.*t871.*(t197-t537);
t1825 = -t8.*t873.*(t197-t537);
t1829 = -t1047.*(t105-t465);
C = ft_3({B_cg_H,ITail,Mb,Mm,Mt,T_cg_H,dphi1,dphi2,dpsi1,dth1,dth2,dx,dy,dz,t10,t100,t1000,t1001,t1002,t1003,t1004,t1005,t1006,t1007,t1008,t1009,t1010,t1011,t1012,t1013,t1014,t1016,t1017,t1018,t1019,t1020,t1022,t1026,t1028,t103,t1031,t1036,t1037,t1040,t1043,t1044,t1045,t1047,t105,t1050,t1051,t1052,t1053,t1054,t1055,t1056,t1057,t1059,t1060,t1061,t1062,t1063,t1064,t1065,t1067,t1071,t1072,t1074,t1075,t1076,t1077,t1078,t1079,t1080,t1081,t1082,t1083,t1084,t1085,t1086,t1087,t1088,t1089,t1090,t1091,t1092,t1093,t1094,t1096,t1097,t1098,t11,t1100,t1101,t1102,t1103,t1104,t1105,t1106,t1108,t1109,t1110,t1111,t1112,t1113,t1116,t1120,t1121,t1122,t1123,t1124,t1126,t1127,t1128,t1129,t1130,t1131,t1134,t1136,t1137,t1138,t1139,t1140,t1141,t1142,t1143,t1145,t1146,t1147,t1149,t115,t1152,t1153,t1154,t1158,t1159,t116,t1160,t1161,t1164,t1165,t1166,t1169,t1170,t1172,t1173,t1174,t1176,t1177,t1179,t1181,t1182,t1183,t1185,t1186,t1187,t1188,t1189,t119,t1190,t1191,t1192,t1193,t1194,t1196,t1198,t1199,t120,t1200,t1201,t1203,t1205,t1206,t1209,t1211,t1212,t1213,t1214,t1215,t1223,t123,t1232,t1234,t1235,t1236,t1237,t124,t1242,t1245,t1246,t1247,t1249,t125,t1250,t1251,t1252,t1253,t1255,t1256,t1257,t126,t1260,t1261,t1262,t1263,t1264,t1265,t1268,t1270,t1272,t1275,t1277,t1281,t1283,t1284,t1285,t1287,t1296,t130,t1301,t1302,t1304,t1305,t1307,t1308,t1309,t1311,t1312,t1313,t1319,t1320,t1322,t1323,t1324,t1328,t1329,t1330,t1331,t1332,t1333,t1334,t1337,t1338,t134,t1341,t1342,t1343,t1344,t1345,t1348,t1354,t1355,t1356,t136,t1365,t1366,t1368,t137,t1370,t1371,t1372,t1373,t1374,t1376,t1377,t1378,t1379,t138,t1380,t1384,t1385,t1391,t1393,t1397,t1399,t1402,t1409,t141,t1410,t1411,t1412,t1415,t1416,t1418,t142,t1420,t1422,t1427,t1429,t1431,t1433,t1434,t1436,t144,t1441,t1442,t1443,t1444,t1446,t1448,t1449,t1450,t1452,t1453,t1454,t1455,t1456,t1457,t1458,t1459,t1460,t1478,t1479,t148,t1481,t1486,t1489,t149,t1491,t1492,t1495,t1499,t15,t1500,t1506,t1507,t1509,t1514,t1517,t1518,t152,t1521,t1526,t1529,t1531,t1532,t1539,t1542,t1548,t1549,t1550,t1552,t1559,t156,t1562,t1563,t1565,t1567,t1568,t1576,t1582,t1588,t1591,t1593,t1596,t1597,t1598,t160,t1600,t1605,t161,t1610,t1613,t1614,t1615,t1616,t1617,t1618,t1619,t162,t1620,t1632,t1635,t1639,t1640,t1642,t1645,t1647,t1648,t165,t1651,t1653,t1654,t166,t1661,t1663,t1664,t1667,t167,t1670,t1671,t1673,t1674,t1675,t1677,t1684,t1685,t169,t1690,t1691,t1692,t1693,t1700,t1704,t1709,t171,t1712,t1714,t1717,t1718,t1723,t1727,t173,t1733,t1734,t1747,t1749,t1761,t1762,t1765,t1773,t1775,t1784,t1786,t1788,t1791,t1796,t1798,t1799,t1803,t1805,t1806,t1807,t1808,t1810,t1812,t1814,t1815,t1825,t1829,t184,t1841,t1861,t1865,t1867,t1892,t1906,t1915,t195,t197,t1971,t1973,t1974,t1975,t198,t2,t2043,t2053,t2062,t2066,t2067,t2087,t213,t214,t2141,t2172,t22,t2238,t2245,t225,t23,t2324,t2326,t2339,t24,t241,t242,t243,t244,t245,t246,t2479,t2485,t25,t2505,t251,t2512,t252,t253,t2531,t255,t256,t257,t2581,t259,t2597,t26,t260,t261,t2617,t262,t263,t264,t266,t2660,t267,t269,t2692,t2698,t2699,t27,t2704,t271,t273,t274,t2742,t275,t276,t277,t2783,t2784,t28,t2804,t2819,t283,t2839,t284,t2842,t2844,t285,t2857,t286,t287,t2872,t2874,t2875,t2879,t288,t289,t290,t291,t2912,t2913,t292,t293,t294,t2946,t295,t2951,t296,t297,t2977,t298,t299,t3,t30,t300,t301,t3017,t3019,t302,t3022,t3023,t3025,t3028,t303,t3030,t304,t3109,t3202,t3209,t324,t3260,t3264,t33,t338,t34,t342,t345,t346,t347,t348,t35,t351,t352,t353,t354,t355,t356,t357,t358,t359,t360,t370,t375,t376,t377,t38,t380,t381,t382,t383,t390,t391,t392,t3932,t394,t3944,t3955,t396,t3965,t397,t398,t3982,t399,t3998,t4,t40,t400,t4003,t4008,t401,t4014,t4033,t4038,t41,t410,t411,t412,t413,t414,t415,t418,t419,t420,t421,t424,t425,t426,t428,t429,t430,t431,t433,t434,t436,t437,t438,t44,t445,t447,t448,t45,t450,t451,t453,t454,t456,t459,t4597,t46,t460,t4603,t462,t463,t464,t465,t466,t467,t470,t471,t472,t473,t474,t475,t476,t477,t478,t479,t48,t480,t482,t483,t484,t485,t486,t487,t488,t489,t49,t490,t491,t494,t495,t496,t497,t499,t5,t50,t501,t502,t504,t505,t506,t507,t508,t509,t51,t510,t511,t512,t514,t516,t518,t519,t52,t521,t522,t523,t524,t527,t529,t530,t532,t533,t534,t536,t537,t539,t54,t540,t541,t542,t544,t545,t546,t547,t549,t55,t550,t552,t553,t555,t557,t558,t559,t56,t560,t561,t562,t563,t565,t568,t569,t57,t570,t571,t572,t573,t574,t575,t576,t577,t578,t579,t580,t581,t582,t583,t584,t587,t59,t590,t592,t594,t595,t597,t598,t599,t6,t600,t601,t602,t603,t604,t605,t607,t608,t61,t610,t611,t613,t614,t616,t617,t618,t619,t620,t623,t624,t627,t628,t629,t630,t631,t632,t633,t634,t635,t636,t637,t638,t639,t640,t641,t642,t643,t645,t647,t648,t65,t650,t651,t655,t657,t662,t663,t664,t665,t666,t667,t668,t669,t671,t672,t673,t674,t675,t676,t68,t681,t684,t685,t686,t687,t688,t689,t69,t690,t691,t692,t693,t694,t695,t699,t7,t701,t703,t704,t705,t706,t707,t708,t709,t71,t710,t711,t712,t713,t714,t715,t716,t717,t718,t719,t720,t721,t722,t723,t724,t725,t726,t727,t728,t729,t73,t730,t733,t734,t735,t736,t737,t738,t739,t740,t741,t742,t743,t744,t746,t749,t750,t751,t752,t753,t754,t755,t756,t757,t759,t760,t761,t762,t764,t765,t768,t769,t771,t772,t773,t774,t775,t776,t777,t778,t779,t780,t781,t782,t783,t784,t785,t786,t787,t788,t789,t790,t791,t792,t794,t795,t796,t797,t798,t799,t8,t800,t801,t802,t803,t804,t805,t806,t807,t808,t809,t810,t811,t812,t813,t814,t815,t816,t817,t818,t819,t820,t821,t822,t825,t826,t827,t828,t829,t830,t831,t832,t833,t834,t835,t836,t837,t838,t839,t841,t842,t843,t844,t845,t846,t847,t848,t850,t851,t852,t853,t854,t855,t856,t857,t860,t861,t864,t865,t867,t868,t869,t870,t871,t872,t873,t874,t875,t876,t885,t886,t887,t888,t889,t890,t891,t892,t893,t894,t895,t896,t897,t898,t9,t900,t901,t902,t903,t904,t906,t907,t914,t915,t916,t917,t918,t919,t920,t921,t922,t923,t924,t925,t926,t927,t928,t931,t932,t933,t934,t935,t936,t937,t938,t939,t940,t941,t942,t943,t944,t945,t947,t948,t949,t950,t951,t952,t953,t955,t957,t958,t959,t960,t961,t962,t963,t966,t968,t969,t971,t972,t973,t975,t978,t979,t980,t981,t983,t985,t986,t987,t988,t989,t990,t991,t992,t993,t994,t995,t996,t997,t998,t999});
end
function C = ft_3(ct)
B_cg_H = ct{1};
ITail = ct{2};
Mb = ct{3};
Mm = ct{4};
Mt = ct{5};
T_cg_H = ct{6};
dphi1 = ct{7};
dphi2 = ct{8};
dpsi1 = ct{9};
dth1 = ct{10};
dth2 = ct{11};
dx = ct{12};
dy = ct{13};
dz = ct{14};
t10 = ct{15};
t100 = ct{16};
t1000 = ct{17};
t1001 = ct{18};
t1002 = ct{19};
t1003 = ct{20};
t1004 = ct{21};
t1005 = ct{22};
t1006 = ct{23};
t1007 = ct{24};
t1008 = ct{25};
t1009 = ct{26};
t1010 = ct{27};
t1011 = ct{28};
t1012 = ct{29};
t1013 = ct{30};
t1014 = ct{31};
t1016 = ct{32};
t1017 = ct{33};
t1018 = ct{34};
t1019 = ct{35};
t1020 = ct{36};
t1022 = ct{37};
t1026 = ct{38};
t1028 = ct{39};
t103 = ct{40};
t1031 = ct{41};
t1036 = ct{42};
t1037 = ct{43};
t1040 = ct{44};
t1043 = ct{45};
t1044 = ct{46};
t1045 = ct{47};
t1047 = ct{48};
t105 = ct{49};
t1050 = ct{50};
t1051 = ct{51};
t1052 = ct{52};
t1053 = ct{53};
t1054 = ct{54};
t1055 = ct{55};
t1056 = ct{56};
t1057 = ct{57};
t1059 = ct{58};
t1060 = ct{59};
t1061 = ct{60};
t1062 = ct{61};
t1063 = ct{62};
t1064 = ct{63};
t1065 = ct{64};
t1067 = ct{65};
t1071 = ct{66};
t1072 = ct{67};
t1074 = ct{68};
t1075 = ct{69};
t1076 = ct{70};
t1077 = ct{71};
t1078 = ct{72};
t1079 = ct{73};
t1080 = ct{74};
t1081 = ct{75};
t1082 = ct{76};
t1083 = ct{77};
t1084 = ct{78};
t1085 = ct{79};
t1086 = ct{80};
t1087 = ct{81};
t1088 = ct{82};
t1089 = ct{83};
t1090 = ct{84};
t1091 = ct{85};
t1092 = ct{86};
t1093 = ct{87};
t1094 = ct{88};
t1096 = ct{89};
t1097 = ct{90};
t1098 = ct{91};
t11 = ct{92};
t1100 = ct{93};
t1101 = ct{94};
t1102 = ct{95};
t1103 = ct{96};
t1104 = ct{97};
t1105 = ct{98};
t1106 = ct{99};
t1108 = ct{100};
t1109 = ct{101};
t1110 = ct{102};
t1111 = ct{103};
t1112 = ct{104};
t1113 = ct{105};
t1116 = ct{106};
t1120 = ct{107};
t1121 = ct{108};
t1122 = ct{109};
t1123 = ct{110};
t1124 = ct{111};
t1126 = ct{112};
t1127 = ct{113};
t1128 = ct{114};
t1129 = ct{115};
t1130 = ct{116};
t1131 = ct{117};
t1134 = ct{118};
t1136 = ct{119};
t1137 = ct{120};
t1138 = ct{121};
t1139 = ct{122};
t1140 = ct{123};
t1141 = ct{124};
t1142 = ct{125};
t1143 = ct{126};
t1145 = ct{127};
t1146 = ct{128};
t1147 = ct{129};
t1149 = ct{130};
t115 = ct{131};
t1152 = ct{132};
t1153 = ct{133};
t1154 = ct{134};
t1158 = ct{135};
t1159 = ct{136};
t116 = ct{137};
t1160 = ct{138};
t1161 = ct{139};
t1164 = ct{140};
t1165 = ct{141};
t1166 = ct{142};
t1169 = ct{143};
t1170 = ct{144};
t1172 = ct{145};
t1173 = ct{146};
t1174 = ct{147};
t1176 = ct{148};
t1177 = ct{149};
t1179 = ct{150};
t1181 = ct{151};
t1182 = ct{152};
t1183 = ct{153};
t1185 = ct{154};
t1186 = ct{155};
t1187 = ct{156};
t1188 = ct{157};
t1189 = ct{158};
t119 = ct{159};
t1190 = ct{160};
t1191 = ct{161};
t1192 = ct{162};
t1193 = ct{163};
t1194 = ct{164};
t1196 = ct{165};
t1198 = ct{166};
t1199 = ct{167};
t120 = ct{168};
t1200 = ct{169};
t1201 = ct{170};
t1203 = ct{171};
t1205 = ct{172};
t1206 = ct{173};
t1209 = ct{174};
t1211 = ct{175};
t1212 = ct{176};
t1213 = ct{177};
t1214 = ct{178};
t1215 = ct{179};
t1223 = ct{180};
t123 = ct{181};
t1232 = ct{182};
t1234 = ct{183};
t1235 = ct{184};
t1236 = ct{185};
t1237 = ct{186};
t124 = ct{187};
t1242 = ct{188};
t1245 = ct{189};
t1246 = ct{190};
t1247 = ct{191};
t1249 = ct{192};
t125 = ct{193};
t1250 = ct{194};
t1251 = ct{195};
t1252 = ct{196};
t1253 = ct{197};
t1255 = ct{198};
t1256 = ct{199};
t1257 = ct{200};
t126 = ct{201};
t1260 = ct{202};
t1261 = ct{203};
t1262 = ct{204};
t1263 = ct{205};
t1264 = ct{206};
t1265 = ct{207};
t1268 = ct{208};
t1270 = ct{209};
t1272 = ct{210};
t1275 = ct{211};
t1277 = ct{212};
t1281 = ct{213};
t1283 = ct{214};
t1284 = ct{215};
t1285 = ct{216};
t1287 = ct{217};
t1296 = ct{218};
t130 = ct{219};
t1301 = ct{220};
t1302 = ct{221};
t1304 = ct{222};
t1305 = ct{223};
t1307 = ct{224};
t1308 = ct{225};
t1309 = ct{226};
t1311 = ct{227};
t1312 = ct{228};
t1313 = ct{229};
t1319 = ct{230};
t1320 = ct{231};
t1322 = ct{232};
t1323 = ct{233};
t1324 = ct{234};
t1328 = ct{235};
t1329 = ct{236};
t1330 = ct{237};
t1331 = ct{238};
t1332 = ct{239};
t1333 = ct{240};
t1334 = ct{241};
t1337 = ct{242};
t1338 = ct{243};
t134 = ct{244};
t1341 = ct{245};
t1342 = ct{246};
t1343 = ct{247};
t1344 = ct{248};
t1345 = ct{249};
t1348 = ct{250};
t1354 = ct{251};
t1355 = ct{252};
t1356 = ct{253};
t136 = ct{254};
t1365 = ct{255};
t1366 = ct{256};
t1368 = ct{257};
t137 = ct{258};
t1370 = ct{259};
t1371 = ct{260};
t1372 = ct{261};
t1373 = ct{262};
t1374 = ct{263};
t1376 = ct{264};
t1377 = ct{265};
t1378 = ct{266};
t1379 = ct{267};
t138 = ct{268};
t1380 = ct{269};
t1384 = ct{270};
t1385 = ct{271};
t1391 = ct{272};
t1393 = ct{273};
t1397 = ct{274};
t1399 = ct{275};
t1402 = ct{276};
t1409 = ct{277};
t141 = ct{278};
t1410 = ct{279};
t1411 = ct{280};
t1412 = ct{281};
t1415 = ct{282};
t1416 = ct{283};
t1418 = ct{284};
t142 = ct{285};
t1420 = ct{286};
t1422 = ct{287};
t1427 = ct{288};
t1429 = ct{289};
t1431 = ct{290};
t1433 = ct{291};
t1434 = ct{292};
t1436 = ct{293};
t144 = ct{294};
t1441 = ct{295};
t1442 = ct{296};
t1443 = ct{297};
t1444 = ct{298};
t1446 = ct{299};
t1448 = ct{300};
t1449 = ct{301};
t1450 = ct{302};
t1452 = ct{303};
t1453 = ct{304};
t1454 = ct{305};
t1455 = ct{306};
t1456 = ct{307};
t1457 = ct{308};
t1458 = ct{309};
t1459 = ct{310};
t1460 = ct{311};
t1478 = ct{312};
t1479 = ct{313};
t148 = ct{314};
t1481 = ct{315};
t1486 = ct{316};
t1489 = ct{317};
t149 = ct{318};
t1491 = ct{319};
t1492 = ct{320};
t1495 = ct{321};
t1499 = ct{322};
t15 = ct{323};
t1500 = ct{324};
t1506 = ct{325};
t1507 = ct{326};
t1509 = ct{327};
t1514 = ct{328};
t1517 = ct{329};
t1518 = ct{330};
t152 = ct{331};
t1521 = ct{332};
t1526 = ct{333};
t1529 = ct{334};
t1531 = ct{335};
t1532 = ct{336};
t1539 = ct{337};
t1542 = ct{338};
t1548 = ct{339};
t1549 = ct{340};
t1550 = ct{341};
t1552 = ct{342};
t1559 = ct{343};
t156 = ct{344};
t1562 = ct{345};
t1563 = ct{346};
t1565 = ct{347};
t1567 = ct{348};
t1568 = ct{349};
t1576 = ct{350};
t1582 = ct{351};
t1588 = ct{352};
t1591 = ct{353};
t1593 = ct{354};
t1596 = ct{355};
t1597 = ct{356};
t1598 = ct{357};
t160 = ct{358};
t1600 = ct{359};
t1605 = ct{360};
t161 = ct{361};
t1610 = ct{362};
t1613 = ct{363};
t1614 = ct{364};
t1615 = ct{365};
t1616 = ct{366};
t1617 = ct{367};
t1618 = ct{368};
t1619 = ct{369};
t162 = ct{370};
t1620 = ct{371};
t1632 = ct{372};
t1635 = ct{373};
t1639 = ct{374};
t1640 = ct{375};
t1642 = ct{376};
t1645 = ct{377};
t1647 = ct{378};
t1648 = ct{379};
t165 = ct{380};
t1651 = ct{381};
t1653 = ct{382};
t1654 = ct{383};
t166 = ct{384};
t1661 = ct{385};
t1663 = ct{386};
t1664 = ct{387};
t1667 = ct{388};
t167 = ct{389};
t1670 = ct{390};
t1671 = ct{391};
t1673 = ct{392};
t1674 = ct{393};
t1675 = ct{394};
t1677 = ct{395};
t1684 = ct{396};
t1685 = ct{397};
t169 = ct{398};
t1690 = ct{399};
t1691 = ct{400};
t1692 = ct{401};
t1693 = ct{402};
t1700 = ct{403};
t1704 = ct{404};
t1709 = ct{405};
t171 = ct{406};
t1712 = ct{407};
t1714 = ct{408};
t1717 = ct{409};
t1718 = ct{410};
t1723 = ct{411};
t1727 = ct{412};
t173 = ct{413};
t1733 = ct{414};
t1734 = ct{415};
t1747 = ct{416};
t1749 = ct{417};
t1761 = ct{418};
t1762 = ct{419};
t1765 = ct{420};
t1773 = ct{421};
t1775 = ct{422};
t1784 = ct{423};
t1786 = ct{424};
t1788 = ct{425};
t1791 = ct{426};
t1796 = ct{427};
t1798 = ct{428};
t1799 = ct{429};
t1803 = ct{430};
t1805 = ct{431};
t1806 = ct{432};
t1807 = ct{433};
t1808 = ct{434};
t1810 = ct{435};
t1812 = ct{436};
t1814 = ct{437};
t1815 = ct{438};
t1825 = ct{439};
t1829 = ct{440};
t184 = ct{441};
t1841 = ct{442};
t1861 = ct{443};
t1865 = ct{444};
t1867 = ct{445};
t1892 = ct{446};
t1906 = ct{447};
t1915 = ct{448};
t195 = ct{449};
t197 = ct{450};
t1971 = ct{451};
t1973 = ct{452};
t1974 = ct{453};
t1975 = ct{454};
t198 = ct{455};
t2 = ct{456};
t2043 = ct{457};
t2053 = ct{458};
t2062 = ct{459};
t2066 = ct{460};
t2067 = ct{461};
t2087 = ct{462};
t213 = ct{463};
t214 = ct{464};
t2141 = ct{465};
t2172 = ct{466};
t22 = ct{467};
t2238 = ct{468};
t2245 = ct{469};
t225 = ct{470};
t23 = ct{471};
t2324 = ct{472};
t2326 = ct{473};
t2339 = ct{474};
t24 = ct{475};
t241 = ct{476};
t242 = ct{477};
t243 = ct{478};
t244 = ct{479};
t245 = ct{480};
t246 = ct{481};
t2479 = ct{482};
t2485 = ct{483};
t25 = ct{484};
t2505 = ct{485};
t251 = ct{486};
t2512 = ct{487};
t252 = ct{488};
t253 = ct{489};
t2531 = ct{490};
t255 = ct{491};
t256 = ct{492};
t257 = ct{493};
t2581 = ct{494};
t259 = ct{495};
t2597 = ct{496};
t26 = ct{497};
t260 = ct{498};
t261 = ct{499};
t2617 = ct{500};
t262 = ct{501};
t263 = ct{502};
t264 = ct{503};
t266 = ct{504};
t2660 = ct{505};
t267 = ct{506};
t269 = ct{507};
t2692 = ct{508};
t2698 = ct{509};
t2699 = ct{510};
t27 = ct{511};
t2704 = ct{512};
t271 = ct{513};
t273 = ct{514};
t274 = ct{515};
t2742 = ct{516};
t275 = ct{517};
t276 = ct{518};
t277 = ct{519};
t2783 = ct{520};
t2784 = ct{521};
t28 = ct{522};
t2804 = ct{523};
t2819 = ct{524};
t283 = ct{525};
t2839 = ct{526};
t284 = ct{527};
t2842 = ct{528};
t2844 = ct{529};
t285 = ct{530};
t2857 = ct{531};
t286 = ct{532};
t287 = ct{533};
t2872 = ct{534};
t2874 = ct{535};
t2875 = ct{536};
t2879 = ct{537};
t288 = ct{538};
t289 = ct{539};
t290 = ct{540};
t291 = ct{541};
t2912 = ct{542};
t2913 = ct{543};
t292 = ct{544};
t293 = ct{545};
t294 = ct{546};
t2946 = ct{547};
t295 = ct{548};
t2951 = ct{549};
t296 = ct{550};
t297 = ct{551};
t2977 = ct{552};
t298 = ct{553};
t299 = ct{554};
t3 = ct{555};
t30 = ct{556};
t300 = ct{557};
t301 = ct{558};
t3017 = ct{559};
t3019 = ct{560};
t302 = ct{561};
t3022 = ct{562};
t3023 = ct{563};
t3025 = ct{564};
t3028 = ct{565};
t303 = ct{566};
t3030 = ct{567};
t304 = ct{568};
t3109 = ct{569};
t3202 = ct{570};
t3209 = ct{571};
t324 = ct{572};
t3260 = ct{573};
t3264 = ct{574};
t33 = ct{575};
t338 = ct{576};
t34 = ct{577};
t342 = ct{578};
t345 = ct{579};
t346 = ct{580};
t347 = ct{581};
t348 = ct{582};
t35 = ct{583};
t351 = ct{584};
t352 = ct{585};
t353 = ct{586};
t354 = ct{587};
t355 = ct{588};
t356 = ct{589};
t357 = ct{590};
t358 = ct{591};
t359 = ct{592};
t360 = ct{593};
t370 = ct{594};
t375 = ct{595};
t376 = ct{596};
t377 = ct{597};
t38 = ct{598};
t380 = ct{599};
t381 = ct{600};
t382 = ct{601};
t383 = ct{602};
t390 = ct{603};
t391 = ct{604};
t392 = ct{605};
t3932 = ct{606};
t394 = ct{607};
t3944 = ct{608};
t3955 = ct{609};
t396 = ct{610};
t3965 = ct{611};
t397 = ct{612};
t398 = ct{613};
t3982 = ct{614};
t399 = ct{615};
t3998 = ct{616};
t4 = ct{617};
t40 = ct{618};
t400 = ct{619};
t4003 = ct{620};
t4008 = ct{621};
t401 = ct{622};
t4014 = ct{623};
t4033 = ct{624};
t4038 = ct{625};
t41 = ct{626};
t410 = ct{627};
t411 = ct{628};
t412 = ct{629};
t413 = ct{630};
t414 = ct{631};
t415 = ct{632};
t418 = ct{633};
t419 = ct{634};
t420 = ct{635};
t421 = ct{636};
t424 = ct{637};
t425 = ct{638};
t426 = ct{639};
t428 = ct{640};
t429 = ct{641};
t430 = ct{642};
t431 = ct{643};
t433 = ct{644};
t434 = ct{645};
t436 = ct{646};
t437 = ct{647};
t438 = ct{648};
t44 = ct{649};
t445 = ct{650};
t447 = ct{651};
t448 = ct{652};
t45 = ct{653};
t450 = ct{654};
t451 = ct{655};
t453 = ct{656};
t454 = ct{657};
t456 = ct{658};
t459 = ct{659};
t4597 = ct{660};
t46 = ct{661};
t460 = ct{662};
t4603 = ct{663};
t462 = ct{664};
t463 = ct{665};
t464 = ct{666};
t465 = ct{667};
t466 = ct{668};
t467 = ct{669};
t470 = ct{670};
t471 = ct{671};
t472 = ct{672};
t473 = ct{673};
t474 = ct{674};
t475 = ct{675};
t476 = ct{676};
t477 = ct{677};
t478 = ct{678};
t479 = ct{679};
t48 = ct{680};
t480 = ct{681};
t482 = ct{682};
t483 = ct{683};
t484 = ct{684};
t485 = ct{685};
t486 = ct{686};
t487 = ct{687};
t488 = ct{688};
t489 = ct{689};
t49 = ct{690};
t490 = ct{691};
t491 = ct{692};
t494 = ct{693};
t495 = ct{694};
t496 = ct{695};
t497 = ct{696};
t499 = ct{697};
t5 = ct{698};
t50 = ct{699};
t501 = ct{700};
t502 = ct{701};
t504 = ct{702};
t505 = ct{703};
t506 = ct{704};
t507 = ct{705};
t508 = ct{706};
t509 = ct{707};
t51 = ct{708};
t510 = ct{709};
t511 = ct{710};
t512 = ct{711};
t514 = ct{712};
t516 = ct{713};
t518 = ct{714};
t519 = ct{715};
t52 = ct{716};
t521 = ct{717};
t522 = ct{718};
t523 = ct{719};
t524 = ct{720};
t527 = ct{721};
t529 = ct{722};
t530 = ct{723};
t532 = ct{724};
t533 = ct{725};
t534 = ct{726};
t536 = ct{727};
t537 = ct{728};
t539 = ct{729};
t54 = ct{730};
t540 = ct{731};
t541 = ct{732};
t542 = ct{733};
t544 = ct{734};
t545 = ct{735};
t546 = ct{736};
t547 = ct{737};
t549 = ct{738};
t55 = ct{739};
t550 = ct{740};
t552 = ct{741};
t553 = ct{742};
t555 = ct{743};
t557 = ct{744};
t558 = ct{745};
t559 = ct{746};
t56 = ct{747};
t560 = ct{748};
t561 = ct{749};
t562 = ct{750};
t563 = ct{751};
t565 = ct{752};
t568 = ct{753};
t569 = ct{754};
t57 = ct{755};
t570 = ct{756};
t571 = ct{757};
t572 = ct{758};
t573 = ct{759};
t574 = ct{760};
t575 = ct{761};
t576 = ct{762};
t577 = ct{763};
t578 = ct{764};
t579 = ct{765};
t580 = ct{766};
t581 = ct{767};
t582 = ct{768};
t583 = ct{769};
t584 = ct{770};
t587 = ct{771};
t59 = ct{772};
t590 = ct{773};
t592 = ct{774};
t594 = ct{775};
t595 = ct{776};
t597 = ct{777};
t598 = ct{778};
t599 = ct{779};
t6 = ct{780};
t600 = ct{781};
t601 = ct{782};
t602 = ct{783};
t603 = ct{784};
t604 = ct{785};
t605 = ct{786};
t607 = ct{787};
t608 = ct{788};
t61 = ct{789};
t610 = ct{790};
t611 = ct{791};
t613 = ct{792};
t614 = ct{793};
t616 = ct{794};
t617 = ct{795};
t618 = ct{796};
t619 = ct{797};
t620 = ct{798};
t623 = ct{799};
t624 = ct{800};
t627 = ct{801};
t628 = ct{802};
t629 = ct{803};
t630 = ct{804};
t631 = ct{805};
t632 = ct{806};
t633 = ct{807};
t634 = ct{808};
t635 = ct{809};
t636 = ct{810};
t637 = ct{811};
t638 = ct{812};
t639 = ct{813};
t640 = ct{814};
t641 = ct{815};
t642 = ct{816};
t643 = ct{817};
t645 = ct{818};
t647 = ct{819};
t648 = ct{820};
t65 = ct{821};
t650 = ct{822};
t651 = ct{823};
t655 = ct{824};
t657 = ct{825};
t662 = ct{826};
t663 = ct{827};
t664 = ct{828};
t665 = ct{829};
t666 = ct{830};
t667 = ct{831};
t668 = ct{832};
t669 = ct{833};
t671 = ct{834};
t672 = ct{835};
t673 = ct{836};
t674 = ct{837};
t675 = ct{838};
t676 = ct{839};
t68 = ct{840};
t681 = ct{841};
t684 = ct{842};
t685 = ct{843};
t686 = ct{844};
t687 = ct{845};
t688 = ct{846};
t689 = ct{847};
t69 = ct{848};
t690 = ct{849};
t691 = ct{850};
t692 = ct{851};
t693 = ct{852};
t694 = ct{853};
t695 = ct{854};
t699 = ct{855};
t7 = ct{856};
t701 = ct{857};
t703 = ct{858};
t704 = ct{859};
t705 = ct{860};
t706 = ct{861};
t707 = ct{862};
t708 = ct{863};
t709 = ct{864};
t71 = ct{865};
t710 = ct{866};
t711 = ct{867};
t712 = ct{868};
t713 = ct{869};
t714 = ct{870};
t715 = ct{871};
t716 = ct{872};
t717 = ct{873};
t718 = ct{874};
t719 = ct{875};
t720 = ct{876};
t721 = ct{877};
t722 = ct{878};
t723 = ct{879};
t724 = ct{880};
t725 = ct{881};
t726 = ct{882};
t727 = ct{883};
t728 = ct{884};
t729 = ct{885};
t73 = ct{886};
t730 = ct{887};
t733 = ct{888};
t734 = ct{889};
t735 = ct{890};
t736 = ct{891};
t737 = ct{892};
t738 = ct{893};
t739 = ct{894};
t740 = ct{895};
t741 = ct{896};
t742 = ct{897};
t743 = ct{898};
t744 = ct{899};
t746 = ct{900};
t749 = ct{901};
t750 = ct{902};
t751 = ct{903};
t752 = ct{904};
t753 = ct{905};
t754 = ct{906};
t755 = ct{907};
t756 = ct{908};
t757 = ct{909};
t759 = ct{910};
t760 = ct{911};
t761 = ct{912};
t762 = ct{913};
t764 = ct{914};
t765 = ct{915};
t768 = ct{916};
t769 = ct{917};
t771 = ct{918};
t772 = ct{919};
t773 = ct{920};
t774 = ct{921};
t775 = ct{922};
t776 = ct{923};
t777 = ct{924};
t778 = ct{925};
t779 = ct{926};
t780 = ct{927};
t781 = ct{928};
t782 = ct{929};
t783 = ct{930};
t784 = ct{931};
t785 = ct{932};
t786 = ct{933};
t787 = ct{934};
t788 = ct{935};
t789 = ct{936};
t790 = ct{937};
t791 = ct{938};
t792 = ct{939};
t794 = ct{940};
t795 = ct{941};
t796 = ct{942};
t797 = ct{943};
t798 = ct{944};
t799 = ct{945};
t8 = ct{946};
t800 = ct{947};
t801 = ct{948};
t802 = ct{949};
t803 = ct{950};
t804 = ct{951};
t805 = ct{952};
t806 = ct{953};
t807 = ct{954};
t808 = ct{955};
t809 = ct{956};
t810 = ct{957};
t811 = ct{958};
t812 = ct{959};
t813 = ct{960};
t814 = ct{961};
t815 = ct{962};
t816 = ct{963};
t817 = ct{964};
t818 = ct{965};
t819 = ct{966};
t820 = ct{967};
t821 = ct{968};
t822 = ct{969};
t825 = ct{970};
t826 = ct{971};
t827 = ct{972};
t828 = ct{973};
t829 = ct{974};
t830 = ct{975};
t831 = ct{976};
t832 = ct{977};
t833 = ct{978};
t834 = ct{979};
t835 = ct{980};
t836 = ct{981};
t837 = ct{982};
t838 = ct{983};
t839 = ct{984};
t841 = ct{985};
t842 = ct{986};
t843 = ct{987};
t844 = ct{988};
t845 = ct{989};
t846 = ct{990};
t847 = ct{991};
t848 = ct{992};
t850 = ct{993};
t851 = ct{994};
t852 = ct{995};
t853 = ct{996};
t854 = ct{997};
t855 = ct{998};
t856 = ct{999};
t857 = ct{1000};
t860 = ct{1001};
t861 = ct{1002};
t864 = ct{1003};
t865 = ct{1004};
t867 = ct{1005};
t868 = ct{1006};
t869 = ct{1007};
t870 = ct{1008};
t871 = ct{1009};
t872 = ct{1010};
t873 = ct{1011};
t874 = ct{1012};
t875 = ct{1013};
t876 = ct{1014};
t885 = ct{1015};
t886 = ct{1016};
t887 = ct{1017};
t888 = ct{1018};
t889 = ct{1019};
t890 = ct{1020};
t891 = ct{1021};
t892 = ct{1022};
t893 = ct{1023};
t894 = ct{1024};
t895 = ct{1025};
t896 = ct{1026};
t897 = ct{1027};
t898 = ct{1028};
t9 = ct{1029};
t900 = ct{1030};
t901 = ct{1031};
t902 = ct{1032};
t903 = ct{1033};
t904 = ct{1034};
t906 = ct{1035};
t907 = ct{1036};
t914 = ct{1037};
t915 = ct{1038};
t916 = ct{1039};
t917 = ct{1040};
t918 = ct{1041};
t919 = ct{1042};
t920 = ct{1043};
t921 = ct{1044};
t922 = ct{1045};
t923 = ct{1046};
t924 = ct{1047};
t925 = ct{1048};
t926 = ct{1049};
t927 = ct{1050};
t928 = ct{1051};
t931 = ct{1052};
t932 = ct{1053};
t933 = ct{1054};
t934 = ct{1055};
t935 = ct{1056};
t936 = ct{1057};
t937 = ct{1058};
t938 = ct{1059};
t939 = ct{1060};
t940 = ct{1061};
t941 = ct{1062};
t942 = ct{1063};
t943 = ct{1064};
t944 = ct{1065};
t945 = ct{1066};
t947 = ct{1067};
t948 = ct{1068};
t949 = ct{1069};
t950 = ct{1070};
t951 = ct{1071};
t952 = ct{1072};
t953 = ct{1073};
t955 = ct{1074};
t957 = ct{1075};
t958 = ct{1076};
t959 = ct{1077};
t960 = ct{1078};
t961 = ct{1079};
t962 = ct{1080};
t963 = ct{1081};
t966 = ct{1082};
t968 = ct{1083};
t969 = ct{1084};
t971 = ct{1085};
t972 = ct{1086};
t973 = ct{1087};
t975 = ct{1088};
t978 = ct{1089};
t979 = ct{1090};
t980 = ct{1091};
t981 = ct{1092};
t983 = ct{1093};
t985 = ct{1094};
t986 = ct{1095};
t987 = ct{1096};
t988 = ct{1097};
t989 = ct{1098};
t990 = ct{1099};
t991 = ct{1100};
t992 = ct{1101};
t993 = ct{1102};
t994 = ct{1103};
t995 = ct{1104};
t996 = ct{1105};
t997 = ct{1106};
t998 = ct{1107};
t999 = ct{1108};
t1832 = t4.*t868.*(t103-t544);
t1836 = -t1799;
t1837 = t1775./2.0;
t1838 = -t1807;
t1839 = -t1806;
t1844 = t487.*(t534-t546).*(-1.0./2.0);
t1856 = t3.*t872.*(t103-t544).*(-1.0./2.0);
t1862 = -t1037.*(t103-t544);
t1866 = t9.*t871.*(t197-t537);
t1868 = t9.*t871.*t1044;
t1871 = t8.*t873.*t1044;
t1874 = -t1861;
t1876 = t4.*t871.*t1031;
t1879 = t8.*t872.*t1031;
t1881 = t1031.*(t105-t465).*(-1.0./2.0);
t1884 = t1037.*(t105-t465).*(-1.0./2.0);
t1888 = t993.*6.73108e-3;
t1889 = t994.*6.73108e-3;
t1894 = t8.*t873.*(t197-t537).*(-1.0./2.0);
t1895 = t1047.*(t105-t465).*(-1.0./2.0);
t1899 = t867.*3.367829185e-3;
t1905 = t986.*3.36554e-3;
t1907 = t988.*3.36554e-3;
t1908 = t989.*3.36554e-3;
t1909 = t990.*3.36554e-3;
t1910 = t991.*3.36554e-3;
t1914 = -t1892;
t1922 = t1037.*(t103-t544).*(-1.0./2.0);
t1928 = t867.*8.56645e-6;
t1941 = -t1915;
t1962 = t1052.*3.36554e-3;
t1963 = t1053.*3.36554e-3;
t1964 = t1059.*3.36554e-3;
t1965 = t1060.*3.36554e-3;
t1969 = t1062.*3.36554e-3;
t1970 = t1063.*3.36554e-3;
t1972 = t1064.*3.36554e-3;
t1979 = Mb.*t15.*(t197-t537).*(t214-t541);
t1981 = t22+t148+t855+t931;
t1982 = t1079.*3.36554e-3;
t1983 = t1080.*3.36554e-3;
t1989 = (t105-t465).*(t534-t546);
t2008 = t871.*t1198;
t2042 = t986.*3.372786875e-3;
t2044 = t988.*3.372786875e-3;
t2045 = t989.*3.372786875e-3;
t2046 = t990.*3.372786875e-3;
t2047 = t991.*3.372786875e-3;
t2050 = t993.*6.74557375e-3;
t2051 = t994.*6.74557375e-3;
t2052 = t986.*9.53094055e-4;
t2054 = t988.*9.53094055e-4;
t2055 = t989.*9.53094055e-4;
t2056 = t990.*9.53094055e-4;
t2057 = t991.*9.53094055e-4;
t2058 = t993.*1.90618811e-3;
t2059 = t994.*1.90618811e-3;
t2064 = t1129.*3.36554e-3;
t2068 = -Mb.*t15.*t1047.*(t197-t537);
t2071 = t1137.*3.36554e-3;
t2072 = t1138.*3.36554e-3;
t2078 = -t8.*t872.*(t534-t546);
t2102 = -t2067;
t2104 = t871.*t1281;
t2120 = -t4.*t871.*(t534-t546);
t2121 = (t103-t544).*(t534-t546);
t2130 = t1079.*3.372786875e-3;
t2131 = t1080.*3.372786875e-3;
t2134 = t1079.*9.53094055e-4;
t2135 = t1080.*9.53094055e-4;
t2144 = t1062.*3.372786875e-3;
t2145 = t1063.*3.372786875e-3;
t2146 = t1062.*9.53094055e-4;
t2147 = t1063.*9.53094055e-4;
t2150 = t1052.*3.367829185e-3;
t2151 = t1053.*3.367829185e-3;
t2152 = t1176.*3.36554e-3;
t2154 = t1177.*3.36554e-3;
t2155 = t1059.*3.367829185e-3;
t2156 = t1060.*3.367829185e-3;
t2158 = t1063.*3.367829185e-3;
t2159 = t1064.*3.367829185e-3;
t2161 = Mb.*t15.*t1047.*(t197-t537);
t2176 = -t2141;
t2201 = t1052.*8.56645e-6;
t2202 = t1053.*8.56645e-6;
t2203 = t391+t398+t429+t938;
t2205 = t8.*t872.*(t534-t546).*(-1.0./2.0);
t2207 = t1059.*8.56645e-6;
t2208 = t1060.*8.56645e-6;
t2211 = -t2172;
t2214 = t1063.*8.56645e-6;
t2218 = t1064.*8.56645e-6;
t2226 = t1137.*3.367829185e-3;
t2227 = t1138.*3.367829185e-3;
t2237 = t1129.*9.52624335e-4;
t2242 = t1129.*3.372816795e-3;
t2246 = t4.*t871.*(t534-t546).*(-1.0./2.0);
t2251 = t1261.*3.36554e-3;
t2252 = t1262.*3.36554e-3;
t2253 = t1263.*3.36554e-3;
t2256 = t1249.*3.36554e-3;
t2257 = t1250.*3.36554e-3;
t2261 = t353+t598+t599+t734;
t2273 = Mt.*t10.*t2087;
t2302 = t1176.*9.52624335e-4;
t2303 = t1177.*9.52624335e-4;
t2305 = t1176.*3.372816795e-3;
t2307 = t1177.*3.372816795e-3;
t2311 = t1137.*8.56645e-6;
t2312 = t1138.*8.56645e-6;
t2320 = t1328.*3.36554e-3;
t2321 = t1329.*3.36554e-3;
t2322 = t1330.*3.36554e-3;
t2323 = t1331.*3.36554e-3;
t2328 = Mt.*t2.*t5.*t2087;
t2331 = Mt.*t5.*t7.*t2087;
t2337 = t1319.*3.36554e-3;
t2350 = -t2324;
t2351 = -t2326;
t2360 = t40+t396+t462+t595+t681;
t2363 = -t2339;
t2384 = t156+t264+t275+t394+t445+t614;
t2385 = t1262.*3.372786875e-3;
t2386 = t1263.*3.372786875e-3;
t2388 = t1262.*9.53094055e-4;
t2389 = t1263.*9.53094055e-4;
t2392 = t1261.*3.367829185e-3;
t2393 = t1263.*3.367829185e-3;
t2398 = t1249.*3.367829185e-3;
t2399 = t1250.*3.367829185e-3;
t2405 = t149+t255+t269+t390+t430+t587;
t2411 = t1379.*3.36554e-3;
t2412 = t1380.*3.36554e-3;
t2420 = Mt.*t876.*t1531;
t2461 = t1328.*3.372786875e-3;
t2462 = t1329.*3.372786875e-3;
t2463 = t1330.*3.372786875e-3;
t2464 = t1331.*3.372786875e-3;
t2466 = t1328.*9.53094055e-4;
t2467 = t1329.*9.53094055e-4;
t2468 = t1330.*9.53094055e-4;
t2469 = t1331.*9.53094055e-4;
t2477 = dphi1.*(-t44+t390+t430-t524+t587);
t2478 = t1507.*(-3.36554e-3);
t2480 = t1329.*3.367829185e-3;
t2481 = t1331.*3.367829185e-3;
t2489 = t1442.*3.36554e-3;
t2490 = t1443.*3.36554e-3;
t2491 = t11.*t542.*(t105-t465).*(-3.36554e-3);
t2492 = t1446.*3.36554e-3;
t2503 = t1319.*9.52624335e-4;
t2510 = t1319.*3.372816795e-3;
t2514 = t1261.*8.56645e-6;
t2515 = t1263.*8.56645e-6;
t2517 = t1249.*8.56645e-6;
t2518 = t1250.*8.56645e-6;
t2530 = t1507.*3.36554e-3;
t2546 = t11.*t542.*(t105-t465).*3.36554e-3;
t2562 = -t2512;
t2570 = Mt.*t5.*(-t44+t390+t430-t524+t587);
t2572 = t1582.*(-3.36554e-3);
t2577 = t496.*(t214-t541).*(-3.36554e-3);
t2584 = t11.*t420.*(t214-t541).*(-3.36554e-3);
t2589 = Mt.*t10.*(-t51+t394+t445-t527+t614);
t2615 = t1379.*9.52624335e-4;
t2616 = t1380.*9.52624335e-4;
t2620 = t1329.*8.56645e-6;
t2621 = t1331.*8.56645e-6;
t2624 = t1379.*3.372816795e-3;
t2625 = t1380.*3.372816795e-3;
t2632 = t1582.*3.36554e-3;
t2668 = Mt.*t2.*t10.*(-t44+t390+t430-t524+t587);
t2670 = Mt.*t7.*t10.*(-t44+t390+t430-t524+t587);
t2681 = Mt.*t2.*t5.*(-t51+t394+t445-t527+t614);
t2686 = Mt.*t5.*t7.*(-t51+t394+t445-t527+t614);
t2690 = t1507.*(-3.372786875e-3);
t2697 = t1507.*(-9.53094055e-4);
t2706 = t1442.*9.52624335e-4;
t2707 = t1443.*9.52624335e-4;
t2709 = t11.*t542.*(t105-t465).*(-3.372786875e-3);
t2710 = t1446.*3.372786875e-3;
t2715 = t1442.*3.372816795e-3;
t2716 = t1443.*3.372816795e-3;
t2717 = t11.*t542.*(t105-t465).*(-9.53094055e-4);
t2718 = t1446.*9.53094055e-4;
t2740 = t1507.*3.372786875e-3;
t2745 = t1507.*9.53094055e-4;
t2751 = t11.*t542.*(t105-t465).*3.372786875e-3;
t2752 = t1616.*3.36554e-3;
t2753 = t1617.*3.36554e-3;
t2765 = t11.*t420.*(t214-t541).*(-3.367829185e-3);
t2773 = t1582.*(-3.372786875e-3);
t2777 = t1582.*(-9.53094055e-4);
t2788 = t496.*(t214-t541).*(-3.367829185e-3);
t2802 = t1582.*3.372786875e-3;
t2807 = t1582.*9.53094055e-4;
t2821 = t1661.*3.36554e-3;
t2828 = t496.*(t214-t541).*(-8.56645e-6);
t2835 = t11.*t420.*(t214-t541).*(-8.56645e-6);
t2854 = t817.*(t214-t541).*(-3.36554e-3);
t2859 = t11.*t381.*(t534-t546).*(-3.36554e-3);
t2870 = t9.*t868.*(t105-t465).*(-3.36554e-3);
t2873 = t1775.*(-3.36554e-3);
t2883 = t1616.*9.52624335e-4;
t2884 = t1617.*9.52624335e-4;
t2890 = t1616.*3.372816795e-3;
t2891 = t1617.*3.372816795e-3;
t2896 = t817.*(t214-t541).*3.36554e-3;
t2909 = t1775.*3.36554e-3;
t2918 = t487.*(t534-t546).*(-3.36554e-3);
t2938 = t3.*t872.*(t103-t544).*(-3.36554e-3);
t2974 = t257+t338+t345+t425+t519+t765;
t2980 = t267+t342+t351+t436+t523+t769;
t2982 = t1031.*(t105-t465).*(-3.36554e-3);
t2984 = t1037.*(t105-t465).*(-3.36554e-3);
t2992 = t8.*t873.*(t197-t537).*(-3.36554e-3);
t2993 = t475+t476+t943+t944;
t2995 = t1047.*(t105-t465).*(-3.36554e-3);
t3004 = t11.*t381.*(t534-t546).*(-3.372786875e-3);
t3010 = t11.*t381.*(t534-t546).*(-9.53094055e-4);
t3011 = t9.*t868.*(t105-t465).*(-3.372786875e-3);
t3018 = t1775.*(-3.372786875e-3);
t3020 = t9.*t868.*(t105-t465).*(-9.53094055e-4);
t3024 = t1775.*(-9.53094055e-4);
t3029 = t817.*(t214-t541).*(-3.367829185e-3);
t3035 = t1037.*(t105-t465).*3.36554e-3;
t3047 = t1775.*3.372786875e-3;
t3048 = t1775.*9.53094055e-4;
t3051 = t817.*(t214-t541).*3.367829185e-3;
t3056 = t1037.*(t103-t544).*(-3.36554e-3);
t3059 = t817.*(t214-t541).*(-8.56645e-6);
t3060 = t487.*(t534-t546).*(-3.372786875e-3);
t3065 = t487.*(t534-t546).*(-9.53094055e-4);
t3078 = t3.*t872.*(t103-t544).*(-3.372786875e-3);
t3081 = t3.*t872.*(t103-t544).*(-9.53094055e-4);
t3090 = t1037.*(t103-t544).*3.36554e-3;
t3117 = t1031.*(t105-t465).*(-3.372786875e-3);
t3124 = t1031.*(t105-t465).*(-9.53094055e-4);
t3130 = t8.*t873.*(t197-t537).*(-9.52624335e-4);
t3134 = t1047.*(t105-t465).*(-3.372786875e-3);
t3135 = t8.*t873.*(t197-t537).*(-3.372816795e-3);
t3136 = t1047.*(t105-t465).*(-9.53094055e-4);
t3137 = t1037.*(t105-t465).*(-3.367829185e-3);
t3144 = t597+t601+t943+t944;
t3170 = Mt.*t5.*t9.*(-t130+t436+t523-t657+t769);
t3173 = t1037.*(t105-t465).*3.367829185e-3;
t3177 = Mt.*t4.*t5.*(-t120+t425+t519-t651+t765);
t3181 = t1037.*(t105-t465).*(-8.56645e-6);
t3205 = t1037.*(t103-t544).*(-3.367829185e-3);
t3243 = t1037.*(t103-t544).*3.367829185e-3;
t3248 = Mt.*t1495.*t1531;
t3259 = t733+t740+t942+t945;
t3266 = t1037.*(t103-t544).*(-8.56645e-6);
t3268 = t4.*t871.*(t534-t546).*(-3.36554e-3);
t3272 = t8.*t872.*(t534-t546).*(-3.36554e-3);
t3317 = t4.*t871.*(t534-t546).*3.36554e-3;
t3337 = -t3264;
t3419 = -t868.*(t271-t600-t738+t739);
t3426 = t4.*t871.*(t534-t546).*(-9.52624335e-4);
t3434 = t8.*t872.*(t534-t546).*(-9.52624335e-4);
t3435 = t4.*t871.*(t534-t546).*(-3.372816795e-3);
t3441 = t8.*t872.*(t534-t546).*(-3.372816795e-3);
t3449 = Mt.*t876.*(-t44+t390+t430-t524+t587);
t3469 = Mt.*t382.*(-t130+t436+t523-t657+t769);
t3478 = t4.*t871.*(t534-t546).*3.372816795e-3;
t3484 = Mt.*t381.*(-t120+t425+t519-t651+t765);
t3499 = t868.*(t271-t600-t738+t739);
t3519 = Mt.*t420.*(-t130+t436+t523-t657+t769);
t3527 = Mt.*t421.*(-t120+t425+t519-t651+t765);
t3531 = t22+t148+t392+t397+t428+t855+t937;
t3823 = Mt.*t1531.*t2087;
t3852 = t590+t592+t594+t707+t712+t717;
t3853 = t605+t608+t611+t684+t687+t690;
t3926 = Mt.*t1495.*(-t44+t390+t430-t524+t587);
t3931 = Mt.*t1531.*(-t51+t394+t445-t527+t614);
t3994 = -t1037.*(-t488+t603+dpsi1.*(t105-t465)+dth2.*(t103-t544));
t4121 = Mt.*t2087.*(-t44+t390+t430-t524+t587);
t4163 = t124+t125+t126+t685+t688+t691+t709+t714+t719;
t4167 = t136+t137+t138+t686+t689+t692+t706+t711+t716;
t4197 = Mt.*(-t44+t390+t430-t524+t587).*(-t51+t394+t445-t527+t614);
t4251 = t1037.*(-t488+t603+dpsi1.*(t105-t465)+dth2.*(t103-t544)).*(-3.36554e-3);
t4256 = t1037.*(-t488+t603+dpsi1.*(t105-t465)+dth2.*(t103-t544)).*3.36554e-3;
t4283 = t244+t245+t246+t781+t785+t789+t796+t798+t800;
t4284 = t283+t285+t286+t772+t774+t776+t782+t786+t790;
t4287 = t244+t245+t246+t773+t775+t777+t780+t784+t788;
t4288 = t289+t291+t292+t783+t787+t791+t795+t797+t799;
t4466 = t355+t357+t359+t958+t959+t960+t961+t962+t963;
t4593 = t298+t299+t300+t708+t713+t718+t725+t727+t729+t3209;
t4594 = t295+t296+t297+t705+t710+t715+t726+t728+t730+t3202;
t4743 = t301+t302+t303+t773+t775+t777+t780+t781+t784+t785+t788+t789+t796+t798+t800;
t644 = t8.*t561;
t646 = -t553;
t649 = -t562;
t652 = -t577;
t653 = -t580;
t654 = -t583;
t731 = t3.*t561;
t732 = -t619;
t747 = -t633;
t748 = -t638;
t823 = B_cg_H.*t3.*t11.*t576;
t824 = -t746;
t858 = -t825;
t859 = -t826;
t862 = -t832;
t863 = -t835;
t878 = t633.*(2.7e+1./1.0e+2);
t879 = t634.*(2.7e+1./1.0e+2);
t880 = t11.*t832;
t881 = t636.*(2.7e+1./1.0e+2);
t882 = t637.*(2.7e+1./1.0e+2);
t883 = t638.*(2.7e+1./1.0e+2);
t884 = t640.*(2.7e+1./1.0e+2);
t910 = -t860;
t913 = -t861;
t929 = dpsi1.*t903;
t930 = dth2.*t903;
t954 = -t949;
t956 = T_cg_H.*t925;
t964 = t184+t636;
t965 = t4.*t940;
t970 = t9.*t940;
t977 = t198+t640;
t1015 = Mb.*t10.*t926;
t1039 = t324+t634;
t1041 = -t969;
t1042 = -t971;
t1046 = -t981;
t1049 = t918./2.0;
t1058 = -t1019;
t1070 = Mb.*t2.*t5.*t926;
t1073 = Mb.*t5.*t7.*t926;
t1095 = -T_cg_H.*(t195-t634);
t1114 = -t1040;
t1115 = -t1045;
t1117 = -t1083;
t1118 = -t1084;
t1119 = -t1086;
t1125 = B_cg_H.*Mb.*t5.*t9.*t925;
t1133 = -t1072;
t1135 = -t1076;
t1144 = t1061./2.0;
t1148 = -t1098;
t1150 = -t1106;
t1155 = -t1141;
t1156 = -t1142;
t1157 = -t1143;
t1162 = -t1146;
t1163 = -t1147;
t1178 = t460+t637;
t1180 = t463+t634;
t1184 = -t1139;
t1195 = t1139./2.0;
t1208 = B_cg_H.*t1181;
t1210 = -B_cg_H.*Mb.*t4.*t5.*(t195-t634);
t1217 = T_cg_H.*t1179;
t1219 = T_cg_H.*t1181;
t1221 = t529+t737;
t1225 = dphi1.*t1179;
t1227 = dphi1.*t1181;
t1229 = dphi2.*t1179;
t1231 = dpsi1.*t1179;
t1239 = t542+t639;
t1241 = t546+t635;
t1243 = -t1193;
t1244 = -t1194;
t1267 = -dphi1.*(t530+t736);
t1280 = -t1209;
t1282 = B_cg_H.*Mb.*t4.*t5.*(t195-t634);
t1292 = -dphi1.*(t539+t641);
t1303 = -t1235;
t1306 = -t1255;
t1325 = -t1260;
t1335 = dphi1.*(t530+t736);
t1340 = dphi1.*(t539+t641);
t1349 = Mm.*t4.*t5.*t1169;
t1351 = Mm.*t5.*t9.*t1170;
t1352 = t1260./2.0;
t1357 = -t1333;
t1358 = -t1334;
t1360 = B_cg_H.*Mb.*t382.*t925;
t1361 = B_cg_H.*Mb.*t4.*t5.*t1179;
t1362 = t51+t527+t695;
t1367 = t11.*t459.*t903;
t1381 = t613+t827;
t1382 = t44+t524+t671;
t1386 = -t1356;
t1388 = t141+t497+t571;
t1389 = t142+t499+t570;
t1390 = t152+t494+t565;
t1394 = t116+t1169;
t1395 = t1365.*2.0;
t1396 = t1368.*2.0;
t1403 = -Mm.*t4.*t10.*(t530+t736);
t1404 = -Mm.*t5.*t9.*(t530+t736);
t1407 = t1323./2.0;
t1408 = t1324./2.0;
t1419 = B_cg_H.*Mb.*t420.*t925;
t1424 = t4.*t480.*t903;
t1425 = t4.*t485.*t903;
t1426 = t3.*t487.*t903;
t1430 = t545+t925;
t1432 = t3.*t506.*t903;
t1437 = -t1365;
t1439 = -t1368;
t1445 = t11.*t641.*(t105-t465);
t1451 = -t1376;
t1461 = -t1411;
t1463 = -Mm.*t5.*t30.*(t530+t736);
t1464 = t1365./2.0;
t1465 = t1366./2.0;
t1467 = t1368./2.0;
t1469 = -Mm.*t5.*t34.*(t530+t736);
t1470 = t263+t1170;
t1472 = t1372./2.0;
t1474 = t1376./2.0;
t1475 = t1377./2.0;
t1476 = Mm.*t4.*t10.*(t530+t736);
t1477 = Mm.*t5.*t9.*(t530+t736);
t1482 = -B_cg_H.*Mb.*t381.*(t195-t634);
t1488 = t673.*t903;
t1493 = -t1420;
t1511 = -t1431;
t1512 = t225+t539+t641;
t1513 = Mb.*t15.*t1368;
t1515 = -t1436;
t1520 = -t1448;
t1522 = -t1449;
t1524 = -t1452;
t1537 = t1427./2.0;
t1540 = t1431./2.0;
t1543 = Mm.*t5.*t30.*(t530+t736);
t1545 = t1436./2.0;
t1547 = t1441./2.0;
t1553 = t1448./2.0;
t1554 = t1449./2.0;
t1555 = t1450./2.0;
t1556 = t1452./2.0;
t1557 = t1454./2.0;
t1560 = -t1481;
t1561 = -B_cg_H.*Mb.*t421.*(t195-t634);
t1566 = -t1492;
t1577 = -t1499;
t1589 = Mb.*t10.*t1456;
t1609 = t1506./2.0;
t1627 = Mb.*t2.*t5.*t1456;
t1628 = -t1576;
t1629 = Mb.*t5.*t7.*t1456;
t1636 = Mm.*t381.*t1169;
t1637 = Mm.*t382.*t1170;
t1641 = -t1598;
t1644 = t1567./2.0;
t1646 = t11.*t381.*t1179;
t1649 = t1591./2.0;
t1652 = t1598./2.0;
t1657 = B_cg_H.*Mb.*t381.*t1179;
t1660 = t120+t651+t856;
t1665 = Mb.*t11.*t15.*t641.*(t197-t537);
t1668 = t2.*t1635;
t1672 = t7.*t1635;
t1676 = t130+t657+t857;
t1678 = Mm.*t421.*t1169;
t1679 = Mm.*t420.*t1170;
t1682 = -Mm.*t381.*(t530+t736);
t1683 = -Mm.*t382.*(t530+t736);
t1687 = t1653.*2.0;
t1688 = t1654.*2.0;
t1689 = t1615./2.0;
t1694 = t487.*t1179;
t1701 = t4.*t868.*t903;
t1702 = t3.*t869.*t903;
t1706 = t4.*t870.*t903;
t1707 = t4.*t871.*t903;
t1708 = t3.*t872.*t903;
t1710 = t8.*t872.*t903;
t1711 = Mt.*t10.*t1618;
t1715 = Mt.*t10.*t1619;
t1716 = Mt.*t10.*t1620;
t1726 = B_cg_H.*Mb.*t421.*t1179;
t1731 = -t1677;
t1732 = t1647./2.0;
t1737 = -Mm.*t420.*(t530+t736);
t1738 = -Mm.*t421.*(t530+t736);
t1741 = Mm.*t382.*(t530+t736);
t1742 = t1651./2.0;
t1743 = -t1685;
t1744 = t1653./2.0;
t1745 = t1654./2.0;
t1751 = -t903.*(t197-t537);
t1757 = -t903.*(t214-t541);
t1758 = Mt.*t2.*t5.*t1618;
t1759 = Mt.*t2.*t5.*t1619;
t1760 = Mt.*t2.*t5.*t1620;
t1764 = Mt.*t5.*t7.*t1618;
t1769 = Mt.*t5.*t7.*t1619;
t1770 = Mt.*t5.*t7.*t1620;
t1777 = -t1718;
t1801 = Mm.*t420.*(t530+t736);
t1802 = Mm.*t421.*(t530+t736);
C = ft_4({B_cg_H,ITail,Mb,Mm,Mt,T_cg_H,dphi1,dphi2,dpsi1,dth1,dth2,dx,dy,dz,t10,t100,t1000,t1001,t1002,t1003,t1004,t1005,t1006,t1007,t1008,t1009,t1010,t1011,t1012,t1013,t1014,t1015,t1016,t1017,t1018,t1019,t1020,t1022,t1026,t1028,t103,t1031,t1036,t1037,t1039,t1041,t1042,t1043,t1044,t1045,t1046,t1047,t1049,t105,t1050,t1051,t1052,t1053,t1054,t1055,t1056,t1057,t1058,t1059,t1060,t1061,t1062,t1063,t1064,t1065,t1067,t1070,t1071,t1072,t1073,t1074,t1075,t1076,t1077,t1078,t1079,t1080,t1081,t1082,t1084,t1085,t1086,t1087,t1088,t1089,t1090,t1091,t1092,t1093,t1094,t1095,t1096,t1097,t11,t1100,t1101,t1102,t1103,t1104,t1105,t1108,t1109,t1110,t1111,t1112,t1113,t1114,t1115,t1116,t1117,t1118,t1119,t1120,t1121,t1122,t1123,t1124,t1125,t1126,t1127,t1128,t1129,t1130,t1131,t1133,t1134,t1135,t1136,t1137,t1138,t1139,t1140,t1141,t1142,t1143,t1144,t1145,t1146,t1147,t1148,t1149,t115,t1150,t1152,t1153,t1154,t1155,t1156,t1157,t1158,t1159,t1160,t1161,t1162,t1163,t1164,t1165,t1166,t1169,t1170,t1172,t1173,t1174,t1176,t1177,t1178,t1179,t1180,t1181,t1182,t1183,t1184,t1185,t1186,t1187,t1188,t1189,t119,t1190,t1191,t1192,t1193,t1194,t1195,t1196,t1199,t120,t1200,t1201,t1203,t1205,t1206,t1208,t1209,t1211,t1212,t1213,t1214,t1215,t1217,t1219,t1221,t1223,t1225,t1227,t1229,t123,t1231,t1232,t1234,t1235,t1236,t1237,t1242,t1243,t1244,t1245,t1246,t1247,t1250,t1251,t1252,t1253,t1255,t1256,t1257,t1260,t1261,t1262,t1263,t1264,t1265,t1268,t1270,t1272,t1275,t1277,t1280,t1282,t1283,t1284,t1285,t1287,t1296,t130,t1301,t1302,t1303,t1304,t1305,t1306,t1307,t1308,t1309,t1311,t1312,t1313,t1319,t1320,t1322,t1323,t1324,t1325,t1328,t1329,t1331,t1332,t1334,t1335,t1337,t1338,t134,t1340,t1341,t1342,t1343,t1344,t1345,t1348,t1349,t1351,t1352,t1354,t1355,t1356,t1357,t1358,t1360,t1361,t1362,t1365,t1366,t1367,t1368,t1370,t1371,t1372,t1373,t1374,t1376,t1377,t1378,t1379,t1380,t1381,t1382,t1384,t1385,t1386,t1388,t1389,t1390,t1391,t1393,t1394,t1395,t1396,t1397,t1399,t1402,t1403,t1407,t1408,t1409,t1410,t1412,t1415,t1416,t1418,t1419,t1422,t1424,t1425,t1426,t1427,t1429,t1430,t1431,t1432,t1433,t1434,t1436,t1437,t1439,t144,t1441,t1442,t1443,t1444,t1445,t1446,t1448,t1449,t1450,t1451,t1452,t1453,t1454,t1455,t1456,t1457,t1458,t1459,t1460,t1461,t1463,t1464,t1465,t1467,t1469,t1470,t1472,t1474,t1475,t1476,t1477,t1478,t1479,t1481,t1482,t1486,t1488,t1489,t1491,t1492,t1493,t1495,t15,t1500,t1506,t1507,t1509,t1511,t1512,t1513,t1514,t1515,t1517,t1518,t1520,t1521,t1522,t1524,t1526,t1529,t1531,t1532,t1537,t1539,t1540,t1542,t1543,t1545,t1547,t1548,t1549,t1550,t1552,t1553,t1554,t1555,t1556,t1557,t1559,t1560,t1561,t1562,t1563,t1565,t1566,t1567,t1568,t1576,t1577,t1582,t1588,t1589,t1591,t1593,t1596,t1597,t1598,t160,t1600,t1605,t1609,t161,t1610,t1613,t1614,t1615,t1616,t1617,t1618,t1619,t162,t1620,t1627,t1628,t1629,t1632,t1635,t1636,t1637,t1639,t1640,t1641,t1642,t1644,t1645,t1646,t1647,t1648,t1649,t165,t1651,t1652,t1653,t1654,t1657,t166,t1660,t1661,t1663,t1664,t1665,t1667,t1668,t167,t1670,t1671,t1672,t1673,t1674,t1675,t1676,t1677,t1678,t1679,t1682,t1683,t1684,t1685,t1687,t1688,t1689,t169,t1690,t1691,t1692,t1693,t1694,t1700,t1701,t1702,t1704,t1706,t1707,t1708,t1709,t171,t1710,t1711,t1712,t1714,t1715,t1716,t1717,t1718,t1723,t1726,t1727,t173,t1731,t1732,t1733,t1734,t1737,t1741,t1742,t1743,t1744,t1745,t1747,t1749,t1751,t1758,t1759,t1760,t1761,t1762,t1764,t1765,t1769,t1770,t1773,t1775,t1777,t1784,t1786,t1788,t1791,t1796,t1798,t1799,t1801,t1802,t1803,t1805,t1806,t1808,t1810,t1812,t1814,t1815,t1825,t1829,t1832,t1836,t1837,t1838,t1839,t1841,t1844,t1856,t1862,t1865,t1866,t1867,t1868,t1871,t1874,t1876,t1879,t1881,t1884,t1888,t1889,t1894,t1895,t1899,t1905,t1906,t1907,t1908,t1909,t1910,t1914,t1915,t1922,t1928,t1941,t195,t1962,t1963,t1964,t1965,t1969,t197,t1970,t1971,t1972,t1973,t1974,t1975,t1979,t1981,t1982,t1983,t1989,t2,t2008,t2042,t2043,t2044,t2045,t2046,t2047,t2050,t2051,t2052,t2053,t2054,t2055,t2056,t2057,t2058,t2059,t2062,t2064,t2066,t2067,t2068,t2071,t2072,t2078,t2087,t2102,t2104,t2120,t2121,t213,t2130,t2131,t2134,t2135,t214,t2141,t2144,t2145,t2146,t2147,t2150,t2151,t2152,t2154,t2155,t2156,t2158,t2159,t2161,t2172,t2176,t2201,t2202,t2203,t2205,t2207,t2208,t2211,t2214,t2218,t2226,t2227,t2237,t2238,t2242,t2245,t2246,t2251,t2252,t2253,t2256,t2257,t2261,t2273,t23,t2302,t2303,t2305,t2307,t2311,t2312,t2320,t2321,t2322,t2323,t2324,t2326,t2328,t2331,t2337,t2339,t2350,t2351,t2360,t2363,t2385,t2386,t2388,t2389,t2392,t2393,t2398,t2399,t24,t241,t2411,t2412,t242,t2420,t243,t2461,t2462,t2463,t2464,t2466,t2467,t2468,t2469,t2477,t2479,t2480,t2481,t2485,t2489,t2490,t2492,t25,t2503,t2505,t251,t2510,t2512,t2514,t2515,t2517,t2518,t252,t253,t2530,t2531,t2546,t256,t2562,t2570,t2577,t2581,t2584,t2589,t259,t2597,t26,t260,t261,t2615,t2616,t2617,t262,t2620,t2621,t2624,t2625,t2632,t266,t2660,t2668,t2670,t2681,t2686,t2692,t2698,t2699,t27,t2704,t2706,t2707,t2710,t2715,t2716,t2717,t2718,t273,t274,t2740,t2742,t2745,t2751,t2752,t2753,t276,t2765,t277,t2783,t2784,t2788,t28,t2802,t2804,t2807,t2819,t2821,t2828,t283,t2835,t2839,t284,t2842,t2844,t285,t2857,t2859,t286,t287,t2870,t2872,t2874,t2875,t2879,t288,t2883,t2884,t289,t2890,t2891,t2896,t290,t2909,t291,t2912,t2913,t2918,t292,t293,t2938,t294,t2946,t2951,t2977,t2982,t2992,t2993,t2995,t3,t30,t3004,t3010,t3011,t3017,t3019,t3020,t3022,t3023,t3025,t3028,t3030,t3035,t304,t3047,t3048,t3051,t3059,t3060,t3065,t3078,t3081,t3090,t3109,t3117,t3124,t3130,t3134,t3135,t3136,t3144,t3170,t3173,t3177,t3181,t3243,t3248,t3259,t3260,t3266,t3272,t33,t3317,t3337,t34,t3419,t3426,t3434,t3441,t3449,t346,t3469,t347,t3478,t348,t3484,t3499,t35,t3519,t352,t3527,t3531,t354,t356,t358,t360,t370,t375,t376,t377,t38,t380,t381,t382,t3823,t383,t3852,t3853,t390,t3926,t3931,t3932,t394,t3944,t3955,t396,t3965,t3982,t399,t3994,t3998,t4,t40,t400,t4003,t4008,t401,t4014,t4033,t4038,t41,t410,t411,t412,t4121,t413,t414,t415,t4163,t4167,t418,t419,t4197,t420,t421,t424,t425,t4256,t426,t4283,t4284,t4287,t4288,t430,t431,t433,t434,t436,t437,t438,t44,t445,t4466,t447,t448,t45,t450,t451,t453,t454,t456,t459,t4593,t4594,t4597,t46,t4603,t462,t463,t464,t465,t466,t467,t470,t471,t472,t473,t474,t4743,t477,t478,t479,t48,t480,t482,t483,t484,t485,t486,t487,t488,t489,t49,t490,t491,t495,t496,t5,t50,t501,t502,t504,t505,t506,t507,t508,t509,t51,t510,t511,t512,t514,t516,t518,t519,t52,t521,t522,t523,t524,t527,t530,t532,t533,t534,t536,t537,t539,t54,t540,t541,t542,t544,t545,t546,t547,t549,t55,t550,t552,t553,t555,t557,t558,t559,t56,t560,t561,t563,t568,t569,t57,t572,t573,t574,t575,t576,t577,t578,t579,t580,t581,t582,t583,t584,t587,t59,t595,t6,t600,t602,t603,t604,t607,t61,t610,t614,t616,t617,t618,t620,t623,t624,t627,t628,t629,t630,t631,t632,t634,t641,t642,t643,t644,t645,t646,t647,t648,t649,t65,t650,t651,t652,t653,t654,t655,t657,t662,t663,t664,t665,t666,t667,t668,t669,t672,t674,t675,t676,t68,t69,t693,t694,t699,t7,t701,t703,t704,t71,t720,t721,t722,t723,t724,t73,t731,t732,t735,t736,t738,t741,t742,t743,t744,t746,t747,t748,t749,t750,t751,t752,t753,t754,t755,t756,t757,t759,t760,t761,t762,t764,t765,t768,t769,t771,t772,t774,t776,t778,t779,t792,t794,t795,t797,t799,t8,t801,t802,t803,t804,t805,t806,t807,t808,t809,t810,t811,t812,t813,t814,t815,t816,t817,t818,t819,t820,t821,t822,t823,t824,t826,t828,t829,t830,t831,t833,t834,t835,t836,t837,t838,t839,t841,t842,t843,t844,t845,t846,t847,t848,t850,t851,t852,t853,t854,t855,t858,t859,t862,t863,t864,t865,t867,t868,t869,t870,t871,t872,t873,t874,t875,t876,t878,t879,t880,t881,t882,t883,t884,t885,t886,t887,t888,t889,t890,t891,t892,t893,t894,t895,t896,t897,t898,t9,t900,t901,t902,t903,t904,t906,t907,t910,t913,t914,t915,t916,t917,t918,t919,t920,t921,t922,t923,t924,t925,t926,t927,t928,t929,t930,t932,t933,t934,t935,t936,t939,t940,t941,t947,t948,t949,t950,t951,t952,t953,t954,t955,t956,t957,t964,t965,t966,t968,t970,t972,t973,t975,t977,t978,t979,t980,t983,t985,t986,t987,t990,t991,t992,t993,t994,t995,t996,t997,t998,t999});
end
function C = ft_4(ct)
B_cg_H = ct{1};
ITail = ct{2};
Mb = ct{3};
Mm = ct{4};
Mt = ct{5};
T_cg_H = ct{6};
dphi1 = ct{7};
dphi2 = ct{8};
dpsi1 = ct{9};
dth1 = ct{10};
dth2 = ct{11};
dx = ct{12};
dy = ct{13};
dz = ct{14};
t10 = ct{15};
t100 = ct{16};
t1000 = ct{17};
t1001 = ct{18};
t1002 = ct{19};
t1003 = ct{20};
t1004 = ct{21};
t1005 = ct{22};
t1006 = ct{23};
t1007 = ct{24};
t1008 = ct{25};
t1009 = ct{26};
t1010 = ct{27};
t1011 = ct{28};
t1012 = ct{29};
t1013 = ct{30};
t1014 = ct{31};
t1015 = ct{32};
t1016 = ct{33};
t1017 = ct{34};
t1018 = ct{35};
t1019 = ct{36};
t1020 = ct{37};
t1022 = ct{38};
t1026 = ct{39};
t1028 = ct{40};
t103 = ct{41};
t1031 = ct{42};
t1036 = ct{43};
t1037 = ct{44};
t1039 = ct{45};
t1041 = ct{46};
t1042 = ct{47};
t1043 = ct{48};
t1044 = ct{49};
t1045 = ct{50};
t1046 = ct{51};
t1047 = ct{52};
t1049 = ct{53};
t105 = ct{54};
t1050 = ct{55};
t1051 = ct{56};
t1052 = ct{57};
t1053 = ct{58};
t1054 = ct{59};
t1055 = ct{60};
t1056 = ct{61};
t1057 = ct{62};
t1058 = ct{63};
t1059 = ct{64};
t1060 = ct{65};
t1061 = ct{66};
t1062 = ct{67};
t1063 = ct{68};
t1064 = ct{69};
t1065 = ct{70};
t1067 = ct{71};
t1070 = ct{72};
t1071 = ct{73};
t1072 = ct{74};
t1073 = ct{75};
t1074 = ct{76};
t1075 = ct{77};
t1076 = ct{78};
t1077 = ct{79};
t1078 = ct{80};
t1079 = ct{81};
t1080 = ct{82};
t1081 = ct{83};
t1082 = ct{84};
t1084 = ct{85};
t1085 = ct{86};
t1086 = ct{87};
t1087 = ct{88};
t1088 = ct{89};
t1089 = ct{90};
t1090 = ct{91};
t1091 = ct{92};
t1092 = ct{93};
t1093 = ct{94};
t1094 = ct{95};
t1095 = ct{96};
t1096 = ct{97};
t1097 = ct{98};
t11 = ct{99};
t1100 = ct{100};
t1101 = ct{101};
t1102 = ct{102};
t1103 = ct{103};
t1104 = ct{104};
t1105 = ct{105};
t1108 = ct{106};
t1109 = ct{107};
t1110 = ct{108};
t1111 = ct{109};
t1112 = ct{110};
t1113 = ct{111};
t1114 = ct{112};
t1115 = ct{113};
t1116 = ct{114};
t1117 = ct{115};
t1118 = ct{116};
t1119 = ct{117};
t1120 = ct{118};
t1121 = ct{119};
t1122 = ct{120};
t1123 = ct{121};
t1124 = ct{122};
t1125 = ct{123};
t1126 = ct{124};
t1127 = ct{125};
t1128 = ct{126};
t1129 = ct{127};
t1130 = ct{128};
t1131 = ct{129};
t1133 = ct{130};
t1134 = ct{131};
t1135 = ct{132};
t1136 = ct{133};
t1137 = ct{134};
t1138 = ct{135};
t1139 = ct{136};
t1140 = ct{137};
t1141 = ct{138};
t1142 = ct{139};
t1143 = ct{140};
t1144 = ct{141};
t1145 = ct{142};
t1146 = ct{143};
t1147 = ct{144};
t1148 = ct{145};
t1149 = ct{146};
t115 = ct{147};
t1150 = ct{148};
t1152 = ct{149};
t1153 = ct{150};
t1154 = ct{151};
t1155 = ct{152};
t1156 = ct{153};
t1157 = ct{154};
t1158 = ct{155};
t1159 = ct{156};
t1160 = ct{157};
t1161 = ct{158};
t1162 = ct{159};
t1163 = ct{160};
t1164 = ct{161};
t1165 = ct{162};
t1166 = ct{163};
t1169 = ct{164};
t1170 = ct{165};
t1172 = ct{166};
t1173 = ct{167};
t1174 = ct{168};
t1176 = ct{169};
t1177 = ct{170};
t1178 = ct{171};
t1179 = ct{172};
t1180 = ct{173};
t1181 = ct{174};
t1182 = ct{175};
t1183 = ct{176};
t1184 = ct{177};
t1185 = ct{178};
t1186 = ct{179};
t1187 = ct{180};
t1188 = ct{181};
t1189 = ct{182};
t119 = ct{183};
t1190 = ct{184};
t1191 = ct{185};
t1192 = ct{186};
t1193 = ct{187};
t1194 = ct{188};
t1195 = ct{189};
t1196 = ct{190};
t1199 = ct{191};
t120 = ct{192};
t1200 = ct{193};
t1201 = ct{194};
t1203 = ct{195};
t1205 = ct{196};
t1206 = ct{197};
t1208 = ct{198};
t1209 = ct{199};
t1211 = ct{200};
t1212 = ct{201};
t1213 = ct{202};
t1214 = ct{203};
t1215 = ct{204};
t1217 = ct{205};
t1219 = ct{206};
t1221 = ct{207};
t1223 = ct{208};
t1225 = ct{209};
t1227 = ct{210};
t1229 = ct{211};
t123 = ct{212};
t1231 = ct{213};
t1232 = ct{214};
t1234 = ct{215};
t1235 = ct{216};
t1236 = ct{217};
t1237 = ct{218};
t1242 = ct{219};
t1243 = ct{220};
t1244 = ct{221};
t1245 = ct{222};
t1246 = ct{223};
t1247 = ct{224};
t1250 = ct{225};
t1251 = ct{226};
t1252 = ct{227};
t1253 = ct{228};
t1255 = ct{229};
t1256 = ct{230};
t1257 = ct{231};
t1260 = ct{232};
t1261 = ct{233};
t1262 = ct{234};
t1263 = ct{235};
t1264 = ct{236};
t1265 = ct{237};
t1268 = ct{238};
t1270 = ct{239};
t1272 = ct{240};
t1275 = ct{241};
t1277 = ct{242};
t1280 = ct{243};
t1282 = ct{244};
t1283 = ct{245};
t1284 = ct{246};
t1285 = ct{247};
t1287 = ct{248};
t1296 = ct{249};
t130 = ct{250};
t1301 = ct{251};
t1302 = ct{252};
t1303 = ct{253};
t1304 = ct{254};
t1305 = ct{255};
t1306 = ct{256};
t1307 = ct{257};
t1308 = ct{258};
t1309 = ct{259};
t1311 = ct{260};
t1312 = ct{261};
t1313 = ct{262};
t1319 = ct{263};
t1320 = ct{264};
t1322 = ct{265};
t1323 = ct{266};
t1324 = ct{267};
t1325 = ct{268};
t1328 = ct{269};
t1329 = ct{270};
t1331 = ct{271};
t1332 = ct{272};
t1334 = ct{273};
t1335 = ct{274};
t1337 = ct{275};
t1338 = ct{276};
t134 = ct{277};
t1340 = ct{278};
t1341 = ct{279};
t1342 = ct{280};
t1343 = ct{281};
t1344 = ct{282};
t1345 = ct{283};
t1348 = ct{284};
t1349 = ct{285};
t1351 = ct{286};
t1352 = ct{287};
t1354 = ct{288};
t1355 = ct{289};
t1356 = ct{290};
t1357 = ct{291};
t1358 = ct{292};
t1360 = ct{293};
t1361 = ct{294};
t1362 = ct{295};
t1365 = ct{296};
t1366 = ct{297};
t1367 = ct{298};
t1368 = ct{299};
t1370 = ct{300};
t1371 = ct{301};
t1372 = ct{302};
t1373 = ct{303};
t1374 = ct{304};
t1376 = ct{305};
t1377 = ct{306};
t1378 = ct{307};
t1379 = ct{308};
t1380 = ct{309};
t1381 = ct{310};
t1382 = ct{311};
t1384 = ct{312};
t1385 = ct{313};
t1386 = ct{314};
t1388 = ct{315};
t1389 = ct{316};
t1390 = ct{317};
t1391 = ct{318};
t1393 = ct{319};
t1394 = ct{320};
t1395 = ct{321};
t1396 = ct{322};
t1397 = ct{323};
t1399 = ct{324};
t1402 = ct{325};
t1403 = ct{326};
t1407 = ct{327};
t1408 = ct{328};
t1409 = ct{329};
t1410 = ct{330};
t1412 = ct{331};
t1415 = ct{332};
t1416 = ct{333};
t1418 = ct{334};
t1419 = ct{335};
t1422 = ct{336};
t1424 = ct{337};
t1425 = ct{338};
t1426 = ct{339};
t1427 = ct{340};
t1429 = ct{341};
t1430 = ct{342};
t1431 = ct{343};
t1432 = ct{344};
t1433 = ct{345};
t1434 = ct{346};
t1436 = ct{347};
t1437 = ct{348};
t1439 = ct{349};
t144 = ct{350};
t1441 = ct{351};
t1442 = ct{352};
t1443 = ct{353};
t1444 = ct{354};
t1445 = ct{355};
t1446 = ct{356};
t1448 = ct{357};
t1449 = ct{358};
t1450 = ct{359};
t1451 = ct{360};
t1452 = ct{361};
t1453 = ct{362};
t1454 = ct{363};
t1455 = ct{364};
t1456 = ct{365};
t1457 = ct{366};
t1458 = ct{367};
t1459 = ct{368};
t1460 = ct{369};
t1461 = ct{370};
t1463 = ct{371};
t1464 = ct{372};
t1465 = ct{373};
t1467 = ct{374};
t1469 = ct{375};
t1470 = ct{376};
t1472 = ct{377};
t1474 = ct{378};
t1475 = ct{379};
t1476 = ct{380};
t1477 = ct{381};
t1478 = ct{382};
t1479 = ct{383};
t1481 = ct{384};
t1482 = ct{385};
t1486 = ct{386};
t1488 = ct{387};
t1489 = ct{388};
t1491 = ct{389};
t1492 = ct{390};
t1493 = ct{391};
t1495 = ct{392};
t15 = ct{393};
t1500 = ct{394};
t1506 = ct{395};
t1507 = ct{396};
t1509 = ct{397};
t1511 = ct{398};
t1512 = ct{399};
t1513 = ct{400};
t1514 = ct{401};
t1515 = ct{402};
t1517 = ct{403};
t1518 = ct{404};
t1520 = ct{405};
t1521 = ct{406};
t1522 = ct{407};
t1524 = ct{408};
t1526 = ct{409};
t1529 = ct{410};
t1531 = ct{411};
t1532 = ct{412};
t1537 = ct{413};
t1539 = ct{414};
t1540 = ct{415};
t1542 = ct{416};
t1543 = ct{417};
t1545 = ct{418};
t1547 = ct{419};
t1548 = ct{420};
t1549 = ct{421};
t1550 = ct{422};
t1552 = ct{423};
t1553 = ct{424};
t1554 = ct{425};
t1555 = ct{426};
t1556 = ct{427};
t1557 = ct{428};
t1559 = ct{429};
t1560 = ct{430};
t1561 = ct{431};
t1562 = ct{432};
t1563 = ct{433};
t1565 = ct{434};
t1566 = ct{435};
t1567 = ct{436};
t1568 = ct{437};
t1576 = ct{438};
t1577 = ct{439};
t1582 = ct{440};
t1588 = ct{441};
t1589 = ct{442};
t1591 = ct{443};
t1593 = ct{444};
t1596 = ct{445};
t1597 = ct{446};
t1598 = ct{447};
t160 = ct{448};
t1600 = ct{449};
t1605 = ct{450};
t1609 = ct{451};
t161 = ct{452};
t1610 = ct{453};
t1613 = ct{454};
t1614 = ct{455};
t1615 = ct{456};
t1616 = ct{457};
t1617 = ct{458};
t1618 = ct{459};
t1619 = ct{460};
t162 = ct{461};
t1620 = ct{462};
t1627 = ct{463};
t1628 = ct{464};
t1629 = ct{465};
t1632 = ct{466};
t1635 = ct{467};
t1636 = ct{468};
t1637 = ct{469};
t1639 = ct{470};
t1640 = ct{471};
t1641 = ct{472};
t1642 = ct{473};
t1644 = ct{474};
t1645 = ct{475};
t1646 = ct{476};
t1647 = ct{477};
t1648 = ct{478};
t1649 = ct{479};
t165 = ct{480};
t1651 = ct{481};
t1652 = ct{482};
t1653 = ct{483};
t1654 = ct{484};
t1657 = ct{485};
t166 = ct{486};
t1660 = ct{487};
t1661 = ct{488};
t1663 = ct{489};
t1664 = ct{490};
t1665 = ct{491};
t1667 = ct{492};
t1668 = ct{493};
t167 = ct{494};
t1670 = ct{495};
t1671 = ct{496};
t1672 = ct{497};
t1673 = ct{498};
t1674 = ct{499};
t1675 = ct{500};
t1676 = ct{501};
t1677 = ct{502};
t1678 = ct{503};
t1679 = ct{504};
t1682 = ct{505};
t1683 = ct{506};
t1684 = ct{507};
t1685 = ct{508};
t1687 = ct{509};
t1688 = ct{510};
t1689 = ct{511};
t169 = ct{512};
t1690 = ct{513};
t1691 = ct{514};
t1692 = ct{515};
t1693 = ct{516};
t1694 = ct{517};
t1700 = ct{518};
t1701 = ct{519};
t1702 = ct{520};
t1704 = ct{521};
t1706 = ct{522};
t1707 = ct{523};
t1708 = ct{524};
t1709 = ct{525};
t171 = ct{526};
t1710 = ct{527};
t1711 = ct{528};
t1712 = ct{529};
t1714 = ct{530};
t1715 = ct{531};
t1716 = ct{532};
t1717 = ct{533};
t1718 = ct{534};
t1723 = ct{535};
t1726 = ct{536};
t1727 = ct{537};
t173 = ct{538};
t1731 = ct{539};
t1732 = ct{540};
t1733 = ct{541};
t1734 = ct{542};
t1737 = ct{543};
t1741 = ct{544};
t1742 = ct{545};
t1743 = ct{546};
t1744 = ct{547};
t1745 = ct{548};
t1747 = ct{549};
t1749 = ct{550};
t1751 = ct{551};
t1758 = ct{552};
t1759 = ct{553};
t1760 = ct{554};
t1761 = ct{555};
t1762 = ct{556};
t1764 = ct{557};
t1765 = ct{558};
t1769 = ct{559};
t1770 = ct{560};
t1773 = ct{561};
t1775 = ct{562};
t1777 = ct{563};
t1784 = ct{564};
t1786 = ct{565};
t1788 = ct{566};
t1791 = ct{567};
t1796 = ct{568};
t1798 = ct{569};
t1799 = ct{570};
t1801 = ct{571};
t1802 = ct{572};
t1803 = ct{573};
t1805 = ct{574};
t1806 = ct{575};
t1808 = ct{576};
t1810 = ct{577};
t1812 = ct{578};
t1814 = ct{579};
t1815 = ct{580};
t1825 = ct{581};
t1829 = ct{582};
t1832 = ct{583};
t1836 = ct{584};
t1837 = ct{585};
t1838 = ct{586};
t1839 = ct{587};
t1841 = ct{588};
t1844 = ct{589};
t1856 = ct{590};
t1862 = ct{591};
t1865 = ct{592};
t1866 = ct{593};
t1867 = ct{594};
t1868 = ct{595};
t1871 = ct{596};
t1874 = ct{597};
t1876 = ct{598};
t1879 = ct{599};
t1881 = ct{600};
t1884 = ct{601};
t1888 = ct{602};
t1889 = ct{603};
t1894 = ct{604};
t1895 = ct{605};
t1899 = ct{606};
t1905 = ct{607};
t1906 = ct{608};
t1907 = ct{609};
t1908 = ct{610};
t1909 = ct{611};
t1910 = ct{612};
t1914 = ct{613};
t1915 = ct{614};
t1922 = ct{615};
t1928 = ct{616};
t1941 = ct{617};
t195 = ct{618};
t1962 = ct{619};
t1963 = ct{620};
t1964 = ct{621};
t1965 = ct{622};
t1969 = ct{623};
t197 = ct{624};
t1970 = ct{625};
t1971 = ct{626};
t1972 = ct{627};
t1973 = ct{628};
t1974 = ct{629};
t1975 = ct{630};
t1979 = ct{631};
t1981 = ct{632};
t1982 = ct{633};
t1983 = ct{634};
t1989 = ct{635};
t2 = ct{636};
t2008 = ct{637};
t2042 = ct{638};
t2043 = ct{639};
t2044 = ct{640};
t2045 = ct{641};
t2046 = ct{642};
t2047 = ct{643};
t2050 = ct{644};
t2051 = ct{645};
t2052 = ct{646};
t2053 = ct{647};
t2054 = ct{648};
t2055 = ct{649};
t2056 = ct{650};
t2057 = ct{651};
t2058 = ct{652};
t2059 = ct{653};
t2062 = ct{654};
t2064 = ct{655};
t2066 = ct{656};
t2067 = ct{657};
t2068 = ct{658};
t2071 = ct{659};
t2072 = ct{660};
t2078 = ct{661};
t2087 = ct{662};
t2102 = ct{663};
t2104 = ct{664};
t2120 = ct{665};
t2121 = ct{666};
t213 = ct{667};
t2130 = ct{668};
t2131 = ct{669};
t2134 = ct{670};
t2135 = ct{671};
t214 = ct{672};
t2141 = ct{673};
t2144 = ct{674};
t2145 = ct{675};
t2146 = ct{676};
t2147 = ct{677};
t2150 = ct{678};
t2151 = ct{679};
t2152 = ct{680};
t2154 = ct{681};
t2155 = ct{682};
t2156 = ct{683};
t2158 = ct{684};
t2159 = ct{685};
t2161 = ct{686};
t2172 = ct{687};
t2176 = ct{688};
t2201 = ct{689};
t2202 = ct{690};
t2203 = ct{691};
t2205 = ct{692};
t2207 = ct{693};
t2208 = ct{694};
t2211 = ct{695};
t2214 = ct{696};
t2218 = ct{697};
t2226 = ct{698};
t2227 = ct{699};
t2237 = ct{700};
t2238 = ct{701};
t2242 = ct{702};
t2245 = ct{703};
t2246 = ct{704};
t2251 = ct{705};
t2252 = ct{706};
t2253 = ct{707};
t2256 = ct{708};
t2257 = ct{709};
t2261 = ct{710};
t2273 = ct{711};
t23 = ct{712};
t2302 = ct{713};
t2303 = ct{714};
t2305 = ct{715};
t2307 = ct{716};
t2311 = ct{717};
t2312 = ct{718};
t2320 = ct{719};
t2321 = ct{720};
t2322 = ct{721};
t2323 = ct{722};
t2324 = ct{723};
t2326 = ct{724};
t2328 = ct{725};
t2331 = ct{726};
t2337 = ct{727};
t2339 = ct{728};
t2350 = ct{729};
t2351 = ct{730};
t2360 = ct{731};
t2363 = ct{732};
t2385 = ct{733};
t2386 = ct{734};
t2388 = ct{735};
t2389 = ct{736};
t2392 = ct{737};
t2393 = ct{738};
t2398 = ct{739};
t2399 = ct{740};
t24 = ct{741};
t241 = ct{742};
t2411 = ct{743};
t2412 = ct{744};
t242 = ct{745};
t2420 = ct{746};
t243 = ct{747};
t2461 = ct{748};
t2462 = ct{749};
t2463 = ct{750};
t2464 = ct{751};
t2466 = ct{752};
t2467 = ct{753};
t2468 = ct{754};
t2469 = ct{755};
t2477 = ct{756};
t2479 = ct{757};
t2480 = ct{758};
t2481 = ct{759};
t2485 = ct{760};
t2489 = ct{761};
t2490 = ct{762};
t2492 = ct{763};
t25 = ct{764};
t2503 = ct{765};
t2505 = ct{766};
t251 = ct{767};
t2510 = ct{768};
t2512 = ct{769};
t2514 = ct{770};
t2515 = ct{771};
t2517 = ct{772};
t2518 = ct{773};
t252 = ct{774};
t253 = ct{775};
t2530 = ct{776};
t2531 = ct{777};
t2546 = ct{778};
t256 = ct{779};
t2562 = ct{780};
t2570 = ct{781};
t2577 = ct{782};
t2581 = ct{783};
t2584 = ct{784};
t2589 = ct{785};
t259 = ct{786};
t2597 = ct{787};
t26 = ct{788};
t260 = ct{789};
t261 = ct{790};
t2615 = ct{791};
t2616 = ct{792};
t2617 = ct{793};
t262 = ct{794};
t2620 = ct{795};
t2621 = ct{796};
t2624 = ct{797};
t2625 = ct{798};
t2632 = ct{799};
t266 = ct{800};
t2660 = ct{801};
t2668 = ct{802};
t2670 = ct{803};
t2681 = ct{804};
t2686 = ct{805};
t2692 = ct{806};
t2698 = ct{807};
t2699 = ct{808};
t27 = ct{809};
t2704 = ct{810};
t2706 = ct{811};
t2707 = ct{812};
t2710 = ct{813};
t2715 = ct{814};
t2716 = ct{815};
t2717 = ct{816};
t2718 = ct{817};
t273 = ct{818};
t274 = ct{819};
t2740 = ct{820};
t2742 = ct{821};
t2745 = ct{822};
t2751 = ct{823};
t2752 = ct{824};
t2753 = ct{825};
t276 = ct{826};
t2765 = ct{827};
t277 = ct{828};
t2783 = ct{829};
t2784 = ct{830};
t2788 = ct{831};
t28 = ct{832};
t2802 = ct{833};
t2804 = ct{834};
t2807 = ct{835};
t2819 = ct{836};
t2821 = ct{837};
t2828 = ct{838};
t283 = ct{839};
t2835 = ct{840};
t2839 = ct{841};
t284 = ct{842};
t2842 = ct{843};
t2844 = ct{844};
t285 = ct{845};
t2857 = ct{846};
t2859 = ct{847};
t286 = ct{848};
t287 = ct{849};
t2870 = ct{850};
t2872 = ct{851};
t2874 = ct{852};
t2875 = ct{853};
t2879 = ct{854};
t288 = ct{855};
t2883 = ct{856};
t2884 = ct{857};
t289 = ct{858};
t2890 = ct{859};
t2891 = ct{860};
t2896 = ct{861};
t290 = ct{862};
t2909 = ct{863};
t291 = ct{864};
t2912 = ct{865};
t2913 = ct{866};
t2918 = ct{867};
t292 = ct{868};
t293 = ct{869};
t2938 = ct{870};
t294 = ct{871};
t2946 = ct{872};
t2951 = ct{873};
t2977 = ct{874};
t2982 = ct{875};
t2992 = ct{876};
t2993 = ct{877};
t2995 = ct{878};
t3 = ct{879};
t30 = ct{880};
t3004 = ct{881};
t3010 = ct{882};
t3011 = ct{883};
t3017 = ct{884};
t3019 = ct{885};
t3020 = ct{886};
t3022 = ct{887};
t3023 = ct{888};
t3025 = ct{889};
t3028 = ct{890};
t3030 = ct{891};
t3035 = ct{892};
t304 = ct{893};
t3047 = ct{894};
t3048 = ct{895};
t3051 = ct{896};
t3059 = ct{897};
t3060 = ct{898};
t3065 = ct{899};
t3078 = ct{900};
t3081 = ct{901};
t3090 = ct{902};
t3109 = ct{903};
t3117 = ct{904};
t3124 = ct{905};
t3130 = ct{906};
t3134 = ct{907};
t3135 = ct{908};
t3136 = ct{909};
t3144 = ct{910};
t3170 = ct{911};
t3173 = ct{912};
t3177 = ct{913};
t3181 = ct{914};
t3243 = ct{915};
t3248 = ct{916};
t3259 = ct{917};
t3260 = ct{918};
t3266 = ct{919};
t3272 = ct{920};
t33 = ct{921};
t3317 = ct{922};
t3337 = ct{923};
t34 = ct{924};
t3419 = ct{925};
t3426 = ct{926};
t3434 = ct{927};
t3441 = ct{928};
t3449 = ct{929};
t346 = ct{930};
t3469 = ct{931};
t347 = ct{932};
t3478 = ct{933};
t348 = ct{934};
t3484 = ct{935};
t3499 = ct{936};
t35 = ct{937};
t3519 = ct{938};
t352 = ct{939};
t3527 = ct{940};
t3531 = ct{941};
t354 = ct{942};
t356 = ct{943};
t358 = ct{944};
t360 = ct{945};
t370 = ct{946};
t375 = ct{947};
t376 = ct{948};
t377 = ct{949};
t38 = ct{950};
t380 = ct{951};
t381 = ct{952};
t382 = ct{953};
t3823 = ct{954};
t383 = ct{955};
t3852 = ct{956};
t3853 = ct{957};
t390 = ct{958};
t3926 = ct{959};
t3931 = ct{960};
t3932 = ct{961};
t394 = ct{962};
t3944 = ct{963};
t3955 = ct{964};
t396 = ct{965};
t3965 = ct{966};
t3982 = ct{967};
t399 = ct{968};
t3994 = ct{969};
t3998 = ct{970};
t4 = ct{971};
t40 = ct{972};
t400 = ct{973};
t4003 = ct{974};
t4008 = ct{975};
t401 = ct{976};
t4014 = ct{977};
t4033 = ct{978};
t4038 = ct{979};
t41 = ct{980};
t410 = ct{981};
t411 = ct{982};
t412 = ct{983};
t4121 = ct{984};
t413 = ct{985};
t414 = ct{986};
t415 = ct{987};
t4163 = ct{988};
t4167 = ct{989};
t418 = ct{990};
t419 = ct{991};
t4197 = ct{992};
t420 = ct{993};
t421 = ct{994};
t424 = ct{995};
t425 = ct{996};
t4256 = ct{997};
t426 = ct{998};
t4283 = ct{999};
t4284 = ct{1000};
t4287 = ct{1001};
t4288 = ct{1002};
t430 = ct{1003};
t431 = ct{1004};
t433 = ct{1005};
t434 = ct{1006};
t436 = ct{1007};
t437 = ct{1008};
t438 = ct{1009};
t44 = ct{1010};
t445 = ct{1011};
t4466 = ct{1012};
t447 = ct{1013};
t448 = ct{1014};
t45 = ct{1015};
t450 = ct{1016};
t451 = ct{1017};
t453 = ct{1018};
t454 = ct{1019};
t456 = ct{1020};
t459 = ct{1021};
t4593 = ct{1022};
t4594 = ct{1023};
t4597 = ct{1024};
t46 = ct{1025};
t4603 = ct{1026};
t462 = ct{1027};
t463 = ct{1028};
t464 = ct{1029};
t465 = ct{1030};
t466 = ct{1031};
t467 = ct{1032};
t470 = ct{1033};
t471 = ct{1034};
t472 = ct{1035};
t473 = ct{1036};
t474 = ct{1037};
t4743 = ct{1038};
t477 = ct{1039};
t478 = ct{1040};
t479 = ct{1041};
t48 = ct{1042};
t480 = ct{1043};
t482 = ct{1044};
t483 = ct{1045};
t484 = ct{1046};
t485 = ct{1047};
t486 = ct{1048};
t487 = ct{1049};
t488 = ct{1050};
t489 = ct{1051};
t49 = ct{1052};
t490 = ct{1053};
t491 = ct{1054};
t495 = ct{1055};
t496 = ct{1056};
t5 = ct{1057};
t50 = ct{1058};
t501 = ct{1059};
t502 = ct{1060};
t504 = ct{1061};
t505 = ct{1062};
t506 = ct{1063};
t507 = ct{1064};
t508 = ct{1065};
t509 = ct{1066};
t51 = ct{1067};
t510 = ct{1068};
t511 = ct{1069};
t512 = ct{1070};
t514 = ct{1071};
t516 = ct{1072};
t518 = ct{1073};
t519 = ct{1074};
t52 = ct{1075};
t521 = ct{1076};
t522 = ct{1077};
t523 = ct{1078};
t524 = ct{1079};
t527 = ct{1080};
t530 = ct{1081};
t532 = ct{1082};
t533 = ct{1083};
t534 = ct{1084};
t536 = ct{1085};
t537 = ct{1086};
t539 = ct{1087};
t54 = ct{1088};
t540 = ct{1089};
t541 = ct{1090};
t542 = ct{1091};
t544 = ct{1092};
t545 = ct{1093};
t546 = ct{1094};
t547 = ct{1095};
t549 = ct{1096};
t55 = ct{1097};
t550 = ct{1098};
t552 = ct{1099};
t553 = ct{1100};
t555 = ct{1101};
t557 = ct{1102};
t558 = ct{1103};
t559 = ct{1104};
t56 = ct{1105};
t560 = ct{1106};
t561 = ct{1107};
t563 = ct{1108};
t568 = ct{1109};
t569 = ct{1110};
t57 = ct{1111};
t572 = ct{1112};
t573 = ct{1113};
t574 = ct{1114};
t575 = ct{1115};
t576 = ct{1116};
t577 = ct{1117};
t578 = ct{1118};
t579 = ct{1119};
t580 = ct{1120};
t581 = ct{1121};
t582 = ct{1122};
t583 = ct{1123};
t584 = ct{1124};
t587 = ct{1125};
t59 = ct{1126};
t595 = ct{1127};
t6 = ct{1128};
t600 = ct{1129};
t602 = ct{1130};
t603 = ct{1131};
t604 = ct{1132};
t607 = ct{1133};
t61 = ct{1134};
t610 = ct{1135};
t614 = ct{1136};
t616 = ct{1137};
t617 = ct{1138};
t618 = ct{1139};
t620 = ct{1140};
t623 = ct{1141};
t624 = ct{1142};
t627 = ct{1143};
t628 = ct{1144};
t629 = ct{1145};
t630 = ct{1146};
t631 = ct{1147};
t632 = ct{1148};
t634 = ct{1149};
t641 = ct{1150};
t642 = ct{1151};
t643 = ct{1152};
t644 = ct{1153};
t645 = ct{1154};
t646 = ct{1155};
t647 = ct{1156};
t648 = ct{1157};
t649 = ct{1158};
t65 = ct{1159};
t650 = ct{1160};
t651 = ct{1161};
t652 = ct{1162};
t653 = ct{1163};
t654 = ct{1164};
t655 = ct{1165};
t657 = ct{1166};
t662 = ct{1167};
t663 = ct{1168};
t664 = ct{1169};
t665 = ct{1170};
t666 = ct{1171};
t667 = ct{1172};
t668 = ct{1173};
t669 = ct{1174};
t672 = ct{1175};
t674 = ct{1176};
t675 = ct{1177};
t676 = ct{1178};
t68 = ct{1179};
t69 = ct{1180};
t693 = ct{1181};
t694 = ct{1182};
t699 = ct{1183};
t7 = ct{1184};
t701 = ct{1185};
t703 = ct{1186};
t704 = ct{1187};
t71 = ct{1188};
t720 = ct{1189};
t721 = ct{1190};
t722 = ct{1191};
t723 = ct{1192};
t724 = ct{1193};
t73 = ct{1194};
t731 = ct{1195};
t732 = ct{1196};
t735 = ct{1197};
t736 = ct{1198};
t738 = ct{1199};
t741 = ct{1200};
t742 = ct{1201};
t743 = ct{1202};
t744 = ct{1203};
t746 = ct{1204};
t747 = ct{1205};
t748 = ct{1206};
t749 = ct{1207};
t750 = ct{1208};
t751 = ct{1209};
t752 = ct{1210};
t753 = ct{1211};
t754 = ct{1212};
t755 = ct{1213};
t756 = ct{1214};
t757 = ct{1215};
t759 = ct{1216};
t760 = ct{1217};
t761 = ct{1218};
t762 = ct{1219};
t764 = ct{1220};
t765 = ct{1221};
t768 = ct{1222};
t769 = ct{1223};
t771 = ct{1224};
t772 = ct{1225};
t774 = ct{1226};
t776 = ct{1227};
t778 = ct{1228};
t779 = ct{1229};
t792 = ct{1230};
t794 = ct{1231};
t795 = ct{1232};
t797 = ct{1233};
t799 = ct{1234};
t8 = ct{1235};
t801 = ct{1236};
t802 = ct{1237};
t803 = ct{1238};
t804 = ct{1239};
t805 = ct{1240};
t806 = ct{1241};
t807 = ct{1242};
t808 = ct{1243};
t809 = ct{1244};
t810 = ct{1245};
t811 = ct{1246};
t812 = ct{1247};
t813 = ct{1248};
t814 = ct{1249};
t815 = ct{1250};
t816 = ct{1251};
t817 = ct{1252};
t818 = ct{1253};
t819 = ct{1254};
t820 = ct{1255};
t821 = ct{1256};
t822 = ct{1257};
t823 = ct{1258};
t824 = ct{1259};
t826 = ct{1260};
t828 = ct{1261};
t829 = ct{1262};
t830 = ct{1263};
t831 = ct{1264};
t833 = ct{1265};
t834 = ct{1266};
t835 = ct{1267};
t836 = ct{1268};
t837 = ct{1269};
t838 = ct{1270};
t839 = ct{1271};
t841 = ct{1272};
t842 = ct{1273};
t843 = ct{1274};
t844 = ct{1275};
t845 = ct{1276};
t846 = ct{1277};
t847 = ct{1278};
t848 = ct{1279};
t850 = ct{1280};
t851 = ct{1281};
t852 = ct{1282};
t853 = ct{1283};
t854 = ct{1284};
t855 = ct{1285};
t858 = ct{1286};
t859 = ct{1287};
t862 = ct{1288};
t863 = ct{1289};
t864 = ct{1290};
t865 = ct{1291};
t867 = ct{1292};
t868 = ct{1293};
t869 = ct{1294};
t870 = ct{1295};
t871 = ct{1296};
t872 = ct{1297};
t873 = ct{1298};
t874 = ct{1299};
t875 = ct{1300};
t876 = ct{1301};
t878 = ct{1302};
t879 = ct{1303};
t880 = ct{1304};
t881 = ct{1305};
t882 = ct{1306};
t883 = ct{1307};
t884 = ct{1308};
t885 = ct{1309};
t886 = ct{1310};
t887 = ct{1311};
t888 = ct{1312};
t889 = ct{1313};
t890 = ct{1314};
t891 = ct{1315};
t892 = ct{1316};
t893 = ct{1317};
t894 = ct{1318};
t895 = ct{1319};
t896 = ct{1320};
t897 = ct{1321};
t898 = ct{1322};
t9 = ct{1323};
t900 = ct{1324};
t901 = ct{1325};
t902 = ct{1326};
t903 = ct{1327};
t904 = ct{1328};
t906 = ct{1329};
t907 = ct{1330};
t910 = ct{1331};
t913 = ct{1332};
t914 = ct{1333};
t915 = ct{1334};
t916 = ct{1335};
t917 = ct{1336};
t918 = ct{1337};
t919 = ct{1338};
t920 = ct{1339};
t921 = ct{1340};
t922 = ct{1341};
t923 = ct{1342};
t924 = ct{1343};
t925 = ct{1344};
t926 = ct{1345};
t927 = ct{1346};
t928 = ct{1347};
t929 = ct{1348};
t930 = ct{1349};
t932 = ct{1350};
t933 = ct{1351};
t934 = ct{1352};
t935 = ct{1353};
t936 = ct{1354};
t939 = ct{1355};
t940 = ct{1356};
t941 = ct{1357};
t947 = ct{1358};
t948 = ct{1359};
t949 = ct{1360};
t950 = ct{1361};
t951 = ct{1362};
t952 = ct{1363};
t953 = ct{1364};
t954 = ct{1365};
t955 = ct{1366};
t956 = ct{1367};
t957 = ct{1368};
t964 = ct{1369};
t965 = ct{1370};
t966 = ct{1371};
t968 = ct{1372};
t970 = ct{1373};
t972 = ct{1374};
t973 = ct{1375};
t975 = ct{1376};
t977 = ct{1377};
t978 = ct{1378};
t979 = ct{1379};
t980 = ct{1380};
t983 = ct{1381};
t985 = ct{1382};
t986 = ct{1383};
t987 = ct{1384};
t990 = ct{1385};
t991 = ct{1386};
t992 = ct{1387};
t993 = ct{1388};
t994 = ct{1389};
t995 = ct{1390};
t996 = ct{1391};
t997 = ct{1392};
t998 = ct{1393};
t999 = ct{1394};
t1813 = t903.*t1037;
t1817 = t903.*(t197-t537);
t1819 = t903.*t1044;
t1820 = -t1786;
t1824 = t903.*t1047;
t1826 = t903.*(t214-t541);
t1830 = -t1761;
t1851 = t1761./2.0;
t1852 = t1762./2.0;
t1854 = t1832.*(-1.0./2.0);
t1873 = t1832./2.0;
t1875 = t918.*3.36554e-3;
t1886 = t1866.*(-1.0./2.0);
t1896 = -Mm.*t651.*(t530+t736);
t1897 = Mt.*t4.*t5.*t1727;
t1903 = Mt.*t5.*t9.*t1734;
t1911 = t1866./2.0;
t1912 = -t1889;
t1913 = -t1868;
t1916 = -t1899;
t1918 = t23+t40+t852+t926;
t1919 = -t1876;
t1921 = -t1879;
t1925 = -t1179.*(t105-t465);
t1926 = -t1181.*(t105-t465);
t1930 = -t1907;
t1931 = -t1910;
t1936 = t1868./2.0;
t1940 = t1871./2.0;
t1942 = Mm.*t651.*(t530+t736);
t1954 = t1876./2.0;
t1956 = t903.*t1179;
t1958 = t1879./2.0;
t1960 = -t1928;
t1961 = t918.*3.372816795e-3;
t1966 = t1061.*3.36554e-3;
t1985 = t918.*9.52624335e-4;
t1990 = t1179.*(t105-t465);
t1998 = -t1964;
t1999 = -t1965;
t2004 = -t1970;
t2007 = -t1972;
t2015 = B_cg_H.*Mb.*t485.*t1456;
t2025 = -t1983;
t2026 = -t1179.*(t103-t544);
t2028 = -t903.*(t534-t546);
t2031 = t274+t489+t490+t647;
t2035 = t1181.*(t105-t465).*(-1.0./2.0);
t2037 = t1139.*3.36554e-3;
t2063 = dth1.*t1981;
t2069 = -t1979;
t2090 = -t2044;
t2091 = -t2047;
t2094 = -t2051;
t2095 = -t2054;
t2096 = -t2055;
t2097 = -t2057;
t2098 = -t2059;
t2118 = -t2071;
t2119 = -t2072;
t2127 = t1989./2.0;
t2148 = Mb.*t5.*t1981;
t2157 = t1061.*3.367829185e-3;
t2165 = t1179.*(t103-t544).*(-1.0./2.0);
t2167 = t903.*(t534-t546).*(-1.0./2.0);
t2171 = -t2131;
t2178 = -t2145;
t2179 = -t2147;
t2180 = t1031.*t1179;
t2181 = -t2152;
t2182 = -t2155;
t2183 = -t2156;
t2186 = -t2158;
t2188 = Mm.*t1007.*t1169;
t2190 = -t2159;
t2196 = Mm.*t1013.*t1170;
t2209 = t1061.*8.56645e-6;
t2215 = t1139.*9.52624335e-4;
t2220 = t1139.*3.372816795e-3;
t2222 = Mb.*t2.*t10.*t1981;
t2224 = Mt.*t381.*t1727;
t2225 = Mb.*t7.*t10.*t1981;
t2231 = Mt.*t382.*t1734;
t2240 = t370+t396+t462+t932;
t2247 = t2121./2.0;
t2249 = -t2202;
t2254 = -t2207;
t2255 = -t2208;
t2259 = -t2218;
t2262 = -t2226;
t2263 = -t2227;
t2264 = t260+t549+t620+t803;
t2266 = t259+t552+t628+t806;
t2278 = -Mm.*t1009.*(t530+t736);
t2280 = -Mm.*t1013.*(t530+t736);
t2283 = t1260.*3.36554e-3;
t2287 = -t2251;
t2288 = -t2253;
t2290 = -t2256;
t2291 = t467+t828+t1022;
t2294 = Mt.*t421.*t1727;
t2295 = t470+t831+t1028;
t2298 = Mt.*t420.*t1734;
t2306 = dphi2.*t2203;
t2327 = t261+t630+t704+t807;
t2335 = -t2302;
t2336 = -t2273;
t2340 = -t2305;
t2341 = Mm.*t1009.*(t530+t736);
t2342 = -t2311;
t2343 = -t2312;
t2345 = Mm.*t1013.*(t530+t736);
t2346 = t1323.*3.36554e-3;
t2347 = t1324.*3.36554e-3;
t2349 = -t2323;
t2356 = Mt.*t5.*t2203;
t2358 = t1365.*6.73108e-3;
t2359 = t1368.*6.73108e-3;
t2362 = -t2337;
t2376 = -dth2.*(t433-t828+T_cg_H.*(t197-t537));
t2379 = B_cg_H.*Mb.*t871.*t1456;
t2383 = t1260.*3.372786875e-3;
t2387 = t1260.*9.53094055e-4;
t2390 = B_cg_H.*Mb.*t7.*t100.*t1981;
t2394 = t352+t600+t738+t815;
t2395 = t354+t602+t742+t816;
t2397 = -t2331;
t2400 = t1365.*3.36554e-3;
t2401 = t1366.*3.36554e-3;
t2404 = t1368.*3.36554e-3;
t2407 = t1372.*3.36554e-3;
t2408 = t1376.*3.36554e-3;
t2409 = t1377.*3.36554e-3;
t2427 = Mt.*t2.*t10.*t2203;
t2429 = Mt.*t7.*t10.*t2203;
t2430 = -t2392;
t2431 = -t2393;
t2433 = -t2398;
t2435 = -t1179.*(t534-t546);
t2447 = -t2412;
t2474 = t1323.*3.367829185e-3;
t2475 = t1324.*3.367829185e-3;
t2476 = t1427.*3.36554e-3;
t2482 = t1431.*3.36554e-3;
t2487 = t1436.*3.36554e-3;
t2488 = t1441.*3.36554e-3;
t2493 = t1448.*3.36554e-3;
t2494 = t1449.*3.36554e-3;
t2495 = t1450.*3.36554e-3;
t2497 = t1452.*3.36554e-3;
t2504 = t1454.*3.36554e-3;
t2516 = -t2420;
t2519 = Mt.*t10.*t2360;
t2520 = -t2468;
t2527 = t45+t115+t1007+t1087;
t2532 = -Mt.*t4.*t5.*(t433-t828+T_cg_H.*(t197-t537));
t2534 = -t2481;
t2539 = t1179.*(t534-t546);
t2544 = -Mt.*t9.*t10.*(t433-t828+T_cg_H.*(t197-t537));
t2545 = -t2490;
t2553 = -Mt.*t5.*t9.*(t451-t831+T_cg_H.*(t214-t541));
t2560 = -t2510;
t2563 = t52+t119+t1013+t1096;
t2564 = -t2515;
t2565 = -t2517;
t2566 = -t2518;
t2576 = t1506.*3.36554e-3;
t2586 = t1365.*9.52624335e-4;
t2587 = t1365.*1.90524867e-3;
t2588 = t1366.*9.52624335e-4;
t2590 = t1368.*9.52624335e-4;
t2591 = t1368.*1.90524867e-3;
t2598 = t1365.*3.372816795e-3;
t2599 = t1365.*6.74563359e-3;
t2600 = t1366.*3.372816795e-3;
t2603 = t1368.*3.372816795e-3;
t2604 = t1368.*6.74563359e-3;
t2607 = t1372.*3.372786875e-3;
t2608 = t1376.*9.52624335e-4;
t2611 = t1323.*8.56645e-6;
t2612 = t1324.*8.56645e-6;
t2613 = t1377.*3.372786875e-3;
t2614 = t1372.*9.53094055e-4;
t2619 = t1376.*3.372816795e-3;
t2622 = t1377.*9.53094055e-4;
t2626 = Mt.*t5.*t7.*t2360;
t2627 = t46+t266+t1016+t1100;
t2633 = -Mt.*t5.*t33.*(t433-t828+T_cg_H.*(t197-t537));
t2634 = -Mt.*t5.*t38.*(t433-t828+T_cg_H.*(t197-t537));
t2638 = t41+t256+t1009+t1089;
t2654 = Mt.*t5.*t9.*(t451-t831+T_cg_H.*(t214-t541));
t2662 = Mt.*t2.*t5.*t2360;
t2663 = -t2625;
t2664 = t1454.*9.53094055e-4;
t2665 = t2.*t2570;
t2669 = t7.*t2570;
t2671 = t1567.*3.36554e-3;
t2673 = -t2570;
t2682 = t1591.*3.36554e-3;
t2689 = t1427.*3.372786875e-3;
t2693 = t1598.*3.36554e-3;
t2694 = t1431.*3.372786875e-3;
t2695 = t1427.*9.53094055e-4;
t2700 = t1431.*9.53094055e-4;
t2701 = t1436.*9.52624335e-4;
t2702 = -t2589;
t2705 = t1441.*3.372786875e-3;
t2708 = t1436.*3.372816795e-3;
t2711 = t1441.*9.53094055e-4;
t2712 = t1448.*9.52624335e-4;
t2713 = t1449.*9.52624335e-4;
t2714 = t1450.*9.52624335e-4;
t2719 = t1452.*3.372786875e-3;
t2720 = t1448.*3.372816795e-3;
t2721 = t1449.*3.372816795e-3;
t2722 = t1450.*3.372816795e-3;
t2723 = t1454.*3.372786875e-3;
t2724 = t1452.*9.53094055e-4;
t2730 = t437+t474+t522+t1103;
t2731 = Mt.*t5.*t33.*(t433-t828+T_cg_H.*(t197-t537));
t2732 = Mt.*t5.*t38.*(t433-t828+T_cg_H.*(t197-t537));
t2749 = t1615.*3.36554e-3;
t2756 = -t2716;
t2763 = t426+t472+t518+t1091;
t2764 = -t2668;
t2766 = -t2670;
t2774 = -t2681;
t2776 = -t2686;
t2781 = t1653.*6.73108e-3;
t2782 = t1654.*6.73108e-3;
t2786 = -t2753;
t2787 = t1506.*3.367829185e-3;
t2790 = B_cg_H.*Mb.*t495.*t1981;
t2803 = t1647.*3.36554e-3;
t2806 = t1651.*3.36554e-3;
t2812 = t1653.*3.36554e-3;
t2813 = t1654.*3.36554e-3;
t2820 = t1598.*3.367829185e-3;
t2825 = t1506.*8.56645e-6;
t2837 = t1567.*3.367829185e-3;
t2841 = t1591.*3.367829185e-3;
t2880 = t1615.*9.52624335e-4;
t2886 = t1615.*3.372816795e-3;
t2887 = B_cg_H.*Mb.*t555.*t1981;
t2888 = B_cg_H.*Mb.*t557.*t1981;
t2889 = B_cg_H.*Mb.*t558.*t1981;
t2892 = t1567.*8.56645e-6;
t2894 = -Mt.*t381.*(t433-t828+T_cg_H.*(t197-t537));
t2895 = -Mt.*t382.*(t433-t828+T_cg_H.*(t197-t537));
t2902 = t1591.*8.56645e-6;
t2907 = -Mt.*t382.*(t451-t831+T_cg_H.*(t214-t541));
t2908 = t1598.*8.56645e-6;
t2916 = -t2891;
t2928 = t1761.*3.36554e-3;
t2929 = t1762.*3.36554e-3;
t2932 = t1832.*(-3.36554e-3);
t2945 = t1647.*3.372786875e-3;
t2949 = t1651.*3.372786875e-3;
t2950 = t1647.*9.53094055e-4;
t2952 = t1651.*9.53094055e-4;
t2954 = t1653.*9.52624335e-4;
t2955 = t1653.*1.90524867e-3;
t2956 = t1654.*9.52624335e-4;
t2957 = t1654.*1.90524867e-3;
t2958 = t1653.*3.372816795e-3;
t2959 = t1653.*6.74563359e-3;
t2960 = t1654.*3.372816795e-3;
t2961 = t1654.*6.74563359e-3;
t2967 = -Mt.*t420.*(t433-t828+T_cg_H.*(t197-t537));
t2968 = -Mt.*t421.*(t433-t828+T_cg_H.*(t197-t537));
t2969 = Mt.*t381.*(t433-t828+T_cg_H.*(t197-t537));
t2975 = -Mt.*t420.*(t451-t831+T_cg_H.*(t214-t541));
t2988 = t1866.*(-3.36554e-3);
t3034 = B_cg_H.*Mb.*t819.*t1981;
t3039 = Mt.*t421.*(t433-t828+T_cg_H.*(t197-t537));
t3055 = t1879.*3.36554e-3;
t3058 = t1868.*3.36554e-3;
t3063 = t1871.*3.36554e-3;
t3067 = t486+t642+t902+t939;
t3068 = t477+t645+t901+t940;
t3074 = t1762.*3.372786875e-3;
t3075 = t1832.*(-3.372786875e-3);
t3077 = t1762.*9.53094055e-4;
t3079 = t1832.*(-9.53094055e-4);
t3085 = t1761.*3.367829185e-3;
t3088 = t1876.*3.36554e-3;
t3105 = t1832.*9.53094055e-4;
t3111 = Mb.*t926.*t1981;
t3120 = t1761.*8.56645e-6;
t3126 = t1866.*(-9.52624335e-4);
t3132 = t1866.*(-3.372816795e-3);
t3138 = t399+t530+t736+t1277;
t3153 = t1181.*(t105-t465).*(-3.36554e-3);
t3165 = t1866.*9.52624335e-4;
t3182 = t629+t802+t902+t939;
t3186 = t1876.*9.52624335e-4;
t3188 = t1879.*9.52624335e-4;
t3191 = t1876.*3.372816795e-3;
t3194 = t1879.*3.372816795e-3;
t3199 = t1868.*9.52624335e-4;
t3200 = t1871.*9.52624335e-4;
t3201 = t1868.*3.372816795e-3;
t3204 = t1871.*3.372816795e-3;
t3208 = t488+t703+t935+t975;
t3210 = t1179.*(t103-t544).*(-3.36554e-3);
t3212 = t903.*(t534-t546).*(-3.36554e-3);
t3218 = t1989.*3.36554e-3;
t3235 = t7.*t35.*t2993;
t3237 = -t3170;
t3247 = t2008.*3.36554e-3;
t3249 = -t3177;
t3256 = Mt.*t876.*t2203;
t3265 = t868.*t2261;
t3269 = t2121.*3.36554e-3;
t3285 = t1181.*(t105-t465).*(-3.372786875e-3);
t3291 = t1181.*(t105-t465).*(-9.53094055e-4);
t3304 = -t3248;
t3310 = t2104.*3.36554e-3;
t3330 = Mt.*t1531.*t1618;
t3331 = Mt.*t1531.*t1620;
t3351 = t903.*(t534-t546).*(-3.372786875e-3);
t3360 = t1989.*3.372786875e-3;
t3364 = t903.*(t534-t546).*(-9.53094055e-4);
t3370 = t1989.*9.53094055e-4;
t3380 = t1179.*(t103-t544).*(-3.367829185e-3);
t3428 = t2121.*3.372786875e-3;
t3438 = t2121.*9.53094055e-4;
t3459 = t1179.*(t103-t544).*(-8.56645e-6);
t3471 = t380.*t2993;
t3504 = -t3449;
t3520 = -t3469;
t3521 = t418.*t2993;
t3522 = t419.*t2993;
t3565 = -t3519;
t3580 = dth1.*t3531;
t3581 = -t3527;
t3644 = Mt.*t5.*t3531;
t3701 = Mt.*t2.*t10.*t3531;
t3704 = Mt.*t7.*t10.*t3531;
t3709 = Mb.*t1456.*t1981;
t3847 = -t3823;
t3858 = Mt.*t1495.*t2203;
t3862 = t868.*t3144;
t3880 = dx.*t3852;
t3881 = dx.*t3853;
t3882 = dy.*t3853;
t3883 = dz.*t3852;
t3902 = Mt.*t1618.*t2203;
t3908 = Mt.*t1619.*t2203;
t3909 = Mt.*t1620.*t2203;
t3916 = Mt.*t1531.*t2360;
t3930 = t868.*t3259;
t3937 = t52+t119+t453+t454+t540+t1013+t1101;
t3940 = t45+t115+t438+t447+t536+t1007+t1090;
t3957 = -t3926;
t3959 = -t3931;
t3962 = Mt.*t1618.*(-t44+t390+t430-t524+t587);
t3963 = Mt.*t1619.*(-t44+t390+t430-t524+t587);
t3964 = Mt.*t1620.*(-t44+t390+t430-t524+t587);
t3969 = t46+t266+t448+t473+t521+t1016+t1104;
t3971 = t41+t256+t431+t471+t516+t1009+t1092;
t3996 = -Mt.*t1734.*(t433-t828+T_cg_H.*(t197-t537));
t4042 = t3499.*(-3.36554e-3);
t4054 = Mt.*t876.*t3531;
t4057 = -t1179.*(-t488+t603+dpsi1.*(t105-t465)+dth2.*(t103-t544));
t4061 = t3499.*3.36554e-3;
t4070 = t1179.*(-t488+t603+dpsi1.*(t105-t465)+dth2.*(t103-t544));
t4078 = t241+t242+t243+t508+t510+t512+t577+t580+t583;
t4081 = t251+t252+t253+t507+t509+t511+t576+t579+t582;
t4090 = Mt.*t2087.*t2203;
t4098 = t694+t771+t978+t1094+t1108;
t4141 = Mt.*(t433-t828+T_cg_H.*(t197-t537)).*(t451-t831+T_cg_H.*(t214-t541));
t4142 = Mt.*t2203.*t2360;
t4143 = -t4121;
t4153 = Mt.*t2203.*(-t51+t394+t445-t527+t614);
t4161 = t169+t171+t173+t604+t607+t610+t812+t813+t814;
t4172 = t165+t166+t167+t616+t617+t618+t808+t809+t810;
t4181 = dphi1.*t4167;
t4182 = dz.*t4167;
t4189 = dphi1.*t4163;
t4190 = dy.*t4163;
t4210 = -t4197;
t4218 = Mt.*t1495.*t3531;
t4234 = Mt.*t1618.*t3531;
t4235 = Mt.*t1619.*t3531;
t4236 = Mt.*t1620.*t3531;
t4269 = -Mt.*(t433-t828+T_cg_H.*(t197-t537)).*(-t130+t436+t523-t657+t769);
t4294 = dz.*t4287;
t4295 = dy.*t4288;
t4297 = dy.*t4283;
t4298 = dz.*t4284;
t4323 = Mt.*t2087.*t3531;
t4349 = Mt.*t2360.*t3531;
t4355 = Mt.*t3531.*(-t51+t394+t445-t527+t614);
t4363 = t920+t921+t922+t1110+t1111+t1112;
t4474 = dy.*t4466;
t4475 = dz.*t4466;
t4509 = t356+t358+t360+t997+t998+t999+t1000+t1001+t1002;
t4598 = dth1.*t4593;
t4599 = dth1.*t4594;
t4752 = dth1.*t4743;
t877 = -t823;
t908 = -t878;
t909 = -t879;
t912 = -t883;
t974 = -t929;
t976 = -t930;
t1021 = T_cg_H.*t964;
t1023 = dphi2.*t964;
t1024 = dpsi1.*t964;
t1025 = T_cg_H.*t977;
t1029 = dphi2.*t977;
t1030 = dpsi1.*t977;
t1068 = B_cg_H.*dth2.*t964;
t1132 = -t1070;
t1167 = B_cg_H.*Mb.*t4.*t10.*t964;
t1168 = B_cg_H.*Mb.*t5.*t9.*t964;
t1171 = B_cg_H.*Mb.*t4.*t5.*t977;
t1197 = B_cg_H.*Mb.*t5.*t30.*t964;
t1202 = B_cg_H.*Mb.*t5.*t34.*t964;
t1207 = B_cg_H.*t1180;
t1216 = T_cg_H.*t1178;
t1218 = T_cg_H.*t1180;
t1224 = dphi1.*t1178;
t1226 = dphi1.*t1180;
t1228 = dphi2.*t1178;
t1230 = dpsi1.*t1178;
t1238 = t459+t748;
t1240 = t464+t747;
t1248 = -t1195;
t1266 = dphi1.*t1221;
t1279 = -t1208;
t1289 = -t1219;
t1363 = B_cg_H.*Mb.*t5.*t9.*t1178;
t1383 = -t1352;
t1400 = Mm.*t4.*t5.*t1221;
t1405 = -t1351;
t1406 = Mm.*t9.*t10.*t1221;
t1413 = B_cg_H.*Mb.*t381.*t964;
t1414 = B_cg_H.*Mb.*t382.*t964;
t1421 = B_cg_H.*Mb.*t381.*t977;
t1435 = t11.*t381.*t977;
t1438 = -t1395;
t1440 = -t1396;
t1447 = dphi1.*t1382;
t1462 = dpsi1.*t1394;
t1466 = t1367./2.0;
t1468 = Mm.*t5.*t33.*t1221;
t1471 = Mm.*t5.*t38.*t1221;
t1483 = B_cg_H.*Mb.*t420.*t964;
t1484 = B_cg_H.*Mb.*t421.*t964;
t1487 = B_cg_H.*t1430;
t1494 = T_cg_H.*t1430;
t1496 = B_cg_H.*Mb.*t421.*t977;
t1497 = dphi2.*t1430;
t1498 = dpsi1.*t1430;
t1501 = t487.*t977;
t1503 = -t1425;
t1504 = -t1426;
t1505 = t463+t1039;
t1508 = Mb.*t5.*t1382;
t1516 = -t1464;
t1523 = -t1474;
t1525 = Mb.*t10.*t1362;
t1527 = t1430.^2;
t1528 = t723+t880;
